simulink model "kinovaMicoSimscapeModel"  (R2021b)
(part 40 of 50)

Y4_5_3=(1369*ddqr5)/2000000 - (4107*ddqr4*cos(q5)^2)/4000000 + ddqr4*((23717*3^(1/2))/10000000 + 2327843/400000000) - (1369*dq2*dqr3*sin(2*q5))/4000000 + (1369*dq3*dqr3*sin(2*q5))/4000000 + (4107*dq4*dqr5*sin(2*q5))/8000000 + (4107*dq5*dqr4*sin(2*q5))/8000000 - (32449*ddqr2*sin(q4)*sin(q5))/4000000 + (32449*ddqr3*sin(q4)*sin(q5))/4000000 - ddqr4*cos(q5)*((23717*3^(1/2))/20000000 + 1369/1000000) - ddqr5*cos(q5)*((23717*3^(1/2))/20000000 + 1369/1000000) - ddqr2*cos(q4)*((562157*3^(1/2))/80000000 + 32449/4000000) + ddqr3*cos(q4)*((562157*3^(1/2))/80000000 + 32449/4000000) + (1369*3^(1/2)*ddqr2*cos(q4)*cos(q5)^2)/4000000 - (1369*3^(1/2)*ddqr3*cos(q4)*cos(q5)^2)/4000000 + dq2*dqr3*sin(q5)*((23717*3^(1/2))/20000000 + 1369/1000000) - dq3*dqr3*sin(q5)*((23717*3^(1/2))/20000000 + 1369/1000000) + dq5*dqr5*sin(q5)*((23717*3^(1/2))/20000000 + 1369/1000000) + dq4*dqr5*sin(q5)*((23717*3^(1/2))/40000000 + 1369/2000000) + dq5*dqr4*sin(q5)*((23717*3^(1/2))/40000000 + 1369/2000000) - (1073*ddqr2*cos(q3)*cos(q4)*cos(q5))/200000 - (1073*ddqr1*cos(q4)*sin(q2)*sin(q5))/100000 - (1073*ddqr1*cos(q5)*sin(q2)*sin(q4))/200000 + (1073*ddqr2*cos(q3)*sin(q4)*sin(q5))/100000 + (1369*3^(1/2)*dq2*dqr5*sin(q4))/2000000 - (1369*3^(1/2)*dq3*dqr5*sin(q4))/2000000 - (1369*3^(1/2)*dq5*dqr3*sin(q4))/2000000 + ddqr2*cos(q3)*cos(q4)*((18589*3^(1/2))/2000000 + 1073/100000) - ddqr2*cos(q4)*cos(q5)*((1369*3^(1/2))/2000000 - 45547/20000000) + ddqr3*cos(q4)*cos(q5)*((1369*3^(1/2))/2000000 - 45547/20000000) - (4107*ddqr1*cos(q2)*cos(q3)*cos(q5)^2)/4000000 + ddqr1*cos(q2)*cos(q3)*((23717*3^(1/2))/10000000 + 2327843/400000000) + ddqr1*sin(q2)*sin(q4)*((18589*3^(1/2))/2000000 + 1073/100000) + dq2*dqr3*sin(2*q4)*((23717*3^(1/2))/20000000 + 1232643/800000000) - dq3*dqr3*sin(2*q4)*((23717*3^(1/2))/20000000 + 1232643/800000000) - (4107*ddqr1*cos(q5)^2*sin(q2)*sin(q3))/4000000 + ddqr1*sin(q2)*sin(q3)*((23717*3^(1/2))/10000000 + 2327843/400000000) + dq2*dqr5*cos(q4)*sin(q5)*((1369*3^(1/2))/2000000 + 71151/40000000) - dq3*dqr5*cos(q4)*sin(q5)*((1369*3^(1/2))/2000000 + 71151/40000000) - dq5*dqr3*cos(q4)*sin(q5)*((1369*3^(1/2))/2000000 + 71151/40000000) + (1369*dq2*dqr3*cos(q4)*cos(q5)^2*sin(q4))/800000 + (1369*dq2*dqr3*cos(q4)^2*cos(q5)*sin(q5))/1000000 - (1369*dq3*dqr3*cos(q4)*cos(q5)^2*sin(q4))/800000 - (1369*dq3*dqr3*cos(q4)^2*cos(q5)*sin(q5))/1000000 + (259*ddqr1*cos(q2)*cos(q3)*cos(q4)*cos(q5))/2000000 - (259*ddqr1*cos(q2)*cos(q3)*sin(q4)*sin(q5))/1000000 - (32449*ddqr1*cos(q2)*cos(q4)*sin(q3)*sin(q5))/4000000 + (32449*ddqr1*cos(q3)*cos(q4)*sin(q2)*sin(q5))/4000000 + (259*ddqr1*cos(q4)*cos(q5)*sin(q2)*sin(q3))/2000000 - (259*ddqr1*sin(q2)*sin(q3)*sin(q4)*sin(q5))/1000000 - dq2*dqr3*cos(q4)^2*sin(q5)*((23717*3^(1/2))/10000000 + 1369/500000) + dq3*dqr3*cos(q4)^2*sin(q5)*((23717*3^(1/2))/10000000 + 1369/500000) - ddqr1*cos(q2)*cos(q3)*cos(q4)*((4487*3^(1/2))/20000000 + 259/1000000) - ddqr1*cos(q2)*cos(q3)*cos(q5)*((23717*3^(1/2))/20000000 + 1369/1000000) - ddqr1*cos(q4)*sin(q2)*sin(q3)*((4487*3^(1/2))/20000000 + 259/1000000) - ddqr1*cos(q5)*sin(q2)*sin(q3)*((23717*3^(1/2))/20000000 + 1369/1000000) + ddqr1*cos(q2)*sin(q3)*sin(q4)*((562157*3^(1/2))/80000000 + 32449/4000000) - ddqr1*cos(q3)*sin(q2)*sin(q4)*((562157*3^(1/2))/80000000 + 32449/4000000) - (1369*3^(1/2)*dq2*dqr5*cos(q5)^2*sin(q4))/2000000 + (1369*3^(1/2)*dq3*dqr5*cos(q5)^2*sin(q4))/2000000 + (1369*3^(1/2)*dq5*dqr3*cos(q5)^2*sin(q4))/2000000 - (1369*3^(1/2)*ddqr2*cos(q5)*sin(q4)*sin(q5))/2000000 + (1369*3^(1/2)*ddqr3*cos(q5)*sin(q4)*sin(q5))/2000000 + (1369*3^(1/2)*dq1*dqr5*cos(q2)*cos(q4)*sin(q3))/2000000 - (1369*3^(1/2)*dq1*dqr5*cos(q3)*cos(q4)*sin(q2))/2000000 - (1369*3^(1/2)*dq2*dqr5*cos(q4)*cos(q5)*sin(q5))/4000000 + (1369*3^(1/2)*dq3*dqr5*cos(q4)*cos(q5)*sin(q5))/4000000 + (1369*3^(1/2)*dq5*dqr3*cos(q4)*cos(q5)*sin(q5))/4000000 + ddqr1*cos(q2)*cos(q5)*sin(q3)*sin(q4)*((1369*3^(1/2))/2000000 - 45547/20000000) - ddqr1*cos(q3)*cos(q5)*sin(q2)*sin(q4)*((1369*3^(1/2))/2000000 - 45547/20000000) - (32449*dq1*dqr3*cos(q2)*cos(q3)*cos(q4)*sin(q5))/4000000 + (4107*dq1*dqr5*cos(q2)*cos(q3)*cos(q5)*sin(q5))/4000000 + (4107*dq1*dqr5*cos(q5)*sin(q2)*sin(q3)*sin(q5))/4000000 - dq2*dqr3*cos(q4)*cos(q5)*sin(q4)*((23717*3^(1/2))/20000000 + 1369/1000000) + dq3*dqr3*cos(q4)*cos(q5)*sin(q4)*((23717*3^(1/2))/20000000 + 1369/1000000) + dq1*dqr5*cos(q2)*cos(q3)*sin(q5)*((23717*3^(1/2))/40000000 + 1369/2000000) + dq1*dqr3*cos(q2)*cos(q3)*sin(q4)*((562157*3^(1/2))/80000000 + 32449/4000000) - (1369*3^(1/2)*ddqr1*cos(q2)*cos(q5)^2*sin(q3)*sin(q4))/4000000 + (1369*3^(1/2)*ddqr1*cos(q3)*cos(q5)^2*sin(q2)*sin(q4))/4000000 + dq1*dqr5*sin(q2)*sin(q3)*sin(q5)*((23717*3^(1/2))/40000000 + 1369/2000000) - (1369*3^(1/2)*dq1*dqr5*cos(q2)*cos(q4)*cos(q5)^2*sin(q3))/2000000 + (1369*3^(1/2)*dq1*dqr5*cos(q3)*cos(q4)*cos(q5)^2*sin(q2))/2000000 - (1369*3^(1/2)*ddqr1*cos(q2)*cos(q4)*cos(q5)*sin(q3)*sin(q5))/2000000 + (1369*3^(1/2)*ddqr1*cos(q3)*cos(q4)*cos(q5)*sin(q2)*sin(q5))/2000000 - dq1*dqr5*cos(q2)*sin(q3)*sin(q4)*sin(q5)*((1369*3^(1/2))/2000000 + 71151/40000000) + dq1*dqr5*cos(q3)*sin(q2)*sin(q4)*sin(q5)*((1369*3^(1/2))/2000000 + 71151/40000000) - (1369*3^(1/2)*dq1*dqr3*cos(q2)*cos(q3)*cos(q4)*cos(q5)*sin(q5))/2000000 + (1369*3^(1/2)*dq1*dqr5*cos(q2)*cos(q5)*sin(q3)*sin(q4)*sin(q5))/4000000 - (1369*3^(1/2)*dq1*dqr5*cos(q3)*cos(q5)*sin(q2)*sin(q4)*sin(q5))/4000000;
Y4_8_1=(1231*ddqr2*cos(q4))/10000 - (1231*ddqr3*cos(q4))/10000 + (7*dq1*dqr1*sin(q4))/1000 - (29*ddqr2*cos(q3)*cos(q4))/100 - (29*ddqr1*sin(q2)*sin(q4))/100 + (7*ddqr1*cos(q2)*cos(q3)*cos(q4))/1000 - (1231*ddqr1*cos(q2)*sin(q3)*sin(q4))/10000 + (1231*ddqr1*cos(q3)*sin(q2)*sin(q4))/10000 + (7*ddqr1*cos(q4)*sin(q2)*sin(q3))/1000 + (29*dq1*dqr1*cos(q4)*sin(q3))/100 - (29*dq1*dqr2*cos(q2)*sin(q4))/100 - (29*dq2*dqr1*cos(q2)*sin(q4))/100 + (29*dq2*dqr2*cos(q4)*sin(q3))/100 - (29*dq1*dqr1*cos(q2)^2*cos(q4)*sin(q3))/100 + (1231*dq1*dqr1*cos(q2)*cos(q4)*sin(q2))/10000 - (1231*dq1*dqr1*cos(q3)*cos(q4)*sin(q3))/10000 + (1231*dq1*dqr2*cos(q2)*cos(q3)*sin(q4))/10000 + (1231*dq2*dqr1*cos(q2)*cos(q3)*sin(q4))/10000 - (1231*dq1*dqr3*cos(q2)*cos(q3)*sin(q4))/10000 - (1231*dq3*dqr1*cos(q2)*cos(q3)*sin(q4))/10000 + (1231*dq1*dqr2*sin(q2)*sin(q3)*sin(q4))/10000 + (1231*dq2*dqr1*sin(q2)*sin(q3)*sin(q4))/10000 - (1231*dq1*dqr3*sin(q2)*sin(q3)*sin(q4))/10000 - (1231*dq3*dqr1*sin(q2)*sin(q3)*sin(q4))/10000 + (29*dq1*dqr1*cos(q2)*cos(q3)*cos(q4)*sin(q2))/100 - (1231*dq1*dqr1*cos(q2)*cos(q3)^2*cos(q4)*sin(q2))/5000 + (1231*dq1*dqr1*cos(q2)^2*cos(q3)*cos(q4)*sin(q3))/5000;
Y4_9_1=(37*dq2*dqr2*sin(q5))/1000 - (37*dq2*dqr3*sin(q5))/1000 - (37*dq3*dqr2*sin(q5))/1000 + (37*dq3*dqr3*sin(q5))/1000 - (37*dq4*dqr5*sin(q5))/2000 - (37*dq5*dqr4*sin(q5))/2000 - (37*dq1*dqr1*cos(q2)^2*sin(q5))/1000 - (37*dq1*dqr1*cos(q3)^2*sin(q5))/1000 - (37*dq2*dqr2*cos(q4)^2*sin(q5))/500 + (37*dq2*dqr3*cos(q4)^2*sin(q5))/500 + (37*dq3*dqr2*cos(q4)^2*sin(q5))/500 - (37*dq3*dqr3*cos(q4)^2*sin(q5))/500 - (7*dq1*dqr1*cos(q4)*sin(q5))/1000 - (7*dq1*dqr1*cos(q5)*sin(q4))/2000 - (37*3^(1/2)*dq2*dqr5*cos(q4)*sin(q5))/2000 - (37*3^(1/2)*dq5*dqr2*cos(q4)*sin(q5))/2000 + (37*3^(1/2)*dq3*dqr5*cos(q4)*sin(q5))/2000 + (37*3^(1/2)*dq5*dqr3*cos(q4)*sin(q5))/2000 + (37*dq1*dqr1*cos(q2)^2*cos(q3)^2*sin(q5))/500 + (37*dq1*dqr1*cos(q2)^2*cos(q4)^2*sin(q5))/500 + (37*dq1*dqr1*cos(q3)^2*cos(q4)^2*sin(q5))/500 + (37*dq1*dqr2*cos(q2)*cos(q5)*sin(q3))/1000 - (37*dq1*dqr2*cos(q3)*cos(q5)*sin(q2))/1000 + (37*dq2*dqr1*cos(q2)*cos(q5)*sin(q3))/1000 - (37*dq2*dqr1*cos(q3)*cos(q5)*sin(q2))/1000 - (29*dq1*dqr1*cos(q4)*cos(q5)*sin(q3))/200 + (29*dq1*dqr2*cos(q2)*cos(q4)*sin(q5))/100 + (29*dq1*dqr2*cos(q2)*cos(q5)*sin(q4))/200 - (37*dq1*dqr3*cos(q2)*cos(q5)*sin(q3))/1000 + (37*dq1*dqr3*cos(q3)*cos(q5)*sin(q2))/1000 + (29*dq2*dqr1*cos(q2)*cos(q4)*sin(q5))/100 + (29*dq2*dqr1*cos(q2)*cos(q5)*sin(q4))/200 - (37*dq3*dqr1*cos(q2)*cos(q5)*sin(q3))/1000 + (37*dq3*dqr1*cos(q3)*cos(q5)*sin(q2))/1000 - (37*dq1*dqr5*cos(q2)*cos(q3)*sin(q5))/2000 - (29*dq2*dqr2*cos(q4)*cos(q5)*sin(q3))/200 - (37*dq5*dqr1*cos(q2)*cos(q3)*sin(q5))/2000 - (37*dq2*dqr2*cos(q4)*cos(q5)*sin(q4))/1000 + (37*dq2*dqr3*cos(q4)*cos(q5)*sin(q4))/1000 + (37*dq3*dqr2*cos(q4)*cos(q5)*sin(q4))/1000 - (37*dq3*dqr3*cos(q4)*cos(q5)*sin(q4))/1000 + (29*dq1*dqr1*sin(q3)*sin(q4)*sin(q5))/100 - (37*dq1*dqr5*sin(q2)*sin(q3)*sin(q5))/2000 + (29*dq2*dqr2*sin(q3)*sin(q4)*sin(q5))/100 - (37*dq5*dqr1*sin(q2)*sin(q3)*sin(q5))/2000 - (29*dq1*dqr1*cos(q2)^2*sin(q3)*sin(q4)*sin(q5))/100 - (117*dq1*dqr2*cos(q2)*cos(q3)*cos(q4)*sin(q5))/625 - (117*dq2*dqr1*cos(q2)*cos(q3)*cos(q4)*sin(q5))/625 + (117*dq1*dqr3*cos(q2)*cos(q3)*cos(q4)*sin(q5))/625 + (117*dq3*dqr1*cos(q2)*cos(q3)*cos(q4)*sin(q5))/625 - (37*dq1*dqr1*cos(q2)^2*cos(q3)^2*cos(q4)^2*sin(q5))/250 + (117*dq1*dqr1*cos(q2)*sin(q2)*sin(q4)*sin(q5))/625 - (117*dq1*dqr1*cos(q3)*sin(q3)*sin(q4)*sin(q5))/625 - (117*dq1*dqr2*cos(q4)*sin(q2)*sin(q3)*sin(q5))/625 - (117*dq2*dqr1*cos(q4)*sin(q2)*sin(q3)*sin(q5))/625 + (117*dq1*dqr3*cos(q4)*sin(q2)*sin(q3)*sin(q5))/625 + (117*dq3*dqr1*cos(q4)*sin(q2)*sin(q3)*sin(q5))/625 + (29*dq1*dqr1*cos(q2)^2*cos(q4)*cos(q5)*sin(q3))/200 + (37*dq1*dqr1*cos(q2)^2*cos(q4)*cos(q5)*sin(q4))/1000 - (37*dq1*dqr2*cos(q2)*cos(q4)^2*cos(q5)*sin(q3))/1000 + (37*dq1*dqr2*cos(q3)*cos(q4)^2*cos(q5)*sin(q2))/1000 - (37*dq2*dqr1*cos(q2)*cos(q4)^2*cos(q5)*sin(q3))/1000 + (37*dq2*dqr1*cos(q3)*cos(q4)^2*cos(q5)*sin(q2))/1000 + (37*dq1*dqr1*cos(q3)^2*cos(q4)*cos(q5)*sin(q4))/1000 + (37*dq1*dqr3*cos(q2)*cos(q4)^2*cos(q5)*sin(q3))/1000 - (37*dq1*dqr3*cos(q3)*cos(q4)^2*cos(q5)*sin(q2))/1000 + (37*dq3*dqr1*cos(q2)*cos(q4)^2*cos(q5)*sin(q3))/1000 - (37*dq3*dqr1*cos(q3)*cos(q4)^2*cos(q5)*sin(q2))/1000 + (37*3^(1/2)*dq1*dqr5*cos(q2)*sin(q3)*sin(q4)*sin(q5))/2000 - (37*3^(1/2)*dq1*dqr5*cos(q3)*sin(q2)*sin(q4)*sin(q5))/2000 + (37*3^(1/2)*dq5*dqr1*cos(q2)*sin(q3)*sin(q4)*sin(q5))/2000 - (37*3^(1/2)*dq5*dqr1*cos(q3)*sin(q2)*sin(q4)*sin(q5))/2000 - (37*dq1*dqr1*cos(q2)^2*cos(q3)^2*cos(q4)*cos(q5)*sin(q4))/500 - (29*dq1*dqr1*cos(q2)*cos(q3)*cos(q4)*cos(q5)*sin(q2))/200 + (37*dq1*dqr1*cos(q2)*cos(q3)*sin(q2)*sin(q3)*sin(q5))/500 + (29*dq1*dqr1*cos(q2)*cos(q3)*sin(q2)*sin(q4)*sin(q5))/100 + (37*dq1*dqr2*cos(q2)*cos(q4)*sin(q3)*sin(q4)*sin(q5))/500 - (37*dq1*dqr2*cos(q3)*cos(q4)*sin(q2)*sin(q4)*sin(q5))/500 + (37*dq2*dqr1*cos(q2)*cos(q4)*sin(q3)*sin(q4)*sin(q5))/500 - (37*dq2*dqr1*cos(q3)*cos(q4)*sin(q2)*sin(q4)*sin(q5))/500 - (37*dq1*dqr3*cos(q2)*cos(q4)*sin(q3)*sin(q4)*sin(q5))/500 + (37*dq1*dqr3*cos(q3)*cos(q4)*sin(q2)*sin(q4)*sin(q5))/500 - (37*dq3*dqr1*cos(q2)*cos(q4)*sin(q3)*sin(q4)*sin(q5))/500 + (37*dq3*dqr1*cos(q3)*cos(q4)*sin(q2)*sin(q4)*sin(q5))/500 + dq1*dqr1*cos(q2)*cos(q4)*cos(q5)*sin(q2)*((37*3^(1/2))/2000 - 117/1250) - dq1*dqr1*cos(q3)*cos(q4)*cos(q5)*sin(q3)*((37*3^(1/2))/2000 - 117/1250) + dq1*dqr2*cos(q2)*cos(q3)*cos(q5)*sin(q4)*((37*3^(1/2))/2000 - 117/1250) + dq2*dqr1*cos(q2)*cos(q3)*cos(q5)*sin(q4)*((37*3^(1/2))/2000 - 117/1250) - dq1*dqr3*cos(q2)*cos(q3)*cos(q5)*sin(q4)*((37*3^(1/2))/2000 - 117/1250) - dq3*dqr1*cos(q2)*cos(q3)*cos(q5)*sin(q4)*((37*3^(1/2))/2000 - 117/1250) + dq1*dqr2*cos(q5)*sin(q2)*sin(q3)*sin(q4)*((37*3^(1/2))/2000 - 117/1250) + dq2*dqr1*cos(q5)*sin(q2)*sin(q3)*sin(q4)*((37*3^(1/2))/2000 - 117/1250) - dq1*dqr3*cos(q5)*sin(q2)*sin(q3)*sin(q4)*((37*3^(1/2))/2000 - 117/1250) - dq3*dqr1*cos(q5)*sin(q2)*sin(q3)*sin(q4)*((37*3^(1/2))/2000 - 117/1250) - (234*dq1*dqr1*cos(q2)*cos(q3)^2*sin(q2)*sin(q4)*sin(q5))/625 + (234*dq1*dqr1*cos(q2)^2*cos(q3)*sin(q3)*sin(q4)*sin(q5))/625 - (37*dq1*dqr1*cos(q2)*cos(q3)*cos(q4)^2*sin(q2)*sin(q3)*sin(q5))/250 - dq1*dqr1*cos(q2)*cos(q3)^2*cos(q4)*cos(q5)*sin(q2)*((37*3^(1/2))/1000 - 117/625) + dq1*dqr1*cos(q2)^2*cos(q3)*cos(q4)*cos(q5)*sin(q3)*((37*3^(1/2))/1000 - 117/625) - (37*dq1*dqr1*cos(q2)*cos(q3)*cos(q4)*cos(q5)*sin(q2)*sin(q3)*sin(q4))/500;
Y4_9_2=(37*ddqr4*cos(q5))/1000 + (37*ddqr5*cos(q5))/1000 - (37*dq5*dqr5*sin(q5))/1000 + (117*ddqr2*sin(q4)*sin(q5))/625 - (117*ddqr3*sin(q4)*sin(q5))/625 + (37*ddqr1*cos(q2)*cos(q3)*cos(q5))/1000 + (29*ddqr2*cos(q3)*cos(q4)*cos(q5))/200 + (37*ddqr1*cos(q5)*sin(q2)*sin(q3))/1000 + (29*ddqr1*cos(q4)*sin(q2)*sin(q5))/100 + (29*ddqr1*cos(q5)*sin(q2)*sin(q4))/200 - (29*ddqr2*cos(q3)*sin(q4)*sin(q5))/100 + ddqr2*cos(q4)*cos(q5)*((37*3^(1/2))/2000 - 117/1250) - ddqr3*cos(q4)*cos(q5)*((37*3^(1/2))/2000 - 117/1250) - (7*ddqr1*cos(q2)*cos(q3)*cos(q4)*cos(q5))/2000 + (7*ddqr1*cos(q2)*cos(q3)*sin(q4)*sin(q5))/1000 + (117*ddqr1*cos(q2)*cos(q4)*sin(q3)*sin(q5))/625 - (117*ddqr1*cos(q3)*cos(q4)*sin(q2)*sin(q5))/625 - (7*ddqr1*cos(q4)*cos(q5)*sin(q2)*sin(q3))/2000 + (7*ddqr1*sin(q2)*sin(q3)*sin(q4)*sin(q5))/1000 - ddqr1*cos(q2)*cos(q5)*sin(q3)*sin(q4)*((37*3^(1/2))/2000 - 117/1250) + ddqr1*cos(q3)*cos(q5)*sin(q2)*sin(q4)*((37*3^(1/2))/2000 - 117/1250);
Y4_10_1=(111*dq5*dqr1*cos(q5)^2*sin(q2)*sin(q3)*sin(q6))/2000 - (111*dq5*dqr1*sin(q2)*sin(q3)*sin(q6))/4000 + (111*dq6*dqr1*cos(q5)^2*sin(q2)*sin(q3)*sin(q6))/8000 + dq6*dqr1*sin(q2)*sin(q3)*sin(q6)*((1923*3^(1/2))/80000 + 37/4000) + (37*3^(1/2)*dq1*dqr1*cos(q2)*sin(q2)*sin(q4)*sin(q6))/2000 - (37*3^(1/2)*dq2*dqr1*cos(q4)*sin(q2)*sin(q3)*sin(q6))/2000 + (37*3^(1/2)*dq3*dqr1*cos(q4)*sin(q2)*sin(q3)*sin(q6))/2000 + (37*3^(1/2)*dq5*dqr1*cos(q3)*sin(q2)*sin(q4)*sin(q6))/4000 + (87*dq1*dqr1*cos(q2)*cos(q3)*cos(q4)*cos(q6)*sin(q2))/400 + (1231*dq1*dqr1*cos(q2)*cos(q4)*cos(q5)*cos(q6)*sin(q2))/40000 - (37*dq1*dqr1*cos(q2)*cos(q3)*sin(q2)*sin(q3)*sin(q6))/1000 - (877*dq1*dqr1*cos(q2)*cos(q5)*sin(q2)*sin(q4)*sin(q6))/4000 + (37*dq2*dqr1*cos(q3)*cos(q4)*sin(q2)*sin(q4)*sin(q6))/1000 + (877*dq2*dqr1*cos(q4)*cos(q5)*sin(q2)*sin(q3)*sin(q6))/4000 + (1231*dq2*dqr1*cos(q5)*cos(q6)*sin(q2)*sin(q3)*sin(q4))/40000 - (37*dq3*dqr1*cos(q3)*cos(q4)*sin(q2)*sin(q4)*sin(q6))/1000 + (37*dq2*dqr1*cos(q3)*cos(q5)*sin(q2)*sin(q5)*sin(q6))/2000 - (877*dq3*dqr1*cos(q4)*cos(q5)*sin(q2)*sin(q3)*sin(q6))/4000 - (1231*dq3*dqr1*cos(q5)*cos(q6)*sin(q2)*sin(q3)*sin(q4))/40000 - (37*dq3*dqr1*cos(q3)*cos(q5)*sin(q2)*sin(q5)*sin(q6))/2000 + (111*dq5*dqr1*cos(q5)*cos(q6)*sin(q2)*sin(q3)*sin(q5))/4000 + (111*dq6*dqr1*cos(q5)*cos(q6)*sin(q2)*sin(q3)*sin(q5))/4000 - dq2*dqr1*cos(q3)*sin(q2)*sin(q5)*sin(q6)*((641*3^(1/2))/20000 + 37/1000) + dq3*dqr1*cos(q3)*sin(q2)*sin(q5)*sin(q6)*((641*3^(1/2))/20000 + 37/1000) + dq5*dqr1*cos(q5)*sin(q2)*sin(q3)*sin(q6)*((641*3^(1/2))/40000 + 37/2000) + dq6*dqr1*cos(q6)*sin(q2)*sin(q3)*sin(q5)*((641*3^(1/2))/40000 + 37/2000) + dq2*dqr1*cos(q6)*sin(q2)*sin(q3)*sin(q4)*((37*3^(1/2))/4000 + 7539/40000) - dq3*dqr1*cos(q6)*sin(q2)*sin(q3)*sin(q4)*((37*3^(1/2))/4000 + 7539/40000) - dq6*dqr1*cos(q3)*sin(q2)*sin(q4)*sin(q6)*((37*3^(1/2))/4000 + 1923/80000) + dq5*dqr1*cos(q6)*sin(q2)*sin(q3)*sin(q5)*((641*3^(1/2))/80000 - 37/8000) + dq6*dqr1*cos(q5)*sin(q2)*sin(q3)*sin(q6)*((641*3^(1/2))/80000 - 37/8000) + (37*3^(1/2)*dq1*dqr1*cos(q2)*cos(q4)*cos(q5)^2*cos(q6)*sin(q2))/4000 + (29*dq1*dqr1*cos(q2)*cos(q3)*cos(q4)*cos(q5)*cos(q6)*sin(q2))/400 - (37*3^(1/2)*dq1*dqr1*cos(q2)*cos(q3)^2*sin(q2)*sin(q4)*sin(q6))/1000 - (37*3^(1/2)*dq1*dqr1*cos(q2)*cos(q5)^2*sin(q2)*sin(q4)*sin(q6))/1000 + (37*3^(1/2)*dq2*dqr1*cos(q4)*cos(q5)^2*sin(q2)*sin(q3)*sin(q6))/1000 + (37*3^(1/2)*dq2*dqr1*cos(q5)^2*cos(q6)*sin(q2)*sin(q3)*sin(q4))/4000 - (37*3^(1/2)*dq3*dqr1*cos(q4)*cos(q5)^2*sin(q2)*sin(q3)*sin(q6))/1000 - (37*3^(1/2)*dq3*dqr1*cos(q5)^2*cos(q6)*sin(q2)*sin(q3)*sin(q4))/4000 - (37*3^(1/2)*dq5*dqr1*cos(q3)*cos(q5)^2*sin(q2)*sin(q4)*sin(q6))/2000 - (37*3^(1/2)*dq6*dqr1*cos(q3)*cos(q5)^2*sin(q2)*sin(q4)*sin(q6))/8000 - (29*dq1*dqr1*cos(q2)*cos(q3)*cos(q4)*sin(q2)*sin(q5)*sin(q6))/200 - (29*dq1*dqr1*cos(q2)*cos(q3)*cos(q5)*sin(q2)*sin(q4)*sin(q6))/100 - (29*dq1*dqr1*cos(q2)*cos(q3)*cos(q6)*sin(q2)*sin(q4)*sin(q5))/200 - (1231*dq1*dqr1*cos(q2)*cos(q3)^2*cos(q4)*cos(q5)*cos(q6)*sin(q2))/20000 + dq1*dqr1*cos(q2)*cos(q6)*sin(q2)*sin(q4)*sin(q5)*((37*3^(1/2))/4000 - 877/8000) - dq2*dqr1*cos(q4)*cos(q6)*sin(q2)*sin(q3)*sin(q5)*((37*3^(1/2))/4000 - 877/8000) + dq3*dqr1*cos(q4)*cos(q6)*sin(q2)*sin(q3)*sin(q5)*((37*3^(1/2))/4000 - 877/8000) + dq1*dqr1*cos(q2)*cos(q4)*sin(q2)*sin(q5)*sin(q6)*((37*3^(1/2))/2000 - 1231/20000) + dq5*dqr1*cos(q3)*cos(q5)*sin(q2)*sin(q4)*sin(q6)*((37*3^(1/2))/2000 + 1923/40000) + dq6*dqr1*cos(q3)*cos(q6)*sin(q2)*sin(q4)*sin(q5)*((37*3^(1/2))/2000 + 1923/40000) - dq5*dqr1*cos(q3)*cos(q6)*sin(q2)*sin(q4)*sin(q5)*((37*3^(1/2))/8000 - 1923/80000) + dq6*dqr1*cos(q3)*cos(q5)*sin(q2)*sin(q4)*sin(q6)*((111*3^(1/2))/8000 + 1923/80000) + (37*dq1*dqr1*cos(q2)*cos(q3)*cos(q4)^2*sin(q2)*sin(q3)*sin(q6))/500 + (37*dq1*dqr1*cos(q2)*cos(q3)*cos(q5)^2*sin(q2)*sin(q3)*sin(q6))/500 + (877*dq1*dqr1*cos(q2)*cos(q3)^2*cos(q5)*sin(q2)*sin(q4)*sin(q6))/2000 - (37*dq2*dqr1*cos(q3)*cos(q4)*cos(q5)^2*sin(q2)*sin(q4)*sin(q6))/500 - (37*dq2*dqr1*cos(q3)*cos(q4)^2*cos(q5)*sin(q2)*sin(q5)*sin(q6))/400 + (37*dq3*dqr1*cos(q3)*cos(q4)*cos(q5)^2*sin(q2)*sin(q4)*sin(q6))/500 + (37*dq3*dqr1*cos(q3)*cos(q4)^2*cos(q5)*sin(q2)*sin(q5)*sin(q6))/400 + dq2*dqr1*sin(q2)*sin(q3)*sin(q4)*sin(q5)*sin(q6)*((37*3^(1/2))/2000 - 1231/20000) - dq3*dqr1*sin(q2)*sin(q3)*sin(q4)*sin(q5)*sin(q6)*((37*3^(1/2))/2000 - 1231/20000) - dq1*dqr1*cos(q2)*cos(q3)^2*cos(q4)*cos(q6)*sin(q2)*((37*3^(1/2))/2000 + 7539/20000) + (37*3^(1/2)*dq6*dqr1*cos(q3)*cos(q4)*sin(q2)*sin(q5)*sin(q6))/4000 + dq2*dqr1*cos(q3)*cos(q4)^2*sin(q2)*sin(q5)*sin(q6)*((641*3^(1/2))/20000 + 37/1000) - dq3*dqr1*cos(q3)*cos(q4)^2*sin(q2)*sin(q5)*sin(q6)*((641*3^(1/2))/20000 + 37/1000) + (37*dq1*dqr1*cos(q2)*cos(q3)*cos(q5)*cos(q6)*sin(q2)*sin(q3)*sin(q5))/1000 - (37*dq2*dqr1*cos(q3)*cos(q4)*cos(q5)*cos(q6)*sin(q2)*sin(q4)*sin(q5))/1000 + (37*dq3*dqr1*cos(q3)*cos(q4)*cos(q5)*cos(q6)*sin(q2)*sin(q4)*sin(q5))/1000 - (37*3^(1/2)*dq1*dqr1*cos(q2)*cos(q3)^2*cos(q4)*cos(q5)^2*cos(q6)*sin(q2))/2000 - dq1*dqr1*cos(q2)*cos(q3)*cos(q5)*sin(q2)*sin(q3)*sin(q6)*((641*3^(1/2))/10000 + 37/500) + dq2*dqr1*cos(q3)*cos(q4)*cos(q5)*sin(q2)*sin(q4)*sin(q6)*((641*3^(1/2))/10000 + 37/500) - dq3*dqr1*cos(q3)*cos(q4)*cos(q5)*sin(q2)*sin(q4)*sin(q6)*((641*3^(1/2))/10000 + 37/500) - dq1*dqr1*cos(q2)*cos(q3)*cos(q6)*sin(q2)*sin(q3)*sin(q5)*((641*3^(1/2))/20000 - 37/2000) + dq2*dqr1*cos(q3)*cos(q4)*cos(q6)*sin(q2)*sin(q4)*sin(q5)*((641*3^(1/2))/20000 - 37/2000) - dq3*dqr1*cos(q3)*cos(q4)*cos(q6)*sin(q2)*sin(q4)*sin(q5)*((641*3^(1/2))/20000 - 37/2000) + (37*3^(1/2)*dq1*dqr1*cos(q2)*cos(q3)^2*cos(q5)^2*sin(q2)*sin(q4)*sin(q6))/500 - (37*3^(1/2)*dq1*dqr1*cos(q2)*cos(q4)*cos(q5)*sin(q2)*sin(q5)*sin(q6))/2000 - (37*3^(1/2)*dq1*dqr1*cos(q2)*cos(q5)*cos(q6)*sin(q2)*sin(q4)*sin(q5))/2000 + (37*3^(1/2)*dq2*dqr1*cos(q4)*cos(q5)*cos(q6)*sin(q2)*sin(q3)*sin(q5))/2000 - (37*3^(1/2)*dq3*dqr1*cos(q4)*cos(q5)*cos(q6)*sin(q2)*sin(q3)*sin(q5))/2000 - (37*3^(1/2)*dq5*dqr1*cos(q3)*cos(q4)*cos(q5)*sin(q2)*sin(q5)*sin(q6))/1000 - (37*3^(1/2)*dq5*dqr1*cos(q3)*cos(q5)*cos(q6)*sin(q2)*sin(q4)*sin(q5))/4000 - (37*3^(1/2)*dq6*dqr1*cos(q3)*cos(q4)*cos(q5)*sin(q2)*sin(q5)*sin(q6))/4000 - (37*3^(1/2)*dq6*dqr1*cos(q3)*cos(q5)*cos(q6)*sin(q2)*sin(q4)*sin(q5))/4000 - dq1*dqr1*cos(q2)*cos(q3)^2*cos(q6)*sin(q2)*sin(q4)*sin(q5)*((37*3^(1/2))/2000 - 877/4000) - dq1*dqr1*cos(q2)*cos(q3)^2*cos(q4)*sin(q2)*sin(q5)*sin(q6)*((37*3^(1/2))/1000 - 1231/10000) - (37*3^(1/2)*dq2*dqr1*cos(q5)*sin(q2)*sin(q3)*sin(q4)*sin(q5)*sin(q6))/2000 + (37*3^(1/2)*dq3*dqr1*cos(q5)*sin(q2)*sin(q3)*sin(q4)*sin(q5)*sin(q6))/2000 - (37*dq1*dqr1*cos(q2)*cos(q3)*cos(q4)^2*cos(q5)^2*sin(q2)*sin(q3)*sin(q6))/250 + dq1*dqr1*cos(q2)*cos(q3)*cos(q4)*cos(q6)*sin(q2)*sin(q3)*sin(q4)*((1923*3^(1/2))/20000 + 37/200) - (37*dq1*dqr1*cos(q2)*cos(q3)*cos(q4)*cos(q5)^2*cos(q6)*sin(q2)*sin(q3)*sin(q4))/400 - (37*dq1*dqr1*cos(q2)*cos(q3)*cos(q4)^2*cos(q5)*cos(q6)*sin(q2)*sin(q3)*sin(q5))/500 + dq1*dqr1*cos(q2)*cos(q3)*cos(q4)^2*cos(q5)*sin(q2)*sin(q3)*sin(q6)*((641*3^(1/2))/5000 + 37/250) + dq1*dqr1*cos(q2)*cos(q3)*cos(q4)^2*cos(q6)*sin(q2)*sin(q3)*sin(q5)*((641*3^(1/2))/10000 - 37/1000) + (37*3^(1/2)*dq1*dqr1*cos(q2)*cos(q3)^2*cos(q4)*cos(q5)*sin(q2)*sin(q5)*sin(q6))/1000 + (37*3^(1/2)*dq1*dqr1*cos(q2)*cos(q3)^2*cos(q5)*cos(q6)*sin(q2)*sin(q4)*sin(q5))/1000 + dq1*dqr1*cos(q2)*cos(q3)*cos(q4)*cos(q5)*cos(q6)*sin(q2)*sin(q3)*sin(q4)*((641*3^(1/2))/20000 - 37/2000) - dq1*dqr1*cos(q2)*cos(q3)*cos(q4)*sin(q2)*sin(q3)*sin(q4)*sin(q5)*sin(q6)*((641*3^(1/2))/10000 + 37/500) + (37*dq1*dqr1*cos(q2)*cos(q3)*cos(q4)*cos(q5)*sin(q2)*sin(q3)*sin(q4)*sin(q5)*sin(q6))/200;
Y4_10_2=(87*dq1*dqr1*cos(q4)*cos(q6)*sin(q3))/400 + (29*dq1*dqr1*cos(q4)*cos(q5)*cos(q6)*sin(q3))/400 - (29*dq1*dqr1*cos(q4)*sin(q3)*sin(q5)*sin(q6))/200 - (29*dq1*dqr1*cos(q5)*sin(q3)*sin(q4)*sin(q6))/100 - (29*dq1*dqr1*cos(q6)*sin(q3)*sin(q4)*sin(q5))/200 - dq2*dqr1*cos(q2)*cos(q6)*sin(q3)*((1923*3^(1/2))/40000 + 111/2000) + dq2*dqr1*cos(q3)*cos(q6)*sin(q2)*((1923*3^(1/2))/40000 + 111/2000) + dq3*dqr1*cos(q2)*cos(q6)*sin(q3)*((1923*3^(1/2))/40000 + 111/2000) - dq3*dqr1*cos(q3)*cos(q6)*sin(q2)*((1923*3^(1/2))/40000 + 111/2000) - (87*dq1*dqr1*cos(q2)^2*cos(q4)*cos(q6)*sin(q3))/400 + (37*dq2*dqr1*cos(q2)*cos(q5)^2*cos(q6)*sin(q3))/4000 - (37*dq2*dqr1*cos(q3)*cos(q5)^2*cos(q6)*sin(q2))/4000 - (37*dq3*dqr1*cos(q2)*cos(q5)^2*cos(q6)*sin(q3))/4000 + (37*dq3*dqr1*cos(q3)*cos(q5)^2*cos(q6)*sin(q2))/4000 + dq2*dqr1*cos(q2)*cos(q4)^2*cos(q6)*sin(q3)*((1923*3^(1/2))/40000 + 37/400) - dq2*dqr1*cos(q3)*cos(q4)^2*cos(q6)*sin(q2)*((1923*3^(1/2))/40000 + 37/400) - dq3*dqr1*cos(q2)*cos(q4)^2*cos(q6)*sin(q3)*((1923*3^(1/2))/40000 + 37/400) + dq3*dqr1*cos(q3)*cos(q4)^2*cos(q6)*sin(q2)*((1923*3^(1/2))/40000 + 37/400) - (37*3^(1/2)*dq1*dqr1*cos(q3)*sin(q3)*sin(q4)*sin(q6))/2000 - (37*3^(1/2)*dq5*dqr1*cos(q2)*sin(q3)*sin(q4)*sin(q6))/4000 - (37*dq2*dqr1*cos(q2)*cos(q4)^2*cos(q5)^2*cos(q6)*sin(q3))/800 + (37*dq2*dqr1*cos(q3)*cos(q4)^2*cos(q5)^2*cos(q6)*sin(q2))/800 + (37*dq3*dqr1*cos(q2)*cos(q4)^2*cos(q5)^2*cos(q6)*sin(q3))/800 - (37*dq3*dqr1*cos(q3)*cos(q4)^2*cos(q5)^2*cos(q6)*sin(q2))/800 - (1231*dq1*dqr1*cos(q3)*cos(q4)*cos(q5)*cos(q6)*sin(q3))/40000 - (37*dq2*dqr1*cos(q2)*cos(q4)*sin(q3)*sin(q4)*sin(q6))/1000 + (877*dq1*dqr1*cos(q3)*cos(q5)*sin(q3)*sin(q4)*sin(q6))/4000 + (37*dq3*dqr1*cos(q2)*cos(q4)*sin(q3)*sin(q4)*sin(q6))/1000 - (37*dq2*dqr1*cos(q2)*cos(q5)*sin(q3)*sin(q5)*sin(q6))/2000 + (37*dq3*dqr1*cos(q2)*cos(q5)*sin(q3)*sin(q5)*sin(q6))/2000 - dq2*dqr1*cos(q2)*cos(q5)*cos(q6)*sin(q3)*((641*3^(1/2))/40000 - 37/4000) + dq2*dqr1*cos(q3)*cos(q5)*cos(q6)*sin(q2)*((641*3^(1/2))/40000 - 37/4000) + dq3*dqr1*cos(q2)*cos(q5)*cos(q6)*sin(q3)*((641*3^(1/2))/40000 - 37/4000) - dq3*dqr1*cos(q3)*cos(q5)*cos(q6)*sin(q2)*((641*3^(1/2))/40000 - 37/4000) + dq1*dqr1*cos(q2)*cos(q4)*cos(q6)*sin(q2)*((37*3^(1/2))/4000 + 7539/40000) - dq1*dqr1*cos(q3)*cos(q4)*cos(q6)*sin(q3)*((37*3^(1/2))/4000 + 7539/40000) - (29*dq1*dqr1*cos(q2)^2*cos(q4)*cos(q5)*cos(q6)*sin(q3))/400 + dq2*dqr1*cos(q2)*sin(q3)*sin(q5)*sin(q6)*((641*3^(1/2))/20000 + 37/1000) - dq3*dqr1*cos(q2)*sin(q3)*sin(q5)*sin(q6)*((641*3^(1/2))/20000 + 37/1000) + dq6*dqr1*cos(q2)*sin(q3)*sin(q4)*sin(q6)*((37*3^(1/2))/4000 + 1923/80000) + (29*dq1*dqr1*cos(q2)^2*cos(q4)*sin(q3)*sin(q5)*sin(q6))/200 + (29*dq1*dqr1*cos(q2)^2*cos(q5)*sin(q3)*sin(q4)*sin(q6))/100 + (29*dq1*dqr1*cos(q2)^2*cos(q6)*sin(q3)*sin(q4)*sin(q5))/200 + (37*3^(1/2)*dq5*dqr1*cos(q2)*cos(q4)*cos(q6)*sin(q3))/2000 - (37*3^(1/2)*dq5*dqr1*cos(q3)*cos(q4)*cos(q6)*sin(q2))/2000 + (37*3^(1/2)*dq6*dqr1*cos(q2)*cos(q4)*cos(q6)*sin(q3))/2000 - (37*3^(1/2)*dq6*dqr1*cos(q3)*cos(q4)*cos(q6)*sin(q2))/2000 - (37*3^(1/2)*dq1*dqr1*cos(q3)*cos(q4)*cos(q5)^2*cos(q6)*sin(q3))/4000 - (37*3^(1/2)*dq5*dqr1*cos(q2)*cos(q4)*cos(q5)^2*cos(q6)*sin(q3))/2000 + (37*3^(1/2)*dq5*dqr1*cos(q3)*cos(q4)*cos(q5)^2*cos(q6)*sin(q2))/2000 - (37*3^(1/2)*dq6*dqr1*cos(q2)*cos(q4)*cos(q5)^2*cos(q6)*sin(q3))/2000 + (37*3^(1/2)*dq6*dqr1*cos(q3)*cos(q4)*cos(q5)^2*cos(q6)*sin(q2))/2000 + (37*3^(1/2)*dq1*dqr1*cos(q2)^2*cos(q3)*sin(q3)*sin(q4)*sin(q6))/1000 + (37*3^(1/2)*dq1*dqr1*cos(q3)*cos(q5)^2*sin(q3)*sin(q4)*sin(q6))/1000 + (37*3^(1/2)*dq5*dqr1*cos(q2)*cos(q5)^2*sin(q3)*sin(q4)*sin(q6))/2000 + (37*3^(1/2)*dq6*dqr1*cos(q2)*cos(q5)^2*sin(q3)*sin(q4)*sin(q6))/8000 + (1231*dq1*dqr1*cos(q2)^2*cos(q3)*cos(q4)*cos(q5)*cos(q6)*sin(q3))/20000 - dq1*dqr1*cos(q3)*cos(q6)*sin(q3)*sin(q4)*sin(q5)*((37*3^(1/2))/4000 - 877/8000) - dq1*dqr1*cos(q3)*cos(q4)*sin(q3)*sin(q5)*sin(q6)*((37*3^(1/2))/2000 - 1231/20000) - dq5*dqr1*cos(q2)*cos(q5)*sin(q3)*sin(q4)*sin(q6)*((37*3^(1/2))/2000 + 1923/40000) - dq6*dqr1*cos(q2)*cos(q6)*sin(q3)*sin(q4)*sin(q5)*((37*3^(1/2))/2000 + 1923/40000) + dq5*dqr1*cos(q2)*cos(q6)*sin(q3)*sin(q4)*sin(q5)*((37*3^(1/2))/8000 - 1923/80000) - dq6*dqr1*cos(q2)*cos(q5)*sin(q3)*sin(q4)*sin(q6)*((111*3^(1/2))/8000 + 1923/80000) - (877*dq1*dqr1*cos(q2)^2*cos(q3)*cos(q5)*sin(q3)*sin(q4)*sin(q6))/2000 + (37*dq2*dqr1*cos(q2)*cos(q4)*cos(q5)^2*sin(q3)*sin(q4)*sin(q6))/500 - (37*dq1*dqr1*cos(q2)^2*cos(q4)*cos(q5)*sin(q4)*sin(q5)*sin(q6))/400 + (37*dq2*dqr1*cos(q2)*cos(q4)^2*cos(q5)*sin(q3)*sin(q5)*sin(q6))/400 - (37*dq3*dqr1*cos(q2)*cos(q4)*cos(q5)^2*sin(q3)*sin(q4)*sin(q6))/500 - (37*dq3*dqr1*cos(q2)*cos(q4)^2*cos(q5)*sin(q3)*sin(q5)*sin(q6))/400 + dq1*dqr1*cos(q2)^2*cos(q3)*cos(q4)*cos(q6)*sin(q3)*((37*3^(1/2))/2000 + 7539/20000) + dq2*dqr1*cos(q2)*cos(q4)^2*cos(q5)*cos(q6)*sin(q3)*((641*3^(1/2))/40000 - 37/4000) - dq2*dqr1*cos(q3)*cos(q4)^2*cos(q5)*cos(q6)*sin(q2)*((641*3^(1/2))/40000 - 37/4000) - dq3*dqr1*cos(q2)*cos(q4)^2*cos(q5)*cos(q6)*sin(q3)*((641*3^(1/2))/40000 - 37/4000) + dq3*dqr1*cos(q3)*cos(q4)^2*cos(q5)*cos(q6)*sin(q2)*((641*3^(1/2))/40000 - 37/4000) - (37*3^(1/2)*dq6*dqr1*cos(q2)*cos(q4)*sin(q3)*sin(q5)*sin(q6))/4000 + dq1*dqr1*cos(q2)^2*cos(q4)*sin(q4)*sin(q5)*sin(q6)*((641*3^(1/2))/20000 + 37/1000) - dq2*dqr1*cos(q2)*cos(q4)^2*sin(q3)*sin(q5)*sin(q6)*((641*3^(1/2))/20000 + 37/1000) + dq3*dqr1*cos(q2)*cos(q4)^2*sin(q3)*sin(q5)*sin(q6)*((641*3^(1/2))/20000 + 37/1000) + (37*dq2*dqr1*cos(q2)*cos(q4)*cos(q5)*cos(q6)*sin(q3)*sin(q4)*sin(q5))/1000 - (37*dq3*dqr1*cos(q2)*cos(q4)*cos(q5)*cos(q6)*sin(q3)*sin(q4)*sin(q5))/1000 - dq1*dqr1*cos(q2)^2*cos(q3)^2*cos(q4)*sin(q4)*sin(q5)*sin(q6)*((641*3^(1/2))/10000 + 37/500) + (37*3^(1/2)*dq1*dqr1*cos(q2)^2*cos(q3)*cos(q4)*cos(q5)^2*cos(q6)*sin(q3))/2000 - dq2*dqr1*cos(q2)*cos(q4)*cos(q5)*sin(q3)*sin(q4)*sin(q6)*((641*3^(1/2))/10000 + 37/500) + dq3*dqr1*cos(q2)*cos(q4)*cos(q5)*sin(q3)*sin(q4)*sin(q6)*((641*3^(1/2))/10000 + 37/500) - dq2*dqr1*cos(q2)*cos(q4)*cos(q6)*sin(q3)*sin(q4)*sin(q5)*((641*3^(1/2))/20000 - 37/2000) + dq3*dqr1*cos(q2)*cos(q4)*cos(q6)*sin(q3)*sin(q4)*sin(q5)*((641*3^(1/2))/20000 - 37/2000) - (37*3^(1/2)*dq1*dqr1*cos(q2)^2*cos(q3)*cos(q5)^2*sin(q3)*sin(q4)*sin(q6))/500 + (37*3^(1/2)*dq1*dqr1*cos(q3)*cos(q4)*cos(q5)*sin(q3)*sin(q5)*sin(q6))/2000 + (37*3^(1/2)*dq1*dqr1*cos(q3)*cos(q5)*cos(q6)*sin(q3)*sin(q4)*sin(q5))/2000 - (37*3^(1/2)*dq2*dqr1*cos(q2)*cos(q3)*cos(q5)*sin(q4)*sin(q5)*sin(q6))/2000 + (37*3^(1/2)*dq3*dqr1*cos(q2)*cos(q3)*cos(q5)*sin(q4)*sin(q5)*sin(q6))/2000 + (37*3^(1/2)*dq5*dqr1*cos(q2)*cos(q4)*cos(q5)*sin(q3)*sin(q5)*sin(q6))/1000 + (37*3^(1/2)*dq5*dqr1*cos(q2)*cos(q5)*cos(q6)*sin(q3)*sin(q4)*sin(q5))/4000 + (37*3^(1/2)*dq6*dqr1*cos(q2)*cos(q4)*cos(q5)*sin(q3)*sin(q5)*sin(q6))/4000 + (37*3^(1/2)*dq6*dqr1*cos(q2)*cos(q5)*cos(q6)*sin(q3)*sin(q4)*sin(q5))/4000 + dq1*dqr1*cos(q2)^2*cos(q3)*cos(q6)*sin(q3)*sin(q4)*sin(q5)*((37*3^(1/2))/2000 - 877/4000) + dq1*dqr1*cos(q2)^2*cos(q3)*cos(q4)*sin(q3)*sin(q5)*sin(q6)*((37*3^(1/2))/1000 - 1231/10000) + (37*dq1*dqr1*cos(q2)^2*cos(q3)^2*cos(q4)*cos(q5)*sin(q4)*sin(q5)*sin(q6))/200 - (37*3^(1/2)*dq1*dqr1*cos(q2)^2*cos(q3)*cos(q4)*cos(q5)*sin(q3)*sin(q5)*sin(q6))/1000 - (37*3^(1/2)*dq1*dqr1*cos(q2)^2*cos(q3)*cos(q5)*cos(q6)*sin(q3)*sin(q4)*sin(q5))/1000;
Y4_10_3=(37*dq1*dqr1*cos(q2)^2*sin(q6))/2000 + (37*dq1*dqr1*cos(q3)^2*sin(q6))/2000 + (21*dq1*dqr1*cos(q6)*sin(q4))/4000 - (37*dq1*dqr1*cos(q2)^2*cos(q3)^2*sin(q6))/1000 - (37*dq1*dqr1*cos(q2)^2*cos(q4)^2*sin(q6))/1000 - (37*dq1*dqr1*cos(q2)^2*cos(q5)^2*sin(q6))/1000 - (37*dq1*dqr1*cos(q3)^2*cos(q4)^2*sin(q6))/1000 - (37*dq1*dqr1*cos(q3)^2*cos(q5)^2*sin(q6))/1000 - (87*dq2*dqr1*cos(q2)*cos(q6)*sin(q4))/400 + (7*dq1*dqr1*cos(q4)*cos(q5)*sin(q6))/1000 + (7*dq1*dqr1*cos(q4)*cos(q6)*sin(q5))/2000 + (7*dq1*dqr1*cos(q5)*cos(q6)*sin(q4))/4000 - (111*dq5*dqr1*cos(q2)*cos(q3)*sin(q6))/4000 - (7*dq1*dqr1*sin(q4)*sin(q5)*sin(q6))/2000 + dq1*dqr1*cos(q2)^2*cos(q5)*sin(q6)*((641*3^(1/2))/20000 + 37/1000) + dq1*dqr1*cos(q3)^2*cos(q5)*sin(q6)*((641*3^(1/2))/20000 + 37/1000) + dq1*dqr1*cos(q2)^2*cos(q6)*sin(q5)*((641*3^(1/2))/40000 - 37/4000) + dq1*dqr1*cos(q3)^2*cos(q6)*sin(q5)*((641*3^(1/2))/40000 - 37/4000) - (29*dq2*dqr1*cos(q2)*cos(q4)*cos(q5)*sin(q6))/100 - (29*dq2*dqr1*cos(q2)*cos(q4)*cos(q6)*sin(q5))/200 - (29*dq2*dqr1*cos(q2)*cos(q5)*cos(q6)*sin(q4))/400 + (37*dq1*dqr1*cos(q2)^2*cos(q3)^2*cos(q4)^2*sin(q6))/500 + (37*dq1*dqr1*cos(q2)^2*cos(q3)^2*cos(q5)^2*sin(q6))/500 + (37*dq1*dqr1*cos(q2)^2*cos(q4)^2*cos(q5)^2*sin(q6))/500 + (37*dq1*dqr1*cos(q3)^2*cos(q4)^2*cos(q5)^2*sin(q6))/500 + (29*dq2*dqr1*cos(q2)*sin(q4)*sin(q5)*sin(q6))/200 + dq6*dqr1*cos(q2)*cos(q3)*sin(q6)*((1923*3^(1/2))/80000 + 37/4000) - (37*dq1*dqr1*cos(q2)^2*cos(q5)*cos(q6)*sin(q5))/2000 - (37*dq1*dqr1*cos(q3)^2*cos(q5)*cos(q6)*sin(q5))/2000 + (111*dq5*dqr1*cos(q2)*cos(q3)*cos(q5)^2*sin(q6))/2000 + (111*dq6*dqr1*cos(q2)*cos(q3)*cos(q5)^2*sin(q6))/8000 - dq1*dqr1*cos(q2)^2*cos(q4)*cos(q6)*sin(q4)*((1923*3^(1/2))/40000 + 37/400) - dq1*dqr1*cos(q3)^2*cos(q4)*cos(q6)*sin(q4)*((1923*3^(1/2))/40000 + 37/400) - (37*3^(1/2)*dq1*dqr2*cos(q4)*sin(q2)*sin(q3)*sin(q6))/2000 + (37*dq1*dqr1*cos(q2)^2*cos(q4)*cos(q5)^2*cos(q6)*sin(q4))/800 + (37*dq1*dqr1*cos(q2)^2*cos(q3)^2*cos(q5)*cos(q6)*sin(q5))/1000 + (37*dq1*dqr2*cos(q3)*cos(q4)^2*cos(q5)^2*cos(q6)*sin(q2))/800 + (37*dq1*dqr1*cos(q2)^2*cos(q4)^2*cos(q5)*cos(q6)*sin(q5))/1000 + (37*dq1*dqr1*cos(q3)^2*cos(q4)*cos(q5)^2*cos(q6)*sin(q4))/800 + (37*dq1*dqr1*cos(q3)^2*cos(q4)^2*cos(q5)*cos(q6)*sin(q5))/1000 + (877*dq2*dqr1*cos(q2)*cos(q3)*cos(q4)*cos(q5)*sin(q6))/4000 + (1231*dq2*dqr1*cos(q2)*cos(q3)*cos(q5)*cos(q6)*sin(q4))/40000 - (877*dq3*dqr1*cos(q2)*cos(q3)*cos(q4)*cos(q5)*sin(q6))/4000 - (1231*dq3*dqr1*cos(q2)*cos(q3)*cos(q5)*cos(q6)*sin(q4))/40000 + (111*dq5*dqr1*cos(q2)*cos(q3)*cos(q5)*cos(q6)*sin(q5))/4000 + (111*dq6*dqr1*cos(q2)*cos(q3)*cos(q5)*cos(q6)*sin(q5))/4000 - dq1*dqr1*cos(q2)^2*cos(q3)^2*cos(q5)*sin(q6)*((641*3^(1/2))/10000 + 37/500) - dq1*dqr1*cos(q2)^2*cos(q4)^2*cos(q5)*sin(q6)*((641*3^(1/2))/10000 + 37/500) - dq1*dqr1*cos(q3)^2*cos(q4)^2*cos(q5)*sin(q6)*((641*3^(1/2))/10000 + 37/500) - dq1*dqr1*cos(q2)^2*cos(q3)^2*cos(q6)*sin(q5)*((641*3^(1/2))/20000 - 37/2000) - dq1*dqr1*cos(q2)^2*cos(q4)^2*cos(q6)*sin(q5)*((641*3^(1/2))/20000 - 37/2000) - dq1*dqr1*cos(q3)^2*cos(q4)^2*cos(q6)*sin(q5)*((641*3^(1/2))/20000 - 37/2000) + (37*dq1*dqr2*cos(q3)*cos(q4)*sin(q2)*sin(q4)*sin(q6))/1000 + (877*dq1*dqr2*cos(q4)*cos(q5)*sin(q2)*sin(q3)*sin(q6))/4000 + (1231*dq1*dqr2*cos(q5)*cos(q6)*sin(q2)*sin(q3)*sin(q4))/40000 + (37*dq1*dqr2*cos(q3)*cos(q5)*sin(q2)*sin(q5)*sin(q6))/2000 + dq5*dqr1*cos(q2)*cos(q3)*cos(q5)*sin(q6)*((641*3^(1/2))/40000 + 37/2000) + dq6*dqr1*cos(q2)*cos(q3)*cos(q6)*sin(q5)*((641*3^(1/2))/40000 + 37/2000) + dq2*dqr1*cos(q2)*cos(q3)*cos(q6)*sin(q4)*((37*3^(1/2))/4000 + 7539/40000) - dq3*dqr1*cos(q2)*cos(q3)*cos(q6)*sin(q4)*((37*3^(1/2))/4000 + 7539/40000) + dq5*dqr1*cos(q2)*cos(q3)*cos(q6)*sin(q5)*((641*3^(1/2))/80000 - 37/8000) + dq6*dqr1*cos(q2)*cos(q3)*cos(q5)*sin(q6)*((641*3^(1/2))/80000 - 37/8000) - dq1*dqr2*cos(q3)*sin(q2)*sin(q5)*sin(q6)*((641*3^(1/2))/20000 + 37/1000) + dq1*dqr2*cos(q6)*sin(q2)*sin(q3)*sin(q4)*((37*3^(1/2))/4000 + 7539/40000) - (37*dq1*dqr1*cos(q2)^2*cos(q3)^2*cos(q4)^2*cos(q5)^2*sin(q6))/250 - (37*3^(1/2)*dq2*dqr1*cos(q2)*cos(q3)*cos(q4)*sin(q6))/2000 + (37*3^(1/2)*dq3*dqr1*cos(q2)*cos(q3)*cos(q4)*sin(q6))/2000 + (37*3^(1/2)*dq2*dqr1*cos(q2)*cos(q3)*cos(q4)*cos(q5)^2*sin(q6))/1000 + (37*3^(1/2)*dq2*dqr1*cos(q2)*cos(q3)*cos(q5)^2*cos(q6)*sin(q4))/4000 - (37*3^(1/2)*dq3*dqr1*cos(q2)*cos(q3)*cos(q4)*cos(q5)^2*sin(q6))/1000 - (37*3^(1/2)*dq3*dqr1*cos(q2)*cos(q3)*cos(q5)^2*cos(q6)*sin(q4))/4000 + dq1*dqr1*cos(q2)^2*cos(q3)^2*cos(q4)*cos(q6)*sin(q4)*((1923*3^(1/2))/20000 + 37/200) + (37*3^(1/2)*dq1*dqr2*cos(q4)*cos(q5)^2*sin(q2)*sin(q3)*sin(q6))/1000 + (37*3^(1/2)*dq1*dqr2*cos(q5)^2*cos(q6)*sin(q2)*sin(q3)*sin(q4))/4000 - (37*dq1*dqr1*cos(q2)^2*cos(q3)^2*cos(q4)*cos(q5)^2*cos(q6)*sin(q4))/400 - (37*dq1*dqr1*cos(q2)^2*cos(q3)^2*cos(q4)^2*cos(q5)*cos(q6)*sin(q5))/500 - dq2*dqr1*cos(q2)*cos(q3)*cos(q4)*cos(q6)*sin(q5)*((37*3^(1/2))/4000 - 877/8000) + dq3*dqr1*cos(q2)*cos(q3)*cos(q4)*cos(q6)*sin(q5)*((37*3^(1/2))/4000 - 877/8000) + dq1*dqr1*cos(q2)^2*cos(q3)^2*cos(q4)^2*cos(q5)*sin(q6)*((641*3^(1/2))/5000 + 37/250) + dq1*dqr1*cos(q2)^2*cos(q3)^2*cos(q4)^2*cos(q6)*sin(q5)*((641*3^(1/2))/10000 - 37/1000) - dq1*dqr2*cos(q4)*cos(q6)*sin(q2)*sin(q3)*sin(q5)*((37*3^(1/2))/4000 - 877/8000) + dq2*dqr1*cos(q2)*cos(q3)*sin(q4)*sin(q5)*sin(q6)*((37*3^(1/2))/2000 - 1231/20000) - dq3*dqr1*cos(q2)*cos(q3)*sin(q4)*sin(q5)*sin(q6)*((37*3^(1/2))/2000 - 1231/20000) - (37*dq1*dqr2*cos(q3)*cos(q4)*cos(q5)^2*sin(q2)*sin(q4)*sin(q6))/500 - (37*dq1*dqr2*cos(q3)*cos(q4)^2*cos(q5)*sin(q2)*sin(q5)*sin(q6))/400 - (37*dq1*dqr1*cos(q3)^2*cos(q4)*cos(q5)*sin(q4)*sin(q5)*sin(q6))/400 + dq1*dqr2*sin(q2)*sin(q3)*sin(q4)*sin(q5)*sin(q6)*((37*3^(1/2))/2000 - 1231/20000) - dq1*dqr1*cos(q2)^2*cos(q4)*cos(q5)*cos(q6)*sin(q4)*((641*3^(1/2))/40000 - 37/4000) - dq1*dqr2*cos(q3)*cos(q4)^2*cos(q5)*cos(q6)*sin(q2)*((641*3^(1/2))/40000 - 37/4000) - dq1*dqr1*cos(q3)^2*cos(q4)*cos(q5)*cos(q6)*sin(q4)*((641*3^(1/2))/40000 - 37/4000) + dq1*dqr2*cos(q3)*cos(q4)^2*sin(q2)*sin(q5)*sin(q6)*((641*3^(1/2))/20000 + 37/1000) + dq1*dqr1*cos(q3)^2*cos(q4)*sin(q4)*sin(q5)*sin(q6)*((641*3^(1/2))/20000 + 37/1000) + dq1*dqr1*cos(q2)^2*cos(q3)^2*cos(q4)*cos(q5)*cos(q6)*sin(q4)*((641*3^(1/2))/20000 - 37/2000) - (37*dq1*dqr2*cos(q3)*cos(q4)*cos(q5)*cos(q6)*sin(q2)*sin(q4)*sin(q5))/1000 + dq1*dqr2*cos(q3)*cos(q4)*cos(q5)*sin(q2)*sin(q4)*sin(q6)*((641*3^(1/2))/10000 + 37/500) + dq1*dqr2*cos(q3)*cos(q4)*cos(q6)*sin(q2)*sin(q4)*sin(q5)*((641*3^(1/2))/20000 - 37/2000) + (37*3^(1/2)*dq2*dqr1*cos(q2)*cos(q3)*cos(q4)*cos(q5)*cos(q6)*sin(q5))/2000 - (37*3^(1/2)*dq3*dqr1*cos(q2)*cos(q3)*cos(q4)*cos(q5)*cos(q6)*sin(q5))/2000 + (37*3^(1/2)*dq1*dqr2*cos(q4)*cos(q5)*cos(q6)*sin(q2)*sin(q3)*sin(q5))/2000 - (37*3^(1/2)*dq1*dqr2*cos(q5)*sin(q2)*sin(q3)*sin(q4)*sin(q5)*sin(q6))/2000;
Y4_10_4=(37*dq3*dqr2*sin(q6))/2000 - (37*dq2*dqr2*sin(q6))/2000 + (37*dq2*dqr2*cos(q4)^2*sin(q6))/1000 + (37*dq2*dqr2*cos(q5)^2*sin(q6))/1000 - (37*dq3*dqr2*cos(q4)^2*sin(q6))/1000 - (37*dq3*dqr2*cos(q5)^2*sin(q6))/1000 + (37*3^(1/2)*dq5*dqr2*cos(q4)*sin(q6))/4000 + (37*3^(1/2)*dq5*dqr2*cos(q6)*sin(q4))/2000 + (37*3^(1/2)*dq6*dqr2*cos(q6)*sin(q4))/2000 - (37*dq2*dqr2*cos(q4)^2*cos(q5)^2*sin(q6))/500 + (37*dq3*dqr2*cos(q4)^2*cos(q5)^2*sin(q6))/500 - (87*dq1*dqr2*cos(q2)*cos(q6)*sin(q4))/400 + (87*dq2*dqr2*cos(q4)*cos(q6)*sin(q3))/400 + (37*dq2*dqr2*cos(q5)*cos(q6)*sin(q5))/2000 - (37*dq3*dqr2*cos(q5)*cos(q6)*sin(q5))/2000 - dq2*dqr2*cos(q5)*sin(q6)*((641*3^(1/2))/20000 + 37/1000) + dq3*dqr2*cos(q5)*sin(q6)*((641*3^(1/2))/20000 + 37/1000) - dq2*dqr2*cos(q6)*sin(q5)*((641*3^(1/2))/40000 - 37/4000) + dq3*dqr2*cos(q6)*sin(q5)*((641*3^(1/2))/40000 - 37/4000) - dq6*dqr2*cos(q4)*sin(q6)*((37*3^(1/2))/4000 + 1923/80000) + dq2*dqr2*cos(q4)^2*cos(q5)*sin(q6)*((641*3^(1/2))/10000 + 37/500) - dq3*dqr2*cos(q4)^2*cos(q5)*sin(q6)*((641*3^(1/2))/10000 + 37/500) + dq2*dqr2*cos(q4)^2*cos(q6)*sin(q5)*((641*3^(1/2))/20000 - 37/2000) - dq3*dqr2*cos(q4)^2*cos(q6)*sin(q5)*((641*3^(1/2))/20000 - 37/2000) - (37*3^(1/2)*dq6*dqr2*sin(q4)*sin(q5)*sin(q6))/4000 - (37*3^(1/2)*dq5*dqr2*cos(q4)*cos(q5)^2*sin(q6))/2000 - (37*3^(1/2)*dq5*dqr2*cos(q5)^2*cos(q6)*sin(q4))/2000 - (37*3^(1/2)*dq6*dqr2*cos(q4)*cos(q5)^2*sin(q6))/8000 - (37*3^(1/2)*dq6*dqr2*cos(q5)^2*cos(q6)*sin(q4))/2000 - (29*dq1*dqr2*cos(q2)*cos(q4)*cos(q5)*sin(q6))/100 - (29*dq1*dqr2*cos(q2)*cos(q4)*cos(q6)*sin(q5))/200 - (29*dq1*dqr2*cos(q2)*cos(q5)*cos(q6)*sin(q4))/400 + (29*dq2*dqr2*cos(q4)*cos(q5)*cos(q6)*sin(q3))/400 + (29*dq1*dqr2*cos(q2)*sin(q4)*sin(q5)*sin(q6))/200 - (29*dq2*dqr2*cos(q4)*sin(q3)*sin(q5)*sin(q6))/200 - (29*dq2*dqr2*cos(q5)*sin(q3)*sin(q4)*sin(q6))/100 - (29*dq2*dqr2*cos(q6)*sin(q3)*sin(q4)*sin(q5))/200 + dq2*dqr2*cos(q4)*cos(q6)*sin(q4)*((1923*3^(1/2))/40000 + 37/400) - dq3*dqr2*cos(q4)*cos(q6)*sin(q4)*((1923*3^(1/2))/40000 + 37/400) + dq5*dqr2*cos(q4)*cos(q5)*sin(q6)*((37*3^(1/2))/2000 + 1923/40000) + dq6*dqr2*cos(q4)*cos(q6)*sin(q5)*((37*3^(1/2))/2000 + 1923/40000) - dq1*dqr2*cos(q2)*cos(q6)*sin(q3)*((1923*3^(1/2))/40000 + 111/2000) + dq1*dqr2*cos(q3)*cos(q6)*sin(q2)*((1923*3^(1/2))/40000 + 111/2000) - dq5*dqr2*cos(q4)*cos(q6)*sin(q5)*((37*3^(1/2))/8000 - 1923/80000) + dq6*dqr2*cos(q4)*cos(q5)*sin(q6)*((111*3^(1/2))/8000 + 1923/80000) + (37*dq1*dqr2*cos(q2)*cos(q5)^2*cos(q6)*sin(q3))/4000 - (37*dq1*dqr2*cos(q3)*cos(q5)^2*cos(q6)*sin(q2))/4000 - (37*dq2*dqr2*cos(q4)*cos(q5)^2*cos(q6)*sin(q4))/800 - (37*dq2*dqr2*cos(q4)^2*cos(q5)*cos(q6)*sin(q5))/1000 + (37*dq3*dqr2*cos(q4)*cos(q5)^2*cos(q6)*sin(q4))/800 + (37*dq3*dqr2*cos(q4)^2*cos(q5)*cos(q6)*sin(q5))/1000 + dq1*dqr2*cos(q2)*cos(q4)^2*cos(q6)*sin(q3)*((1923*3^(1/2))/40000 + 37/400) - dq1*dqr2*cos(q3)*cos(q4)^2*cos(q6)*sin(q2)*((1923*3^(1/2))/40000 + 37/400) + (37*3^(1/2)*dq1*dqr3*cos(q4)*sin(q2)*sin(q3)*sin(q6))/2000 + (37*3^(1/2)*dq5*dqr2*cos(q5)*sin(q4)*sin(q5)*sin(q6))/1000 + (37*3^(1/2)*dq6*dqr2*cos(q5)*sin(q4)*sin(q5)*sin(q6))/4000 - (37*dq1*dqr2*cos(q2)*cos(q4)^2*cos(q5)^2*cos(q6)*sin(q3))/800 + (877*dq1*dqr2*cos(q2)*cos(q3)*cos(q4)*cos(q5)*sin(q6))/4000 + (1231*dq1*dqr2*cos(q2)*cos(q3)*cos(q5)*cos(q6)*sin(q4))/40000 - (37*dq1*dqr2*cos(q2)*cos(q4)*sin(q3)*sin(q4)*sin(q6))/1000 - (37*dq1*dqr2*cos(q2)*cos(q5)*sin(q3)*sin(q5)*sin(q6))/2000 - (877*dq1*dqr3*cos(q4)*cos(q5)*sin(q2)*sin(q3)*sin(q6))/4000 - (1231*dq1*dqr3*cos(q5)*cos(q6)*sin(q2)*sin(q3)*sin(q4))/40000 + (37*dq2*dqr2*cos(q4)*cos(q5)*sin(q4)*sin(q5)*sin(q6))/400 - (37*dq3*dqr2*cos(q4)*cos(q5)*sin(q4)*sin(q5)*sin(q6))/400 - dq1*dqr2*cos(q2)*cos(q5)*cos(q6)*sin(q3)*((641*3^(1/2))/40000 - 37/4000) + dq1*dqr2*cos(q3)*cos(q5)*cos(q6)*sin(q2)*((641*3^(1/2))/40000 - 37/4000) + dq2*dqr2*cos(q4)*cos(q5)*cos(q6)*sin(q4)*((641*3^(1/2))/40000 - 37/4000) - dq3*dqr2*cos(q4)*cos(q5)*cos(q6)*sin(q4)*((641*3^(1/2))/40000 - 37/4000) + dq1*dqr2*cos(q2)*cos(q3)*cos(q6)*sin(q4)*((37*3^(1/2))/4000 + 7539/40000) + dq1*dqr2*cos(q2)*sin(q3)*sin(q5)*sin(q6)*((641*3^(1/2))/20000 + 37/1000) - dq2*dqr2*cos(q4)*sin(q4)*sin(q5)*sin(q6)*((641*3^(1/2))/20000 + 37/1000) + dq3*dqr2*cos(q4)*sin(q4)*sin(q5)*sin(q6)*((641*3^(1/2))/20000 + 37/1000) - dq1*dqr3*cos(q6)*sin(q2)*sin(q3)*sin(q4)*((37*3^(1/2))/4000 + 7539/40000) - (37*3^(1/2)*dq1*dqr2*cos(q2)*cos(q3)*cos(q4)*sin(q6))/2000 - (37*3^(1/2)*dq5*dqr2*cos(q4)*cos(q5)*cos(q6)*sin(q5))/4000 - (37*3^(1/2)*dq6*dqr2*cos(q4)*cos(q5)*cos(q6)*sin(q5))/4000 + (37*3^(1/2)*dq1*dqr2*cos(q2)*cos(q3)*cos(q4)*cos(q5)^2*sin(q6))/1000 + (37*3^(1/2)*dq1*dqr2*cos(q2)*cos(q3)*cos(q5)^2*cos(q6)*sin(q4))/4000 - (37*3^(1/2)*dq1*dqr3*cos(q4)*cos(q5)^2*sin(q2)*sin(q3)*sin(q6))/1000 - (37*3^(1/2)*dq1*dqr3*cos(q5)^2*cos(q6)*sin(q2)*sin(q3)*sin(q4))/4000 - dq1*dqr2*cos(q2)*cos(q3)*cos(q4)*cos(q6)*sin(q5)*((37*3^(1/2))/4000 - 877/8000) + dq1*dqr3*cos(q4)*cos(q6)*sin(q2)*sin(q3)*sin(q5)*((37*3^(1/2))/4000 - 877/8000) + dq1*dqr2*cos(q2)*cos(q3)*sin(q4)*sin(q5)*sin(q6)*((37*3^(1/2))/2000 - 1231/20000) + (37*dq1*dqr2*cos(q2)*cos(q4)*cos(q5)^2*sin(q3)*sin(q4)*sin(q6))/500 + (37*dq1*dqr2*cos(q2)*cos(q4)^2*cos(q5)*sin(q3)*sin(q5)*sin(q6))/400 + (37*dq1*dqr3*cos(q3)*cos(q4)*cos(q5)^2*sin(q2)*sin(q4)*sin(q6))/500 - dq1*dqr3*sin(q2)*sin(q3)*sin(q4)*sin(q5)*sin(q6)*((37*3^(1/2))/2000 - 1231/20000) + dq1*dqr2*cos(q2)*cos(q4)^2*cos(q5)*cos(q6)*sin(q3)*((641*3^(1/2))/40000 - 37/4000) - dq1*dqr2*cos(q2)*cos(q4)^2*sin(q3)*sin(q5)*sin(q6)*((641*3^(1/2))/20000 + 37/1000) + (37*dq1*dqr2*cos(q2)*cos(q4)*cos(q5)*cos(q6)*sin(q3)*sin(q4)*sin(q5))/1000 + (37*dq1*dqr3*cos(q3)*cos(q4)*cos(q5)*cos(q6)*sin(q2)*sin(q4)*sin(q5))/1000 - dq1*dqr2*cos(q2)*cos(q4)*cos(q5)*sin(q3)*sin(q4)*sin(q6)*((641*3^(1/2))/10000 + 37/500) - dq1*dqr3*cos(q3)*cos(q4)*cos(q5)*sin(q2)*sin(q4)*sin(q6)*((641*3^(1/2))/10000 + 37/500) - dq1*dqr2*cos(q2)*cos(q4)*cos(q6)*sin(q3)*sin(q4)*sin(q5)*((641*3^(1/2))/20000 - 37/2000) - dq1*dqr3*cos(q3)*cos(q4)*cos(q6)*sin(q2)*sin(q4)*sin(q5)*((641*3^(1/2))/20000 - 37/2000) + (37*3^(1/2)*dq1*dqr2*cos(q2)*cos(q3)*cos(q4)*cos(q5)*cos(q6)*sin(q5))/2000 - (37*3^(1/2)*dq1*dqr2*cos(q2)*cos(q3)*cos(q5)*sin(q4)*sin(q5)*sin(q6))/2000 - (37*3^(1/2)*dq1*dqr3*cos(q4)*cos(q5)*cos(q6)*sin(q2)*sin(q3)*sin(q5))/2000 + (37*3^(1/2)*dq1*dqr3*cos(q5)*sin(q2)*sin(q3)*sin(q4)*sin(q5)*sin(q6))/2000;
Y4_10_5=(37*dq2*dqr3*sin(q6))/2000 - (37*dq3*dqr3*sin(q6))/2000 - (111*dq5*dqr4*sin(q6))/4000 + dq6*dqr4*sin(q6)*((1923*3^(1/2))/80000 + 37/4000) - (37*dq2*dqr3*cos(q4)^2*sin(q6))/1000 - (37*dq2*dqr3*cos(q5)^2*sin(q6))/1000 + (37*dq3*dqr3*cos(q4)^2*sin(q6))/1000 + (37*dq3*dqr3*cos(q5)^2*sin(q6))/1000 + (111*dq5*dqr4*cos(q5)^2*sin(q6))/2000 + (111*dq6*dqr4*cos(q5)^2*sin(q6))/8000 - (37*3^(1/2)*dq5*dqr3*cos(q4)*sin(q6))/4000 - (37*3^(1/2)*dq5*dqr3*cos(q6)*sin(q4))/2000 - (37*3^(1/2)*dq6*dqr3*cos(q6)*sin(q4))/2000 + (37*dq2*dqr3*cos(q4)^2*cos(q5)^2*sin(q6))/500 - (37*dq3*dqr3*cos(q4)^2*cos(q5)^2*sin(q6))/500 - (37*dq2*dqr3*cos(q5)*cos(q6)*sin(q5))/2000 + (37*dq3*dqr3*cos(q5)*cos(q6)*sin(q5))/2000 + (111*dq5*dqr4*cos(q5)*cos(q6)*sin(q5))/4000 + (111*dq6*dqr4*cos(q5)*cos(q6)*sin(q5))/4000 - (111*dq1*dqr5*sin(q2)*sin(q3)*sin(q6))/4000 + dq2*dqr3*cos(q5)*sin(q6)*((641*3^(1/2))/20000 + 37/1000) - dq3*dqr3*cos(q5)*sin(q6)*((641*3^(1/2))/20000 + 37/1000) + dq5*dqr4*cos(q5)*sin(q6)*((641*3^(1/2))/40000 + 37/2000) + dq6*dqr4*cos(q6)*sin(q5)*((641*3^(1/2))/40000 + 37/2000) + dq2*dqr3*cos(q6)*sin(q5)*((641*3^(1/2))/40000 - 37/4000) - dq3*dqr3*cos(q6)*sin(q5)*((641*3^(1/2))/40000 - 37/4000) + dq6*dqr3*cos(q4)*sin(q6)*((37*3^(1/2))/4000 + 1923/80000) + dq5*dqr4*cos(q6)*sin(q5)*((641*3^(1/2))/80000 - 37/8000) + dq6*dqr4*cos(q5)*sin(q6)*((641*3^(1/2))/80000 - 37/8000) + (111*dq1*dqr5*cos(q5)^2*sin(q2)*sin(q3)*sin(q6))/2000 - dq2*dqr3*cos(q4)^2*cos(q5)*sin(q6)*((641*3^(1/2))/10000 + 37/500) + dq3*dqr3*cos(q4)^2*cos(q5)*sin(q6)*((641*3^(1/2))/10000 + 37/500) - dq2*dqr3*cos(q4)^2*cos(q6)*sin(q5)*((641*3^(1/2))/20000 - 37/2000) + dq3*dqr3*cos(q4)^2*cos(q6)*sin(q5)*((641*3^(1/2))/20000 - 37/2000) + (37*3^(1/2)*dq6*dqr3*sin(q4)*sin(q5)*sin(q6))/4000 + (37*3^(1/2)*dq5*dqr3*cos(q4)*cos(q5)^2*sin(q6))/2000 + (37*3^(1/2)*dq5*dqr3*cos(q5)^2*cos(q6)*sin(q4))/2000 + (37*3^(1/2)*dq6*dqr3*cos(q4)*cos(q5)^2*sin(q6))/8000 + (37*3^(1/2)*dq6*dqr3*cos(q5)^2*cos(q6)*sin(q4))/2000 - dq2*dqr3*cos(q4)*cos(q6)*sin(q4)*((1923*3^(1/2))/40000 + 37/400) + dq3*dqr3*cos(q4)*cos(q6)*sin(q4)*((1923*3^(1/2))/40000 + 37/400) - dq5*dqr3*cos(q4)*cos(q5)*sin(q6)*((37*3^(1/2))/2000 + 1923/40000) - dq6*dqr3*cos(q4)*cos(q6)*sin(q5)*((37*3^(1/2))/2000 + 1923/40000) + dq1*dqr3*cos(q2)*cos(q6)*sin(q3)*((1923*3^(1/2))/40000 + 111/2000) - dq1*dqr3*cos(q3)*cos(q6)*sin(q2)*((1923*3^(1/2))/40000 + 111/2000) + dq5*dqr3*cos(q4)*cos(q6)*sin(q5)*((37*3^(1/2))/8000 - 1923/80000) - dq6*dqr3*cos(q4)*cos(q5)*sin(q6)*((111*3^(1/2))/8000 + 1923/80000) - (37*dq1*dqr3*cos(q2)*cos(q5)^2*cos(q6)*sin(q3))/4000 + (37*dq1*dqr3*cos(q3)*cos(q5)^2*cos(q6)*sin(q2))/4000 + (37*dq2*dqr3*cos(q4)*cos(q5)^2*cos(q6)*sin(q4))/800 + (37*dq2*dqr3*cos(q4)^2*cos(q5)*cos(q6)*sin(q5))/1000 - (37*dq3*dqr3*cos(q4)*cos(q5)^2*cos(q6)*sin(q4))/800 - (37*dq3*dqr3*cos(q4)^2*cos(q5)*cos(q6)*sin(q5))/1000 - dq1*dqr3*cos(q2)*cos(q4)^2*cos(q6)*sin(q3)*((1923*3^(1/2))/40000 + 37/400) + dq1*dqr3*cos(q3)*cos(q4)^2*cos(q6)*sin(q2)*((1923*3^(1/2))/40000 + 37/400) - (37*3^(1/2)*dq5*dqr3*cos(q5)*sin(q4)*sin(q5)*sin(q6))/1000 - (37*3^(1/2)*dq6*dqr3*cos(q5)*sin(q4)*sin(q5)*sin(q6))/4000 + (37*dq1*dqr3*cos(q2)*cos(q4)^2*cos(q5)^2*cos(q6)*sin(q3))/800 - (37*dq1*dqr3*cos(q3)*cos(q4)^2*cos(q5)^2*cos(q6)*sin(q2))/800 - (877*dq1*dqr3*cos(q2)*cos(q3)*cos(q4)*cos(q5)*sin(q6))/4000 - (1231*dq1*dqr3*cos(q2)*cos(q3)*cos(q5)*cos(q6)*sin(q4))/40000 + (37*dq1*dqr3*cos(q2)*cos(q4)*sin(q3)*sin(q4)*sin(q6))/1000 - (37*dq1*dqr3*cos(q3)*cos(q4)*sin(q2)*sin(q4)*sin(q6))/1000 + (37*dq1*dqr3*cos(q2)*cos(q5)*sin(q3)*sin(q5)*sin(q6))/2000 - (37*dq1*dqr3*cos(q3)*cos(q5)*sin(q2)*sin(q5)*sin(q6))/2000 + (111*dq1*dqr5*cos(q5)*cos(q6)*sin(q2)*sin(q3)*sin(q5))/4000 - (37*dq2*dqr3*cos(q4)*cos(q5)*sin(q4)*sin(q5)*sin(q6))/400 + (37*dq3*dqr3*cos(q4)*cos(q5)*sin(q4)*sin(q5)*sin(q6))/400 + dq1*dqr3*cos(q2)*cos(q5)*cos(q6)*sin(q3)*((641*3^(1/2))/40000 - 37/4000) - dq1*dqr3*cos(q3)*cos(q5)*cos(q6)*sin(q2)*((641*3^(1/2))/40000 - 37/4000) - dq2*dqr3*cos(q4)*cos(q5)*cos(q6)*sin(q4)*((641*3^(1/2))/40000 - 37/4000) + dq3*dqr3*cos(q4)*cos(q5)*cos(q6)*sin(q4)*((641*3^(1/2))/40000 - 37/4000) - dq1*dqr3*cos(q2)*cos(q3)*cos(q6)*sin(q4)*((37*3^(1/2))/4000 + 7539/40000) - dq1*dqr3*cos(q2)*sin(q3)*sin(q5)*sin(q6)*((641*3^(1/2))/20000 + 37/1000) + dq1*dqr3*cos(q3)*sin(q2)*sin(q5)*sin(q6)*((641*3^(1/2))/20000 + 37/1000) + dq2*dqr3*cos(q4)*sin(q4)*sin(q5)*sin(q6)*((641*3^(1/2))/20000 + 37/1000) - dq3*dqr3*cos(q4)*sin(q4)*sin(q5)*sin(q6)*((641*3^(1/2))/20000 + 37/1000) + dq1*dqr5*cos(q5)*sin(q2)*sin(q3)*sin(q6)*((641*3^(1/2))/40000 + 37/2000) + dq1*dqr5*cos(q6)*sin(q2)*sin(q3)*sin(q5)*((641*3^(1/2))/80000 - 37/8000) + (37*3^(1/2)*dq1*dqr3*cos(q2)*cos(q3)*cos(q4)*sin(q6))/2000 + (37*3^(1/2)*dq5*dqr3*cos(q4)*cos(q5)*cos(q6)*sin(q5))/4000 + (37*3^(1/2)*dq6*dqr3*cos(q4)*cos(q5)*cos(q6)*sin(q5))/4000 - (37*3^(1/2)*dq1*dqr3*cos(q2)*cos(q3)*cos(q4)*cos(q5)^2*sin(q6))/1000 - (37*3^(1/2)*dq1*dqr3*cos(q2)*cos(q3)*cos(q5)^2*cos(q6)*sin(q4))/4000 + dq1*dqr3*cos(q2)*cos(q3)*cos(q4)*cos(q6)*sin(q5)*((37*3^(1/2))/4000 - 877/8000) - dq1*dqr3*cos(q2)*cos(q3)*sin(q4)*sin(q5)*sin(q6)*((37*3^(1/2))/2000 - 1231/20000) - dq1*dqr5*cos(q3)*cos(q6)*sin(q2)*sin(q4)*sin(q5)*((37*3^(1/2))/8000 - 1923/80000) - (37*dq1*dqr3*cos(q2)*cos(q4)*cos(q5)^2*sin(q3)*sin(q4)*sin(q6))/500 - (37*dq1*dqr3*cos(q2)*cos(q4)^2*cos(q5)*sin(q3)*sin(q5)*sin(q6))/400 + (37*dq1*dqr3*cos(q3)*cos(q4)^2*cos(q5)*sin(q2)*sin(q5)*sin(q6))/400 - dq1*dqr3*cos(q2)*cos(q4)^2*cos(q5)*cos(q6)*sin(q3)*((641*3^(1/2))/40000 - 37/4000) + dq1*dqr3*cos(q3)*cos(q4)^2*cos(q5)*cos(q6)*sin(q2)*((641*3^(1/2))/40000 - 37/4000) + dq1*dqr3*cos(q2)*cos(q4)^2*sin(q3)*sin(q5)*sin(q6)*((641*3^(1/2))/20000 + 37/1000) - dq1*dqr3*cos(q3)*cos(q4)^2*sin(q2)*sin(q5)*sin(q6)*((641*3^(1/2))/20000 + 37/1000) - (37*dq1*dqr3*cos(q2)*cos(q4)*cos(q5)*cos(q6)*sin(q3)*sin(q4)*sin(q5))/1000 + dq1*dqr3*cos(q2)*cos(q4)*cos(q5)*sin(q3)*sin(q4)*sin(q6)*((641*3^(1/2))/10000 + 37/500) + dq1*dqr3*cos(q2)*cos(q4)*cos(q6)*sin(q3)*sin(q4)*sin(q5)*((641*3^(1/2))/20000 - 37/2000) - (37*3^(1/2)*dq1*dqr3*cos(q2)*cos(q3)*cos(q4)*cos(q5)*cos(q6)*sin(q5))/2000 + (37*3^(1/2)*dq1*dqr3*cos(q2)*cos(q3)*cos(q5)*sin(q4)*sin(q5)*sin(q6))/2000 - (37*3^(1/2)*dq1*dqr5*cos(q3)*cos(q5)*cos(q6)*sin(q2)*sin(q4)*sin(q5))/4000;
Y4_10_6=dq4*dqr6*sin(q6)*((1923*3^(1/2))/80000 + 37/4000) - (37*dq6*dqr5*sin(q6))/4000 - (111*dq4*dqr5*sin(q6))/4000 + (111*dq4*dqr5*cos(q5)^2*sin(q6))/2000 + (111*dq4*dqr6*cos(q5)^2*sin(q6))/8000 + (37*3^(1/2)*dq2*dqr5*cos(q4)*sin(q6))/4000 + (37*3^(1/2)*dq2*dqr5*cos(q6)*sin(q4))/2000 + (37*3^(1/2)*dq2*dqr6*cos(q6)*sin(q4))/2000 - (37*3^(1/2)*dq3*dqr5*cos(q4)*sin(q6))/4000 - (37*3^(1/2)*dq3*dqr5*cos(q6)*sin(q4))/2000 - (37*3^(1/2)*dq3*dqr6*cos(q6)*sin(q4))/2000 - (111*dq1*dqr5*cos(q2)*cos(q3)*sin(q6))/4000 + (111*dq4*dqr5*cos(q5)*cos(q6)*sin(q5))/4000 + (111*dq4*dqr6*cos(q5)*cos(q6)*sin(q5))/4000 + dq5*dqr5*cos(q5)*sin(q6)*((641*3^(1/2))/20000 + 37/1000) + dq5*dqr6*cos(q6)*sin(q5)*((641*3^(1/2))/20000 + 37/1000) + dq6*dqr5*cos(q6)*sin(q5)*((641*3^(1/2))/20000 + 37/1000) + dq6*dqr6*cos(q5)*sin(q6)*((641*3^(1/2))/20000 + 37/1000) + dq6*dqr6*cos(q6)*sin(q5)*((641*3^(1/2))/40000 + 37/800) + dq4*dqr5*cos(q5)*sin(q6)*((641*3^(1/2))/40000 + 37/2000) + dq4*dqr6*cos(q6)*sin(q5)*((641*3^(1/2))/40000 + 37/2000) + dq5*dqr6*cos(q5)*sin(q6)*((641*3^(1/2))/40000 + 37/2000) + dq6*dqr5*cos(q5)*sin(q6)*((641*3^(1/2))/40000 + 37/2000) + dq5*dqr5*cos(q6)*sin(q5)*((641*3^(1/2))/40000 - 37/4000) - dq2*dqr6*cos(q4)*sin(q6)*((37*3^(1/2))/4000 + 1923/80000) + dq3*dqr6*cos(q4)*sin(q6)*((37*3^(1/2))/4000 + 1923/80000) + dq4*dqr5*cos(q6)*sin(q5)*((641*3^(1/2))/80000 - 37/8000) + dq4*dqr6*cos(q5)*sin(q6)*((641*3^(1/2))/80000 - 37/8000) + (111*dq1*dqr6*cos(q5)^2*sin(q2)*sin(q3)*sin(q6))/8000 - (37*3^(1/2)*dq2*dqr6*sin(q4)*sin(q5)*sin(q6))/4000 + (37*3^(1/2)*dq3*dqr6*sin(q4)*sin(q5)*sin(q6))/4000 - (37*3^(1/2)*dq2*dqr5*cos(q4)*cos(q5)^2*sin(q6))/2000 - (37*3^(1/2)*dq2*dqr5*cos(q5)^2*cos(q6)*sin(q4))/2000 - (37*3^(1/2)*dq2*dqr6*cos(q4)*cos(q5)^2*sin(q6))/8000 - (37*3^(1/2)*dq2*dqr6*cos(q5)^2*cos(q6)*sin(q4))/2000 + (37*3^(1/2)*dq3*dqr5*cos(q4)*cos(q5)^2*sin(q6))/2000 + (37*3^(1/2)*dq3*dqr5*cos(q5)^2*cos(q6)*sin(q4))/2000 + (37*3^(1/2)*dq3*dqr6*cos(q4)*cos(q5)^2*sin(q6))/8000 + (37*3^(1/2)*dq3*dqr6*cos(q5)^2*cos(q6)*sin(q4))/2000 + dq2*dqr5*cos(q4)*cos(q5)*sin(q6)*((37*3^(1/2))/2000 + 1923/40000) + dq2*dqr6*cos(q4)*cos(q6)*sin(q5)*((37*3^(1/2))/2000 + 1923/40000) - dq3*dqr5*cos(q4)*cos(q5)*sin(q6)*((37*3^(1/2))/2000 + 1923/40000) - dq3*dqr6*cos(q4)*cos(q6)*sin(q5)*((37*3^(1/2))/2000 + 1923/40000) + dq1*dqr6*cos(q2)*cos(q3)*sin(q6)*((1923*3^(1/2))/80000 + 37/4000) - dq2*dqr5*cos(q4)*cos(q6)*sin(q5)*((37*3^(1/2))/8000 - 1923/80000) + dq3*dqr5*cos(q4)*cos(q6)*sin(q5)*((37*3^(1/2))/8000 - 1923/80000) + dq2*dqr6*cos(q4)*cos(q5)*sin(q6)*((111*3^(1/2))/8000 + 1923/80000) - dq3*dqr6*cos(q4)*cos(q5)*sin(q6)*((111*3^(1/2))/8000 + 1923/80000) + (111*dq1*dqr5*cos(q2)*cos(q3)*cos(q5)^2*sin(q6))/2000 + (111*dq1*dqr6*cos(q2)*cos(q3)*cos(q5)^2*sin(q6))/8000 + dq1*dqr6*sin(q2)*sin(q3)*sin(q6)*((1923*3^(1/2))/80000 + 37/4000) - (37*3^(1/2)*dq1*dqr5*cos(q2)*sin(q3)*sin(q4)*sin(q6))/4000 + (37*3^(1/2)*dq1*dqr5*cos(q3)*sin(q2)*sin(q4)*sin(q6))/4000 + (37*3^(1/2)*dq2*dqr5*cos(q5)*sin(q4)*sin(q5)*sin(q6))/1000 + (37*3^(1/2)*dq2*dqr6*cos(q5)*sin(q4)*sin(q5)*sin(q6))/4000 - (37*3^(1/2)*dq3*dqr5*cos(q5)*sin(q4)*sin(q5)*sin(q6))/1000 - (37*3^(1/2)*dq3*dqr6*cos(q5)*sin(q4)*sin(q5)*sin(q6))/4000 + (111*dq1*dqr5*cos(q2)*cos(q3)*cos(q5)*cos(q6)*sin(q5))/4000 + (111*dq1*dqr6*cos(q2)*cos(q3)*cos(q5)*cos(q6)*sin(q5))/4000 + (111*dq1*dqr6*cos(q5)*cos(q6)*sin(q2)*sin(q3)*sin(q5))/4000 + dq1*dqr5*cos(q2)*cos(q3)*cos(q5)*sin(q6)*((641*3^(1/2))/40000 + 37/2000) + dq1*dqr6*cos(q2)*cos(q3)*cos(q6)*sin(q5)*((641*3^(1/2))/40000 + 37/2000) + dq1*dqr5*cos(q2)*cos(q3)*cos(q6)*sin(q5)*((641*3^(1/2))/80000 - 37/8000) + dq1*dqr6*cos(q2)*cos(q3)*cos(q5)*sin(q6)*((641*3^(1/2))/80000 - 37/8000) + dq1*dqr6*cos(q6)*sin(q2)*sin(q3)*sin(q5)*((641*3^(1/2))/40000 + 37/2000) + dq1*dqr6*cos(q2)*sin(q3)*sin(q4)*sin(q6)*((37*3^(1/2))/4000 + 1923/80000) - dq1*dqr6*cos(q3)*sin(q2)*sin(q4)*sin(q6)*((37*3^(1/2))/4000 + 1923/80000) + dq1*dqr6*cos(q5)*sin(q2)*sin(q3)*sin(q6)*((641*3^(1/2))/80000 - 37/8000) + (37*3^(1/2)*dq1*dqr5*cos(q2)*cos(q4)*cos(q6)*sin(q3))/2000 - (37*3^(1/2)*dq1*dqr5*cos(q3)*cos(q4)*cos(q6)*sin(q2))/2000 + (37*3^(1/2)*dq1*dqr6*cos(q2)*cos(q4)*cos(q6)*sin(q3))/2000 - (37*3^(1/2)*dq1*dqr6*cos(q3)*cos(q4)*cos(q6)*sin(q2))/2000 - (37*3^(1/2)*dq2*dqr5*cos(q4)*cos(q5)*cos(q6)*sin(q5))/4000 - (37*3^(1/2)*dq2*dqr6*cos(q4)*cos(q5)*cos(q6)*sin(q5))/4000 + (37*3^(1/2)*dq3*dqr5*cos(q4)*cos(q5)*cos(q6)*sin(q5))/4000 + (37*3^(1/2)*dq3*dqr6*cos(q4)*cos(q5)*cos(q6)*sin(q5))/4000 - (37*3^(1/2)*dq1*dqr5*cos(q2)*cos(q4)*cos(q5)^2*cos(q6)*sin(q3))/2000 + (37*3^(1/2)*dq1*dqr5*cos(q3)*cos(q4)*cos(q5)^2*cos(q6)*sin(q2))/2000 - (37*3^(1/2)*dq1*dqr6*cos(q2)*cos(q4)*cos(q5)^2*cos(q6)*sin(q3))/2000 + (37*3^(1/2)*dq1*dqr6*cos(q3)*cos(q4)*cos(q5)^2*cos(q6)*sin(q2))/2000 + (37*3^(1/2)*dq1*dqr5*cos(q2)*cos(q5)^2*sin(q3)*sin(q4)*sin(q6))/2000 - (37*3^(1/2)*dq1*dqr5*cos(q3)*cos(q5)^2*sin(q2)*sin(q4)*sin(q6))/2000 + (37*3^(1/2)*dq1*dqr6*cos(q2)*cos(q5)^2*sin(q3)*sin(q4)*sin(q6))/8000 - (37*3^(1/2)*dq1*dqr6*cos(q3)*cos(q5)^2*sin(q2)*sin(q4)*sin(q6))/8000 - dq1*dqr5*cos(q2)*cos(q5)*sin(q3)*sin(q4)*sin(q6)*((37*3^(1/2))/2000 + 1923/40000) + dq1*dqr5*cos(q3)*cos(q5)*sin(q2)*sin(q4)*sin(q6)*((37*3^(1/2))/2000 + 1923/40000) - dq1*dqr6*cos(q2)*cos(q6)*sin(q3)*sin(q4)*sin(q5)*((37*3^(1/2))/2000 + 1923/40000) + dq1*dqr6*cos(q3)*cos(q6)*sin(q2)*sin(q4)*sin(q5)*((37*3^(1/2))/2000 + 1923/40000) + dq1*dqr5*cos(q2)*cos(q6)*sin(q3)*sin(q4)*sin(q5)*((37*3^(1/2))/8000 - 1923/80000) - dq1*dqr6*cos(q2)*cos(q5)*sin(q3)*sin(q4)*sin(q6)*((111*3^(1/2))/8000 + 1923/80000) + dq1*dqr6*cos(q3)*cos(q5)*sin(q2)*sin(q4)*sin(q6)*((111*3^(1/2))/8000 + 1923/80000) - (37*3^(1/2)*dq1*dqr6*cos(q2)*cos(q4)*sin(q3)*sin(q5)*sin(q6))/4000 + (37*3^(1/2)*dq1*dqr6*cos(q3)*cos(q4)*sin(q2)*sin(q5)*sin(q6))/4000 + (37*3^(1/2)*dq1*dqr5*cos(q2)*cos(q4)*cos(q5)*sin(q3)*sin(q5)*sin(q6))/1000 + (37*3^(1/2)*dq1*dqr5*cos(q2)*cos(q5)*cos(q6)*sin(q3)*sin(q4)*sin(q5))/4000 - (37*3^(1/2)*dq1*dqr5*cos(q3)*cos(q4)*cos(q5)*sin(q2)*sin(q5)*sin(q6))/1000 + (37*3^(1/2)*dq1*dqr6*cos(q2)*cos(q4)*cos(q5)*sin(q3)*sin(q5)*sin(q6))/4000 + (37*3^(1/2)*dq1*dqr6*cos(q2)*cos(q5)*cos(q6)*sin(q3)*sin(q4)*sin(q5))/4000 - (37*3^(1/2)*dq1*dqr6*cos(q3)*cos(q4)*cos(q5)*sin(q2)*sin(q5)*sin(q6))/4000 - (37*3^(1/2)*dq1*dqr6*cos(q3)*cos(q5)*cos(q6)*sin(q2)*sin(q4)*sin(q5))/4000;
Y4_10_7=(37*ddqr5*cos(q6))/2000 + (37*ddqr6*cos(q6))/2000 - (37*dq5*dqr6*sin(q6))/4000 - (37*dq6*dqr6*sin(q6))/2000 - ddqr4*cos(q6)*((1923*3^(1/2))/40000 + 37/2000) - (111*ddqr4*cos(q5)^2*cos(q6))/4000 - (87*ddqr2*cos(q3)*cos(q4)*cos(q6))/400 + (1231*ddqr2*cos(q4)*cos(q5)*cos(q6))/40000 - (1231*ddqr3*cos(q4)*cos(q5)*cos(q6))/40000 - (87*ddqr1*cos(q6)*sin(q2)*sin(q4))/400 - (877*ddqr2*cos(q5)*sin(q4)*sin(q6))/4000 + (877*ddqr3*cos(q5)*sin(q4)*sin(q6))/4000 + (111*ddqr4*cos(q5)*sin(q5)*sin(q6))/2000 - ddqr6*cos(q5)*cos(q6)*((641*3^(1/2))/20000 + 37/1000) - ddqr4*cos(q5)*cos(q6)*((641*3^(1/2))/40000 - 37/4000) - ddqr5*cos(q5)*cos(q6)*((641*3^(1/2))/40000 - 37/4000) + ddqr2*cos(q4)*cos(q6)*((37*3^(1/2))/4000 + 7539/40000) - ddqr3*cos(q4)*cos(q6)*((37*3^(1/2))/4000 + 7539/40000) + ddqr4*sin(q5)*sin(q6)*((641*3^(1/2))/20000 + 37/1000) + ddqr5*sin(q5)*sin(q6)*((641*3^(1/2))/20000 + 37/1000) + ddqr6*sin(q5)*sin(q6)*((641*3^(1/2))/40000 + 37/800) + (37*3^(1/2)*ddqr2*sin(q4)*sin(q6))/2000 - (37*3^(1/2)*ddqr3*sin(q4)*sin(q6))/2000 + (37*3^(1/2)*ddqr2*cos(q4)*cos(q5)^2*cos(q6))/4000 - (37*3^(1/2)*ddqr3*cos(q4)*cos(q5)^2*cos(q6))/4000 + (21*ddqr1*cos(q2)*cos(q3)*cos(q4)*cos(q6))/4000 - (29*ddqr2*cos(q3)*cos(q4)*cos(q5)*cos(q6))/400 - (37*3^(1/2)*ddqr2*cos(q5)^2*sin(q4)*sin(q6))/1000 + (37*3^(1/2)*ddqr3*cos(q5)^2*sin(q4)*sin(q6))/1000 + (21*ddqr1*cos(q4)*cos(q6)*sin(q2)*sin(q3))/4000 - (29*ddqr1*cos(q4)*cos(q5)*sin(q2)*sin(q6))/100 - (29*ddqr1*cos(q4)*cos(q6)*sin(q2)*sin(q5))/200 - (29*ddqr1*cos(q5)*cos(q6)*sin(q2)*sin(q4))/400 + (29*ddqr2*cos(q3)*cos(q4)*sin(q5)*sin(q6))/200 + (29*ddqr2*cos(q3)*cos(q5)*sin(q4)*sin(q6))/100 + (29*ddqr2*cos(q3)*cos(q6)*sin(q4)*sin(q5))/200 + (29*ddqr1*sin(q2)*sin(q4)*sin(q5)*sin(q6))/200 - ddqr1*cos(q2)*cos(q3)*cos(q6)*((1923*3^(1/2))/40000 + 37/2000) - (111*ddqr1*cos(q2)*cos(q3)*cos(q5)^2*cos(q6))/4000 + ddqr2*cos(q6)*sin(q4)*sin(q5)*((37*3^(1/2))/4000 - 877/8000) - ddqr3*cos(q6)*sin(q4)*sin(q5)*((37*3^(1/2))/4000 - 877/8000) + ddqr2*cos(q4)*sin(q5)*sin(q6)*((37*3^(1/2))/2000 - 1231/20000) - ddqr3*cos(q4)*sin(q5)*sin(q6)*((37*3^(1/2))/2000 - 1231/20000) - ddqr1*cos(q6)*sin(q2)*sin(q3)*((1923*3^(1/2))/40000 + 37/2000) - (111*ddqr1*cos(q5)^2*cos(q6)*sin(q2)*sin(q3))/4000 - (7*ddqr1*cos(q2)*cos(q3)*cos(q4)*sin(q5)*sin(q6))/2000 - (7*ddqr1*cos(q2)*cos(q3)*cos(q5)*sin(q4)*sin(q6))/1000 - (7*ddqr1*cos(q2)*cos(q3)*cos(q6)*sin(q4)*sin(q5))/2000 - (877*ddqr1*cos(q2)*cos(q4)*cos(q5)*sin(q3)*sin(q6))/4000 - (1231*ddqr1*cos(q2)*cos(q5)*cos(q6)*sin(q3)*sin(q4))/40000 + (877*ddqr1*cos(q3)*cos(q4)*cos(q5)*sin(q2)*sin(q6))/4000 + (1231*ddqr1*cos(q3)*cos(q5)*cos(q6)*sin(q2)*sin(q4))/40000 + (7*ddqr1*cos(q4)*cos(q5)*cos(q6)*sin(q2)*sin(q3))/4000 + (111*ddqr1*cos(q2)*cos(q3)*cos(q5)*sin(q5)*sin(q6))/2000 - (7*ddqr1*cos(q4)*sin(q2)*sin(q3)*sin(q5)*sin(q6))/2000 - (7*ddqr1*cos(q5)*sin(q2)*sin(q3)*sin(q4)*sin(q6))/1000 - (7*ddqr1*cos(q6)*sin(q2)*sin(q3)*sin(q4)*sin(q5))/2000 + (111*ddqr1*cos(q5)*sin(q2)*sin(q3)*sin(q5)*sin(q6))/2000 - ddqr1*cos(q2)*cos(q3)*cos(q5)*cos(q6)*((641*3^(1/2))/40000 - 37/4000) + ddqr1*cos(q2)*cos(q3)*sin(q5)*sin(q6)*((641*3^(1/2))/20000 + 37/1000) - ddqr1*cos(q5)*cos(q6)*sin(q2)*sin(q3)*((641*3^(1/2))/40000 - 37/4000) - ddqr1*cos(q2)*cos(q6)*sin(q3)*sin(q4)*((37*3^(1/2))/4000 + 7539/40000) + ddqr1*cos(q3)*cos(q6)*sin(q2)*sin(q4)*((37*3^(1/2))/4000 + 7539/40000) + ddqr1*sin(q2)*sin(q3)*sin(q5)*sin(q6)*((641*3^(1/2))/20000 + 37/1000) + (37*3^(1/2)*ddqr1*cos(q2)*cos(q4)*sin(q3)*sin(q6))/2000 - (37*3^(1/2)*ddqr1*cos(q3)*cos(q4)*sin(q2)*sin(q6))/2000 - (37*3^(1/2)*ddqr2*cos(q4)*cos(q5)*sin(q5)*sin(q6))/2000 - (37*3^(1/2)*ddqr2*cos(q5)*cos(q6)*sin(q4)*sin(q5))/2000 + (37*3^(1/2)*ddqr3*cos(q4)*cos(q5)*sin(q5)*sin(q6))/2000 + (37*3^(1/2)*ddqr3*cos(q5)*cos(q6)*sin(q4)*sin(q5))/2000 + (7*ddqr1*cos(q2)*cos(q3)*cos(q4)*cos(q5)*cos(q6))/4000 + ddqr1*cos(q2)*cos(q4)*cos(q6)*sin(q3)*sin(q5)*((37*3^(1/2))/4000 - 877/8000) - ddqr1*cos(q3)*cos(q4)*cos(q6)*sin(q2)*sin(q5)*((37*3^(1/2))/4000 - 877/8000) - ddqr1*cos(q2)*sin(q3)*sin(q4)*sin(q5)*sin(q6)*((37*3^(1/2))/2000 - 1231/20000) + ddqr1*cos(q3)*sin(q2)*sin(q4)*sin(q5)*sin(q6)*((37*3^(1/2))/2000 - 1231/20000) - (37*3^(1/2)*ddqr1*cos(q2)*cos(q4)*cos(q5)^2*sin(q3)*sin(q6))/1000 - (37*3^(1/2)*ddqr1*cos(q2)*cos(q5)^2*cos(q6)*sin(q3)*sin(q4))/4000 + (37*3^(1/2)*ddqr1*cos(q3)*cos(q4)*cos(q5)^2*sin(q2)*sin(q6))/1000 + (37*3^(1/2)*ddqr1*cos(q3)*cos(q5)^2*cos(q6)*sin(q2)*sin(q4))/4000 - (37*3^(1/2)*ddqr1*cos(q2)*cos(q4)*cos(q5)*cos(q6)*sin(q3)*sin(q5))/2000 + (37*3^(1/2)*ddqr1*cos(q3)*cos(q4)*cos(q5)*cos(q6)*sin(q2)*sin(q5))/2000 + (37*3^(1/2)*ddqr1*cos(q2)*cos(q5)*sin(q3)*sin(q4)*sin(q5)*sin(q6))/2000 - (37*3^(1/2)*ddqr1*cos(q3)*cos(q5)*sin(q2)*sin(q4)*sin(q5)*sin(q6))/2000;
Y4_13_1=(37*sin(q2 - q3)*cos(q4))/1000;
Y4_14_1=(37*sin(q2 - q3)*sin(q4)*sin(q5))/1000 - (37*sin(q2 - q3)*cos(q4)*cos(q5))/2000 + sin(q2 - q3)*cos(q4)*((641*3^(1/2))/20000 + 37/1000);
Y4_18_1=ddqr4 - (dq2*dqr2*sin(2*q4))/2 + (dq2*dqr3*sin(2*q4))/2 + (dq3*dqr2*sin(2*q4))/2 - (dq3*dqr3*sin(2*q4))/2 + ddqr1*cos(q2)*cos(q3) + ddqr1*sin(q2)*sin(q3) + dq1*dqr2*cos(q2)*sin(q3) - dq1*dqr2*cos(q3)*sin(q2) + dq2*dqr1*cos(q2)*sin(q3) - dq2*dqr1*cos(q3)*sin(q2) - dq1*dqr3*cos(q2)*sin(q3) + dq1*dqr3*cos(q3)*sin(q2) - dq3*dqr1*cos(q2)*sin(q3) + dq3*dqr1*cos(q3)*sin(q2) + dq1*dqr1*cos(q2)^2*cos(q4)*sin(q4) - dq1*dqr2*cos(q2)*cos(q4)^2*sin(q3) + dq1*dqr2*cos(q3)*cos(q4)^2*sin(q2) - dq2*dqr1*cos(q2)*cos(q4)^2*sin(q3) + dq2*dqr1*cos(q3)*cos(q4)^2*sin(q2) + dq1*dqr1*cos(q3)^2*cos(q4)*sin(q4) + dq1*dqr3*cos(q2)*cos(q4)^2*sin(q3) - dq1*dqr3*cos(q3)*cos(q4)^2*sin(q2) + dq3*dqr1*cos(q2)*cos(q4)^2*sin(q3) - dq3*dqr1*cos(q3)*cos(q4)^2*sin(q2) - 2*dq1*dqr1*cos(q2)^2*cos(q3)^2*cos(q4)*sin(q4) - 2*dq1*dqr1*cos(q2)*cos(q3)*cos(q4)*sin(q2)*sin(q3)*sin(q4);
Y4_19_1=(dq2*dqr2*sin(2*q4))/2 + (dq2*dqr2*sin(2*q5))/4 - (dq2*dqr3*sin(2*q4))/2 - (dq3*dqr2*sin(2*q4))/2 - (dq2*dqr3*sin(2*q5))/4 - (dq3*dqr2*sin(2*q5))/4 + (3^(1/2)*dq5*dqr2*sin(q4))/2 - (3^(1/2)*dq5*dqr3*sin(q4))/2 - dq1*dqr1*cos(q2)^2*cos(q4)*sin(q4) + dq1*dqr2*cos(q2)*cos(q4)^2*sin(q3) - dq1*dqr2*cos(q3)*cos(q4)^2*sin(q2) + dq2*dqr1*cos(q2)*cos(q4)^2*sin(q3) - dq2*dqr1*cos(q3)*cos(q4)^2*sin(q2) - dq1*dqr1*cos(q3)^2*cos(q4)*sin(q4) + (dq1*dqr2*cos(q2)*cos(q5)^2*sin(q3))/4 - (dq1*dqr2*cos(q3)*cos(q5)^2*sin(q2))/4 - dq1*dqr3*cos(q2)*cos(q4)^2*sin(q3) + dq1*dqr3*cos(q3)*cos(q4)^2*sin(q2) + (dq2*dqr1*cos(q2)*cos(q5)^2*sin(q3))/4 - (dq2*dqr1*cos(q3)*cos(q5)^2*sin(q2))/4 - dq3*dqr1*cos(q2)*cos(q4)^2*sin(q3) + dq3*dqr1*cos(q3)*cos(q4)^2*sin(q2) - (dq1*dqr1*cos(q2)^2*cos(q5)*sin(q5))/2 - (dq1*dqr3*cos(q2)*cos(q5)^2*sin(q3))/4 + (dq1*dqr3*cos(q3)*cos(q5)^2*sin(q2))/4 - (dq3*dqr1*cos(q2)*cos(q5)^2*sin(q3))/4 + (dq3*dqr1*cos(q3)*cos(q5)^2*sin(q2))/4 - (dq1*dqr1*cos(q3)^2*cos(q5)*sin(q5))/2 - (5*dq2*dqr2*cos(q4)*cos(q5)^2*sin(q4))/4 - dq2*dqr2*cos(q4)^2*cos(q5)*sin(q5) + (5*dq2*dqr3*cos(q4)*cos(q5)^2*sin(q4))/4 + (5*dq3*dqr2*cos(q4)*cos(q5)^2*sin(q4))/4 + dq2*dqr3*cos(q4)^2*cos(q5)*sin(q5) + dq3*dqr2*cos(q4)^2*cos(q5)*sin(q5) - (5*dq3*dqr3*cos(q4)*cos(q5)^2*sin(q4))/4 - dq3*dqr3*cos(q4)^2*cos(q5)*sin(q5) - (3^(1/2)*dq5*dqr2*cos(q5)^2*sin(q4))/2 + (3^(1/2)*dq5*dqr3*cos(q5)^2*sin(q4))/2 + (3^(1/2)*dq5*dqr1*cos(q2)*cos(q4)*sin(q3))/2 - (3^(1/2)*dq5*dqr1*cos(q3)*cos(q4)*sin(q2))/2 - (3^(1/2)*dq5*dqr2*cos(q4)*cos(q5)*sin(q5))/4 + (3^(1/2)*dq5*dqr3*cos(q4)*cos(q5)*sin(q5))/4 + 2*dq1*dqr1*cos(q2)^2*cos(q3)^2*cos(q4)*sin(q4) + (5*dq1*dqr1*cos(q2)^2*cos(q4)*cos(q5)^2*sin(q4))/4 + dq1*dqr1*cos(q2)^2*cos(q3)^2*cos(q5)*sin(q5) - (5*dq1*dqr2*cos(q2)*cos(q4)^2*cos(q5)^2*sin(q3))/4 + (5*dq1*dqr2*cos(q3)*cos(q4)^2*cos(q5)^2*sin(q2))/4 - (5*dq2*dqr1*cos(q2)*cos(q4)^2*cos(q5)^2*sin(q3))/4 + (5*dq2*dqr1*cos(q3)*cos(q4)^2*cos(q5)^2*sin(q2))/4 + dq1*dqr1*cos(q2)^2*cos(q4)^2*cos(q5)*sin(q5) + (5*dq1*dqr1*cos(q3)^2*cos(q4)*cos(q5)^2*sin(q4))/4 + (5*dq1*dqr3*cos(q2)*cos(q4)^2*cos(q5)^2*sin(q3))/4 - (5*dq1*dqr3*cos(q3)*cos(q4)^2*cos(q5)^2*sin(q2))/4 + (5*dq3*dqr1*cos(q2)*cos(q4)^2*cos(q5)^2*sin(q3))/4 - (5*dq3*dqr1*cos(q3)*cos(q4)^2*cos(q5)^2*sin(q2))/4 + dq1*dqr1*cos(q3)^2*cos(q4)^2*cos(q5)*sin(q5) + (3*dq5*dqr1*cos(q2)*cos(q3)*cos(q5)*sin(q5))/4 + (3*dq5*dqr1*cos(q5)*sin(q2)*sin(q3)*sin(q5))/4 + (3^(1/2)*dq1*dqr1*cos(q2)*cos(q4)*cos(q5)^2*sin(q2))/4 - (3^(1/2)*dq1*dqr1*cos(q3)*cos(q4)*cos(q5)^2*sin(q3))/4 + (3^(1/2)*dq1*dqr2*cos(q2)*cos(q3)*cos(q5)^2*sin(q4))/4 + (3^(1/2)*dq2*dqr1*cos(q2)*cos(q3)*cos(q5)^2*sin(q4))/4 - (3^(1/2)*dq1*dqr3*cos(q2)*cos(q3)*cos(q5)^2*sin(q4))/4 - (3^(1/2)*dq3*dqr1*cos(q2)*cos(q3)*cos(q5)^2*sin(q4))/4 - (3^(1/2)*dq5*dqr1*cos(q2)*cos(q4)*cos(q5)^2*sin(q3))/2 + (3^(1/2)*dq5*dqr1*cos(q3)*cos(q4)*cos(q5)^2*sin(q2))/2 + (3^(1/2)*dq1*dqr2*cos(q5)^2*sin(q2)*sin(q3)*sin(q4))/4 + (3^(1/2)*dq2*dqr1*cos(q5)^2*sin(q2)*sin(q3)*sin(q4))/4 - (3^(1/2)*dq1*dqr3*cos(q5)^2*sin(q2)*sin(q3)*sin(q4))/4 - (3^(1/2)*dq3*dqr1*cos(q5)^2*sin(q2)*sin(q3)*sin(q4))/4 - (5*dq1*dqr1*cos(q2)^2*cos(q3)^2*cos(q4)*cos(q5)^2*sin(q4))/2 - 2*dq1*dqr1*cos(q2)^2*cos(q3)^2*cos(q4)^2*cos(q5)*sin(q5) + 2*dq1*dqr1*cos(q2)*cos(q3)*cos(q4)*sin(q2)*sin(q3)*sin(q4) + dq1*dqr1*cos(q2)*cos(q3)*cos(q5)*sin(q2)*sin(q3)*sin(q5) + dq1*dqr2*cos(q2)*cos(q4)*cos(q5)*sin(q3)*sin(q4)*sin(q5) - dq1*dqr2*cos(q3)*cos(q4)*cos(q5)*sin(q2)*sin(q4)*sin(q5) + dq2*dqr1*cos(q2)*cos(q4)*cos(q5)*sin(q3)*sin(q4)*sin(q5) - dq2*dqr1*cos(q3)*cos(q4)*cos(q5)*sin(q2)*sin(q4)*sin(q5) - dq1*dqr3*cos(q2)*cos(q4)*cos(q5)*sin(q3)*sin(q4)*sin(q5) + dq1*dqr3*cos(q3)*cos(q4)*cos(q5)*sin(q2)*sin(q4)*sin(q5) - dq3*dqr1*cos(q2)*cos(q4)*cos(q5)*sin(q3)*sin(q4)*sin(q5) + dq3*dqr1*cos(q3)*cos(q4)*cos(q5)*sin(q2)*sin(q4)*sin(q5) - (3^(1/2)*dq1*dqr1*cos(q2)*cos(q3)^2*cos(q4)*cos(q5)^2*sin(q2))/2 + (3^(1/2)*dq1*dqr1*cos(q2)^2*cos(q3)*cos(q4)*cos(q5)^2*sin(q3))/2 + (3^(1/2)*dq1*dqr2*cos(q2)*cos(q3)*cos(q4)*cos(q5)*sin(q5))/2 + (3^(1/2)*dq2*dqr1*cos(q2)*cos(q3)*cos(q4)*cos(q5)*sin(q5))/2 - (3^(1/2)*dq1*dqr3*cos(q2)*cos(q3)*cos(q4)*cos(q5)*sin(q5))/2 - (3^(1/2)*dq3*dqr1*cos(q2)*cos(q3)*cos(q4)*cos(q5)*sin(q5))/2 - (3^(1/2)*dq1*dqr1*cos(q2)*cos(q5)*sin(q2)*sin(q4)*sin(q5))/2 + (3^(1/2)*dq1*dqr1*cos(q3)*cos(q5)*sin(q3)*sin(q4)*sin(q5))/2 + (3^(1/2)*dq1*dqr2*cos(q4)*cos(q5)*sin(q2)*sin(q3)*sin(q5))/2 + (3^(1/2)*dq2*dqr1*cos(q4)*cos(q5)*sin(q2)*sin(q3)*sin(q5))/2 - (3^(1/2)*dq1*dqr3*cos(q4)*cos(q5)*sin(q2)*sin(q3)*sin(q5))/2 - (3^(1/2)*dq3*dqr1*cos(q4)*cos(q5)*sin(q2)*sin(q3)*sin(q5))/2 + (3^(1/2)*dq5*dqr1*cos(q2)*cos(q5)*sin(q3)*sin(q4)*sin(q5))/4 - (3^(1/2)*dq5*dqr1*cos(q3)*cos(q5)*sin(q2)*sin(q4)*sin(q5))/4 + 3^(1/2)*dq1*dqr1*cos(q2)*cos(q3)^2*cos(q5)*sin(q2)*sin(q4)*sin(q5) - 3^(1/2)*dq1*dqr1*cos(q2)^2*cos(q3)*cos(q5)*sin(q3)*sin(q4)*sin(q5) - (5*dq1*dqr1*cos(q2)*cos(q3)*cos(q4)*cos(q5)^2*sin(q2)*sin(q3)*sin(q4))/2 - 2*dq1*dqr1*cos(q2)*cos(q3)*cos(q4)^2*cos(q5)*sin(q2)*sin(q3)*sin(q5);
Y4_19_2=ddqr4 + ddqr5/2 - (3*ddqr4*cos(q5)^2)/4 + (dq3*dqr3*sin(2*q4))/2 + (dq3*dqr3*sin(2*q5))/4 + (3*dq4*dqr5*sin(2*q5))/8 + (3*dq5*dqr4*sin(2*q5))/8 + ddqr1*cos(q2)*cos(q3) + ddqr1*sin(q2)*sin(q3) + (3^(1/2)*ddqr2*cos(q4)*cos(q5)^2)/4 - (3^(1/2)*ddqr3*cos(q4)*cos(q5)^2)/4 + (3^(1/2)*dq2*dqr5*sin(q4))/2 - (3^(1/2)*dq3*dqr5*sin(q4))/2 - (3*ddqr1*cos(q2)*cos(q3)*cos(q5)^2)/4 - (3*ddqr1*cos(q5)^2*sin(q2)*sin(q3))/4 - (3^(1/2)*dq2*dqr5*cos(q5)^2*sin(q4))/2 + (3^(1/2)*dq3*dqr5*cos(q5)^2*sin(q4))/2 - (3^(1/2)*ddqr2*cos(q5)*sin(q4)*sin(q5))/2 + (3^(1/2)*ddqr3*cos(q5)*sin(q4)*sin(q5))/2 + (3^(1/2)*dq1*dqr5*cos(q2)*cos(q4)*sin(q3))/2 - (3^(1/2)*dq1*dqr5*cos(q3)*cos(q4)*sin(q2))/2 - (3^(1/2)*dq2*dqr5*cos(q4)*cos(q5)*sin(q5))/4 + (3^(1/2)*dq3*dqr5*cos(q4)*cos(q5)*sin(q5))/4 + (3*dq1*dqr5*cos(q2)*cos(q3)*cos(q5)*sin(q5))/4 + (3*dq1*dqr5*cos(q5)*sin(q2)*sin(q3)*sin(q5))/4 - (3^(1/2)*ddqr1*cos(q2)*cos(q5)^2*sin(q3)*sin(q4))/4 + (3^(1/2)*ddqr1*cos(q3)*cos(q5)^2*sin(q2)*sin(q4))/4 - (3^(1/2)*dq1*dqr5*cos(q2)*cos(q4)*cos(q5)^2*sin(q3))/2 + (3^(1/2)*dq1*dqr5*cos(q3)*cos(q4)*cos(q5)^2*sin(q2))/2 - (3^(1/2)*ddqr1*cos(q2)*cos(q4)*cos(q5)*sin(q3)*sin(q5))/2 + (3^(1/2)*ddqr1*cos(q3)*cos(q4)*cos(q5)*sin(q2)*sin(q5))/2 + (3^(1/2)*dq1*dqr5*cos(q2)*cos(q5)*sin(q3)*sin(q4)*sin(q5))/4 - (3^(1/2)*dq1*dqr5*cos(q3)*cos(q5)*sin(q2)*sin(q4)*sin(q5))/4;
Y4_20_1=(3*dq6*dqr1*sin(q2)*sin(q3)*sin(q5))/8 - (3*dq5*dqr1*cos(q6)^2*sin(q2)*sin(q3)*sin(q5))/16 - (3*dq6*dqr1*cos(q6)^2*sin(q2)*sin(q3)*sin(q5))/4 + (3^(1/2)*dq2*dqr1*sin(q2)*sin(q3)*sin(q4))/4 - (3^(1/2)*dq3*dqr1*sin(q2)*sin(q3)*sin(q4))/4 - (3*dq5*dqr1*cos(q5)*sin(q2)*sin(q3)*sin(q5))/4 - (3*dq6*dqr1*cos(q5)*sin(q2)*sin(q3)*sin(q5))/8 - (3*dq5*dqr1*cos(q6)*sin(q2)*sin(q3)*sin(q6))/8 - (9*dq6*dqr1*cos(q6)*sin(q2)*sin(q3)*sin(q6))/16 - (3^(1/2)*dq6*dqr1*cos(q3)*sin(q2)*sin(q4)*sin(q5))/8 - (3^(1/2)*dq2*dqr1*cos(q5)^2*sin(q2)*sin(q3)*sin(q4))/4 - (7*3^(1/2)*dq2*dqr1*cos(q6)^2*sin(q2)*sin(q3)*sin(q4))/16 + (3^(1/2)*dq3*dqr1*cos(q5)^2*sin(q2)*sin(q3)*sin(q4))/4 + (7*3^(1/2)*dq3*dqr1*cos(q6)^2*sin(q2)*sin(q3)*sin(q4))/16 - (3*dq5*dqr1*cos(q5)*cos(q6)*sin(q2)*sin(q3)*sin(q6))/8 - (3*dq6*dqr1*cos(q5)*cos(q6)*sin(q2)*sin(q3)*sin(q6))/8 + (15*dq5*dqr1*cos(q5)*cos(q6)^2*sin(q2)*sin(q3)*sin(q5))/16 + (3*dq5*dqr1*cos(q5)^2*cos(q6)*sin(q2)*sin(q3)*sin(q6))/4 + (3*dq6*dqr1*cos(q5)*cos(q6)^2*sin(q2)*sin(q3)*sin(q5))/4 + (15*dq6*dqr1*cos(q5)^2*cos(q6)*sin(q2)*sin(q3)*sin(q6))/16 + (3^(1/2)*dq1*dqr1*cos(q2)*cos(q6)^2*sin(q2)*sin(q4)*sin(q5))/8 - (3^(1/2)*dq2*dqr1*cos(q4)*cos(q6)^2*sin(q2)*sin(q3)*sin(q5))/8 + (3^(1/2)*dq2*dqr1*cos(q5)*cos(q6)^2*sin(q2)*sin(q3)*sin(q4))/8 + (3^(1/2)*dq3*dqr1*cos(q4)*cos(q6)^2*sin(q2)*sin(q3)*sin(q5))/8 - (3^(1/2)*dq3*dqr1*cos(q5)*cos(q6)^2*sin(q2)*sin(q3)*sin(q4))/8 - (3*3^(1/2)*dq5*dqr1*cos(q3)*cos(q6)^2*sin(q2)*sin(q4)*sin(q5))/16 - (3^(1/2)*dq6*dqr1*cos(q3)*cos(q6)^2*sin(q2)*sin(q4)*sin(q5))/4 - (dq1*dqr1*cos(q2)*cos(q3)*cos(q4)*sin(q2)*sin(q3)*sin(q4))/2 - dq1*dqr1*cos(q2)*cos(q3)*cos(q5)*sin(q2)*sin(q3)*sin(q5) - (dq1*dqr1*cos(q2)*cos(q3)*cos(q6)*sin(q2)*sin(q3)*sin(q6))/2 + dq2*dqr1*cos(q3)*cos(q4)*cos(q5)*sin(q2)*sin(q4)*sin(q5) - dq3*dqr1*cos(q3)*cos(q4)*cos(q5)*sin(q2)*sin(q4)*sin(q5) + (dq2*dqr1*cos(q3)*cos(q4)*cos(q6)*sin(q2)*sin(q4)*sin(q6))/2 - (dq3*dqr1*cos(q3)*cos(q4)*cos(q6)*sin(q2)*sin(q4)*sin(q6))/2 + (5*3^(1/2)*dq2*dqr1*cos(q5)^2*cos(q6)^2*sin(q2)*sin(q3)*sin(q4))/16 - (5*3^(1/2)*dq3*dqr1*cos(q5)^2*cos(q6)^2*sin(q2)*sin(q3)*sin(q4))/16 + (3*dq1*dqr1*cos(q2)*cos(q3)*cos(q6)^2*sin(q2)*sin(q3)*sin(q5))/4 - (3*dq2*dqr1*cos(q3)*cos(q4)*cos(q6)^2*sin(q2)*sin(q4)*sin(q5))/4 + (3*dq3*dqr1*cos(q3)*cos(q4)*cos(q6)^2*sin(q2)*sin(q4)*sin(q5))/4 + (3^(1/2)*dq1*dqr1*cos(q2)*cos(q5)*sin(q2)*sin(q4)*sin(q5))/2 + (3^(1/2)*dq1*dqr1*cos(q2)*cos(q6)*sin(q2)*sin(q4)*sin(q6))/4 - (3^(1/2)*dq2*dqr1*cos(q4)*cos(q5)*sin(q2)*sin(q3)*sin(q5))/2 + (3^(1/2)*dq3*dqr1*cos(q4)*cos(q5)*sin(q2)*sin(q3)*sin(q5))/2 - (3^(1/2)*dq2*dqr1*cos(q4)*cos(q6)*sin(q2)*sin(q3)*sin(q6))/4 + (3^(1/2)*dq3*dqr1*cos(q4)*cos(q6)*sin(q2)*sin(q3)*sin(q6))/4 + (3^(1/2)*dq5*dqr1*cos(q3)*cos(q5)*sin(q2)*sin(q4)*sin(q5))/4 + (3^(1/2)*dq6*dqr1*cos(q3)*cos(q5)*sin(q2)*sin(q4)*sin(q5))/8 + (3^(1/2)*dq5*dqr1*cos(q3)*cos(q6)*sin(q2)*sin(q4)*sin(q6))/8 + (7*3^(1/2)*dq6*dqr1*cos(q3)*cos(q6)*sin(q2)*sin(q4)*sin(q6))/16 - 3^(1/2)*dq1*dqr1*cos(q2)*cos(q3)^2*cos(q5)*sin(q2)*sin(q4)*sin(q5) - (3^(1/2)*dq1*dqr1*cos(q2)*cos(q3)^2*cos(q6)*sin(q2)*sin(q4)*sin(q6))/2 - (5*3^(1/2)*dq1*dqr1*cos(q2)*cos(q5)*cos(q6)^2*sin(q2)*sin(q4)*sin(q5))/8 - (3^(1/2)*dq1*dqr1*cos(q2)*cos(q5)^2*cos(q6)*sin(q2)*sin(q4)*sin(q6))/2 + (5*3^(1/2)*dq2*dqr1*cos(q4)*cos(q5)*cos(q6)^2*sin(q2)*sin(q3)*sin(q5))/8 + (3^(1/2)*dq2*dqr1*cos(q4)*cos(q5)^2*cos(q6)*sin(q2)*sin(q3)*sin(q6))/2 - (5*3^(1/2)*dq3*dqr1*cos(q4)*cos(q5)*cos(q6)^2*sin(q2)*sin(q3)*sin(q5))/8 - (3^(1/2)*dq3*dqr1*cos(q4)*cos(q5)^2*cos(q6)*sin(q2)*sin(q3)*sin(q6))/2 - (5*3^(1/2)*dq5*dqr1*cos(q3)*cos(q5)*cos(q6)^2*sin(q2)*sin(q4)*sin(q5))/16 - (3^(1/2)*dq5*dqr1*cos(q3)*cos(q5)^2*cos(q6)*sin(q2)*sin(q4)*sin(q6))/4 - (3^(1/2)*dq6*dqr1*cos(q3)*cos(q5)*cos(q6)^2*sin(q2)*sin(q4)*sin(q5))/4 - (5*3^(1/2)*dq6*dqr1*cos(q3)*cos(q5)^2*cos(q6)*sin(q2)*sin(q4)*sin(q6))/16 + (3*dq1*dqr1*cos(q2)*cos(q3)*cos(q5)*cos(q6)*sin(q2)*sin(q3)*sin(q6))/2 - (3*dq2*dqr1*cos(q3)*cos(q4)*cos(q5)*cos(q6)*sin(q2)*sin(q4)*sin(q6))/2 + (3*dq3*dqr1*cos(q3)*cos(q4)*cos(q5)*cos(q6)*sin(q2)*sin(q4)*sin(q6))/2 - (3^(1/2)*dq1*dqr1*cos(q2)*cos(q3)^2*cos(q6)^2*sin(q2)*sin(q4)*sin(q5))/4 + (5*dq1*dqr1*cos(q2)*cos(q3)*cos(q4)*cos(q5)^2*sin(q2)*sin(q3)*sin(q4))/2 - (dq1*dqr1*cos(q2)*cos(q3)*cos(q4)*cos(q6)^2*sin(q2)*sin(q3)*sin(q4))/8 + 2*dq1*dqr1*cos(q2)*cos(q3)*cos(q4)^2*cos(q5)*sin(q2)*sin(q3)*sin(q5) + (5*dq1*dqr1*cos(q2)*cos(q3)*cos(q5)*cos(q6)^2*sin(q2)*sin(q3)*sin(q5))/4 + dq1*dqr1*cos(q2)*cos(q3)*cos(q4)^2*cos(q6)*sin(q2)*sin(q3)*sin(q6) + dq1*dqr1*cos(q2)*cos(q3)*cos(q5)^2*cos(q6)*sin(q2)*sin(q3)*sin(q6) - (5*dq2*dqr1*cos(q3)*cos(q4)*cos(q5)*cos(q6)^2*sin(q2)*sin(q4)*sin(q5))/4 - dq2*dqr1*cos(q3)*cos(q4)*cos(q5)^2*cos(q6)*sin(q2)*sin(q4)*sin(q6) + (5*dq3*dqr1*cos(q3)*cos(q4)*cos(q5)*cos(q6)^2*sin(q2)*sin(q4)*sin(q5))/4 - (5*dq2*dqr1*cos(q3)*cos(q4)^2*cos(q5)*cos(q6)*sin(q2)*sin(q5)*sin(q6))/4 + dq3*dqr1*cos(q3)*cos(q4)*cos(q5)^2*cos(q6)*sin(q2)*sin(q4)*sin(q6) - (3^(1/2)*dq1*dqr1*cos(q2)*cos(q4)*cos(q6)*sin(q2)*sin(q5)*sin(q6))/4 + (3^(1/2)*dq1*dqr1*cos(q2)*cos(q5)*cos(q6)*sin(q2)*sin(q4)*sin(q6))/4 - (3^(1/2)*dq2*dqr1*cos(q4)*cos(q5)*cos(q6)*sin(q2)*sin(q3)*sin(q6))/4 + (3^(1/2)*dq3*dqr1*cos(q4)*cos(q5)*cos(q6)*sin(q2)*sin(q3)*sin(q6))/4 - (3*3^(1/2)*dq5*dqr1*cos(q3)*cos(q5)*cos(q6)*sin(q2)*sin(q4)*sin(q6))/8 - (3^(1/2)*dq6*dqr1*cos(q3)*cos(q5)*cos(q6)*sin(q2)*sin(q4)*sin(q6))/8 - (3^(1/2)*dq2*dqr1*cos(q6)*sin(q2)*sin(q3)*sin(q4)*sin(q5)*sin(q6))/4 + (3^(1/2)*dq3*dqr1*cos(q6)*sin(q2)*sin(q3)*sin(q4)*sin(q5)*sin(q6))/4 - (3*dq1*dqr1*cos(q2)*cos(q3)*cos(q4)^2*cos(q6)^2*sin(q2)*sin(q3)*sin(q5))/2 + (5*3^(1/2)*dq1*dqr1*cos(q2)*cos(q3)^2*cos(q5)*cos(q6)^2*sin(q2)*sin(q4)*sin(q5))/4 + 3^(1/2)*dq1*dqr1*cos(q2)*cos(q3)^2*cos(q5)^2*cos(q6)*sin(q2)*sin(q4)*sin(q6) - (3*dq1*dqr1*cos(q2)*cos(q3)*cos(q4)*cos(q5)*cos(q6)^2*sin(q2)*sin(q3)*sin(q4))/4 - 3*dq1*dqr1*cos(q2)*cos(q3)*cos(q4)^2*cos(q5)*cos(q6)*sin(q2)*sin(q3)*sin(q6) - (3^(1/2)*dq1*dqr1*cos(q2)*cos(q4)*cos(q5)*cos(q6)*sin(q2)*sin(q5)*sin(q6))/4 - (3^(1/2)*dq2*dqr1*cos(q5)*cos(q6)*sin(q2)*sin(q3)*sin(q4)*sin(q5)*sin(q6))/4 + (3^(1/2)*dq3*dqr1*cos(q5)*cos(q6)*sin(q2)*sin(q3)*sin(q4)*sin(q5)*sin(q6))/4 - (25*dq1*dqr1*cos(q2)*cos(q3)*cos(q4)*cos(q5)^2*cos(q6)^2*sin(q2)*sin(q3)*sin(q4))/8 - (5*dq1*dqr1*cos(q2)*cos(q3)*cos(q4)^2*cos(q5)*cos(q6)^2*sin(q2)*sin(q3)*sin(q5))/2 - 2*dq1*dqr1*cos(q2)*cos(q3)*cos(q4)^2*cos(q5)^2*cos(q6)*sin(q2)*sin(q3)*sin(q6) + (3^(1/2)*dq1*dqr1*cos(q2)*cos(q3)^2*cos(q4)*cos(q6)*sin(q2)*sin(q5)*sin(q6))/2 - (3^(1/2)*dq1*dqr1*cos(q2)*cos(q3)^2*cos(q5)*cos(q6)*sin(q2)*sin(q4)*sin(q6))/2 + (3^(1/2)*dq1*dqr1*cos(q2)*cos(q3)^2*cos(q4)*cos(q5)*cos(q6)*sin(q2)*sin(q5)*sin(q6))/2 + (3*dq1*dqr1*cos(q2)*cos(q3)*cos(q4)*cos(q6)*sin(q2)*sin(q3)*sin(q4)*sin(q5)*sin(q6))/2 + (5*dq1*dqr1*cos(q2)*cos(q3)*cos(q4)*cos(q5)*cos(q6)*sin(q2)*sin(q3)*sin(q4)*sin(q5)*sin(q6))/2;
Y4_20_2=(dq3*dqr1*cos(q3)*sin(q2))/4 - (dq2*dqr1*cos(q3)*sin(q2))/4 + (dq2*dqr1*cos(q3)*cos(q4)^2*sin(q2))/4 + (dq2*dqr1*cos(q3)*cos(q5)^2*sin(q2))/4 - (dq3*dqr1*cos(q3)*cos(q4)^2*sin(q2))/4 - (5*dq2*dqr1*cos(q3)*cos(q6)^2*sin(q2))/16 - (dq3*dqr1*cos(q3)*cos(q5)^2*sin(q2))/4 + (5*dq3*dqr1*cos(q3)*cos(q6)^2*sin(q2))/16 + (3^(1/2)*dq1*dqr1*cos(q2)*cos(q4)*sin(q2))/4 - (5*dq2*dqr1*cos(q3)*cos(q4)^2*cos(q5)^2*sin(q2))/4 + (dq2*dqr1*cos(q3)*cos(q4)^2*cos(q6)^2*sin(q2))/16 + (5*dq3*dqr1*cos(q3)*cos(q4)^2*cos(q5)^2*sin(q2))/4 - (5*dq2*dqr1*cos(q3)*cos(q5)^2*cos(q6)^2*sin(q2))/16 - (dq3*dqr1*cos(q3)*cos(q4)^2*cos(q6)^2*sin(q2))/16 + (5*dq3*dqr1*cos(q3)*cos(q5)^2*cos(q6)^2*sin(q2))/16 - (3*dq2*dqr1*cos(q3)*cos(q5)*cos(q6)^2*sin(q2))/8 + (3*dq3*dqr1*cos(q3)*cos(q5)*cos(q6)^2*sin(q2))/8 + (3^(1/2)*dq6*dqr1*cos(q2)*sin(q3)*sin(q4)*sin(q5))/8 + (3*dq2*dqr1*cos(q3)*cos(q4)^2*cos(q5)*cos(q6)^2*sin(q2))/8 - (3*dq3*dqr1*cos(q3)*cos(q4)^2*cos(q5)*cos(q6)^2*sin(q2))/8 - (3^(1/2)*dq1*dqr1*cos(q2)*cos(q3)^2*cos(q4)*sin(q2))/2 - (3^(1/2)*dq1*dqr1*cos(q2)*cos(q4)*cos(q5)^2*sin(q2))/4 - (7*3^(1/2)*dq1*dqr1*cos(q2)*cos(q4)*cos(q6)^2*sin(q2))/16 - (3^(1/2)*dq5*dqr1*cos(q3)*cos(q4)*cos(q5)^2*sin(q2))/2 - (3^(1/2)*dq5*dqr1*cos(q3)*cos(q4)*cos(q6)^2*sin(q2))/8 - (3^(1/2)*dq6*dqr1*cos(q3)*cos(q4)*cos(q5)^2*sin(q2))/4 - (3^(1/2)*dq6*dqr1*cos(q3)*cos(q4)*cos(q6)^2*sin(q2))/4 + (25*dq2*dqr1*cos(q3)*cos(q4)^2*cos(q5)^2*cos(q6)^2*sin(q2))/16 - (25*dq3*dqr1*cos(q3)*cos(q4)^2*cos(q5)^2*cos(q6)^2*sin(q2))/16 - (3*dq2*dqr1*cos(q2)*cos(q6)*sin(q3)*sin(q5)*sin(q6))/4 + (3*dq2*dqr1*cos(q3)*cos(q6)*sin(q2)*sin(q5)*sin(q6))/4 + (3*dq3*dqr1*cos(q2)*cos(q6)*sin(q3)*sin(q5)*sin(q6))/4 - (3*dq3*dqr1*cos(q3)*cos(q6)*sin(q2)*sin(q5)*sin(q6))/4 + (3^(1/2)*dq6*dqr1*cos(q3)*cos(q4)*cos(q5)*sin(q2))/4 + (3^(1/2)*dq1*dqr1*cos(q2)*cos(q4)*cos(q5)*cos(q6)^2*sin(q2))/8 - (3^(1/2)*dq6*dqr1*cos(q3)*cos(q4)*cos(q5)*cos(q6)^2*sin(q2))/4 - (3^(1/2)*dq1*dqr1*cos(q3)*cos(q6)^2*sin(q3)*sin(q4)*sin(q5))/8 + (3*3^(1/2)*dq5*dqr1*cos(q2)*cos(q6)^2*sin(q3)*sin(q4)*sin(q5))/16 + (3^(1/2)*dq6*dqr1*cos(q2)*cos(q6)^2*sin(q3)*sin(q4)*sin(q5))/4 - dq2*dqr1*cos(q2)*cos(q4)*cos(q5)*sin(q3)*sin(q4)*sin(q5) + dq3*dqr1*cos(q2)*cos(q4)*cos(q5)*sin(q3)*sin(q4)*sin(q5) - (dq2*dqr1*cos(q2)*cos(q4)*cos(q6)*sin(q3)*sin(q4)*sin(q6))/2 + (dq3*dqr1*cos(q2)*cos(q4)*cos(q6)*sin(q3)*sin(q4)*sin(q6))/2 - (dq2*dqr1*cos(q2)*cos(q5)*cos(q6)*sin(q3)*sin(q5)*sin(q6))/4 + (dq2*dqr1*cos(q3)*cos(q5)*cos(q6)*sin(q2)*sin(q5)*sin(q6))/4 + (dq3*dqr1*cos(q2)*cos(q5)*cos(q6)*sin(q3)*sin(q5)*sin(q6))/4 - (dq3*dqr1*cos(q3)*cos(q5)*cos(q6)*sin(q2)*sin(q5)*sin(q6))/4 + (3^(1/2)*dq1*dqr1*cos(q2)*cos(q3)^2*cos(q4)*cos(q5)^2*sin(q2))/2 + (7*3^(1/2)*dq1*dqr1*cos(q2)*cos(q3)^2*cos(q4)*cos(q6)^2*sin(q2))/8 + (5*3^(1/2)*dq1*dqr1*cos(q2)*cos(q4)*cos(q5)^2*cos(q6)^2*sin(q2))/16 + (5*3^(1/2)*dq5*dqr1*cos(q3)*cos(q4)*cos(q5)^2*cos(q6)^2*sin(q2))/8 + (3^(1/2)*dq6*dqr1*cos(q3)*cos(q4)*cos(q5)^2*cos(q6)^2*sin(q2))/2 + (3*dq2*dqr1*cos(q2)*cos(q4)*cos(q6)^2*sin(q3)*sin(q4)*sin(q5))/4 - (3*dq3*dqr1*cos(q2)*cos(q4)*cos(q6)^2*sin(q3)*sin(q4)*sin(q5))/4 + (3*dq2*dqr1*cos(q2)*cos(q4)^2*cos(q6)*sin(q3)*sin(q5)*sin(q6))/4 - (3*dq2*dqr1*cos(q3)*cos(q4)^2*cos(q6)*sin(q2)*sin(q5)*sin(q6))/4 - (3*dq3*dqr1*cos(q2)*cos(q4)^2*cos(q6)*sin(q3)*sin(q5)*sin(q6))/4 + (3*dq3*dqr1*cos(q3)*cos(q4)^2*cos(q6)*sin(q2)*sin(q5)*sin(q6))/4 - (3^(1/2)*dq1*dqr1*cos(q3)*cos(q5)*sin(q3)*sin(q4)*sin(q5))/2 - (3^(1/2)*dq1*dqr1*cos(q3)*cos(q6)*sin(q3)*sin(q4)*sin(q6))/4 - (3^(1/2)*dq5*dqr1*cos(q2)*cos(q5)*sin(q3)*sin(q4)*sin(q5))/4 - (3^(1/2)*dq6*dqr1*cos(q2)*cos(q5)*sin(q3)*sin(q4)*sin(q5))/8 - (3^(1/2)*dq5*dqr1*cos(q2)*cos(q6)*sin(q3)*sin(q4)*sin(q6))/8 - (7*3^(1/2)*dq6*dqr1*cos(q2)*cos(q6)*sin(q3)*sin(q4)*sin(q6))/16 + 3^(1/2)*dq1*dqr1*cos(q2)^2*cos(q3)*cos(q5)*sin(q3)*sin(q4)*sin(q5) + (3^(1/2)*dq1*dqr1*cos(q2)^2*cos(q3)*cos(q6)*sin(q3)*sin(q4)*sin(q6))/2 + (5*3^(1/2)*dq1*dqr1*cos(q3)*cos(q5)*cos(q6)^2*sin(q3)*sin(q4)*sin(q5))/8 + (3^(1/2)*dq1*dqr1*cos(q3)*cos(q5)^2*cos(q6)*sin(q3)*sin(q4)*sin(q6))/2 + (5*3^(1/2)*dq5*dqr1*cos(q2)*cos(q5)*cos(q6)^2*sin(q3)*sin(q4)*sin(q5))/16 + (3^(1/2)*dq5*dqr1*cos(q2)*cos(q5)^2*cos(q6)*sin(q3)*sin(q4)*sin(q6))/4 + (3^(1/2)*dq6*dqr1*cos(q2)*cos(q5)*cos(q6)^2*sin(q3)*sin(q4)*sin(q5))/4 + (5*3^(1/2)*dq6*dqr1*cos(q2)*cos(q5)^2*cos(q6)*sin(q3)*sin(q4)*sin(q6))/16 + (3*dq2*dqr1*cos(q2)*cos(q4)*cos(q5)*cos(q6)*sin(q3)*sin(q4)*sin(q6))/2 - (3*dq3*dqr1*cos(q2)*cos(q4)*cos(q5)*cos(q6)*sin(q3)*sin(q4)*sin(q6))/2 - (3^(1/2)*dq1*dqr1*cos(q2)*cos(q3)^2*cos(q4)*cos(q5)*cos(q6)^2*sin(q2))/4 + (3^(1/2)*dq1*dqr1*cos(q2)^2*cos(q3)*cos(q6)^2*sin(q3)*sin(q4)*sin(q5))/4 + (5*dq2*dqr1*cos(q2)*cos(q4)*cos(q5)*cos(q6)^2*sin(q3)*sin(q4)*sin(q5))/4 + dq2*dqr1*cos(q2)*cos(q4)*cos(q5)^2*cos(q6)*sin(q3)*sin(q4)*sin(q6) - (5*dq3*dqr1*cos(q2)*cos(q4)*cos(q5)*cos(q6)^2*sin(q3)*sin(q4)*sin(q5))/4 + (5*dq2*dqr1*cos(q2)*cos(q4)^2*cos(q5)*cos(q6)*sin(q3)*sin(q5)*sin(q6))/4 - dq3*dqr1*cos(q2)*cos(q4)*cos(q5)^2*cos(q6)*sin(q3)*sin(q4)*sin(q6) - (5*dq3*dqr1*cos(q2)*cos(q4)^2*cos(q5)*cos(q6)*sin(q3)*sin(q5)*sin(q6))/4 + (5*dq3*dqr1*cos(q3)*cos(q4)^2*cos(q5)*cos(q6)*sin(q2)*sin(q5)*sin(q6))/4 - (5*3^(1/2)*dq1*dqr1*cos(q2)*cos(q3)^2*cos(q4)*cos(q5)^2*cos(q6)^2*sin(q2))/8 + (3^(1/2)*dq1*dqr1*cos(q3)*cos(q4)*cos(q6)*sin(q3)*sin(q5)*sin(q6))/4 - (3^(1/2)*dq1*dqr1*cos(q3)*cos(q5)*cos(q6)*sin(q3)*sin(q4)*sin(q6))/4 + (3*3^(1/2)*dq5*dqr1*cos(q2)*cos(q5)*cos(q6)*sin(q3)*sin(q4)*sin(q6))/8 - (3^(1/2)*dq6*dqr1*cos(q2)*cos(q4)*cos(q6)*sin(q3)*sin(q5)*sin(q6))/8 + (3^(1/2)*dq6*dqr1*cos(q2)*cos(q5)*cos(q6)*sin(q3)*sin(q4)*sin(q6))/8 + (3^(1/2)*dq6*dqr1*cos(q3)*cos(q4)*cos(q6)*sin(q2)*sin(q5)*sin(q6))/8 - (5*3^(1/2)*dq1*dqr1*cos(q2)^2*cos(q3)*cos(q5)*cos(q6)^2*sin(q3)*sin(q4)*sin(q5))/4 - 3^(1/2)*dq1*dqr1*cos(q2)^2*cos(q3)*cos(q5)^2*cos(q6)*sin(q3)*sin(q4)*sin(q6) + (3^(1/2)*dq1*dqr1*cos(q3)*cos(q4)*cos(q5)*cos(q6)*sin(q3)*sin(q5)*sin(q6))/4 + (3^(1/2)*dq5*dqr1*cos(q2)*cos(q4)*cos(q5)*cos(q6)*sin(q3)*sin(q5)*sin(q6))/2 - (3^(1/2)*dq5*dqr1*cos(q3)*cos(q4)*cos(q5)*cos(q6)*sin(q2)*sin(q5)*sin(q6))/2 + (5*3^(1/2)*dq6*dqr1*cos(q2)*cos(q4)*cos(q5)*cos(q6)*sin(q3)*sin(q5)*sin(q6))/8 - (5*3^(1/2)*dq6*dqr1*cos(q3)*cos(q4)*cos(q5)*cos(q6)*sin(q2)*sin(q5)*sin(q6))/8 - (3^(1/2)*dq1*dqr1*cos(q2)^2*cos(q3)*cos(q4)*cos(q6)*sin(q3)*sin(q5)*sin(q6))/2 + (3^(1/2)*dq1*dqr1*cos(q2)^2*cos(q3)*cos(q5)*cos(q6)*sin(q3)*sin(q4)*sin(q6))/2 - (3^(1/2)*dq1*dqr1*cos(q2)^2*cos(q3)*cos(q4)*cos(q5)*cos(q6)*sin(q3)*sin(q5)*sin(q6))/2;
Y4_20_3=(dq2*dqr1*cos(q2)*sin(q3))/4 - (dq3*dqr1*cos(q2)*sin(q3))/4 + (dq1*dqr1*cos(q2)^2*cos(q4)*sin(q4))/4 - (dq2*dqr1*cos(q2)*cos(q4)^2*sin(q3))/4 + (dq1*dqr1*cos(q3)^2*cos(q4)*sin(q4))/4 - (dq2*dqr1*cos(q2)*cos(q5)^2*sin(q3))/4 + (dq3*dqr1*cos(q2)*cos(q4)^2*sin(q3))/4 + (dq1*dqr1*cos(q2)^2*cos(q5)*sin(q5))/2 + (5*dq2*dqr1*cos(q2)*cos(q6)^2*sin(q3))/16 + (dq3*dqr1*cos(q2)*cos(q5)^2*sin(q3))/4 - (5*dq3*dqr1*cos(q2)*cos(q6)^2*sin(q3))/16 - (3*dq1*dqr1*cos(q2)^2*cos(q6)^2*sin(q5))/8 + (3*dq6*dqr1*cos(q2)*cos(q3)*sin(q5))/8 - (3^(1/2)*dq1*dqr1*cos(q3)*cos(q4)*sin(q3))/4 + (3^(1/2)*dq2*dqr1*cos(q2)*cos(q3)*sin(q4))/4 - (3^(1/2)*dq3*dqr1*cos(q2)*cos(q3)*sin(q4))/4 - (dq1*dqr1*cos(q2)^2*cos(q3)^2*cos(q4)*sin(q4))/2 - (5*dq1*dqr1*cos(q2)^2*cos(q4)*cos(q5)^2*sin(q4))/4 - dq1*dqr1*cos(q2)^2*cos(q3)^2*cos(q5)*sin(q5) + (5*dq2*dqr1*cos(q2)*cos(q4)^2*cos(q5)^2*sin(q3))/4 + (dq1*dqr1*cos(q2)^2*cos(q4)*cos(q6)^2*sin(q4))/16 - dq1*dqr1*cos(q2)^2*cos(q4)^2*cos(q5)*sin(q5) - (5*dq1*dqr1*cos(q3)^2*cos(q4)*cos(q5)^2*sin(q4))/4 - (dq2*dqr1*cos(q2)*cos(q4)^2*cos(q6)^2*sin(q3))/16 - (5*dq3*dqr1*cos(q2)*cos(q4)^2*cos(q5)^2*sin(q3))/4 + (dq1*dqr1*cos(q3)^2*cos(q4)*cos(q6)^2*sin(q4))/16 - dq1*dqr1*cos(q3)^2*cos(q4)^2*cos(q5)*sin(q5) + (5*dq2*dqr1*cos(q2)*cos(q5)^2*cos(q6)^2*sin(q3))/16 + (dq3*dqr1*cos(q2)*cos(q4)^2*cos(q6)^2*sin(q3))/16 - (5*dq1*dqr1*cos(q2)^2*cos(q5)*cos(q6)^2*sin(q5))/8 - (5*dq3*dqr1*cos(q2)*cos(q5)^2*cos(q6)^2*sin(q3))/16 - (3*dq5*dqr1*cos(q2)*cos(q3)*cos(q5)*sin(q5))/4 - (3*dq6*dqr1*cos(q2)*cos(q3)*cos(q5)*sin(q5))/8 + (3*dq1*dqr1*cos(q2)^2*cos(q3)^2*cos(q6)^2*sin(q5))/4 + (3*dq1*dqr1*cos(q2)^2*cos(q4)^2*cos(q6)^2*sin(q5))/4 + (3*dq2*dqr1*cos(q2)*cos(q5)*cos(q6)^2*sin(q3))/8 - (3*dq3*dqr1*cos(q2)*cos(q5)*cos(q6)^2*sin(q3))/8 - (3*dq5*dqr1*cos(q2)*cos(q3)*cos(q6)^2*sin(q5))/16 - (3*dq6*dqr1*cos(q2)*cos(q3)*cos(q6)^2*sin(q5))/4 + (3*dq1*dqr1*cos(q2)^2*cos(q4)*cos(q5)*cos(q6)^2*sin(q4))/8 - (3*dq2*dqr1*cos(q2)*cos(q4)^2*cos(q5)*cos(q6)^2*sin(q3))/8 + (3*dq1*dqr1*cos(q3)^2*cos(q4)*cos(q5)*cos(q6)^2*sin(q4))/8 + (3*dq3*dqr1*cos(q2)*cos(q4)^2*cos(q5)*cos(q6)^2*sin(q3))/8 + (3^(1/2)*dq1*dqr1*cos(q2)^2*cos(q3)*cos(q4)*sin(q3))/2 + (3^(1/2)*dq1*dqr1*cos(q3)*cos(q4)*cos(q5)^2*sin(q3))/4 - (3^(1/2)*dq2*dqr1*cos(q2)*cos(q3)*cos(q5)^2*sin(q4))/4 + (7*3^(1/2)*dq1*dqr1*cos(q3)*cos(q4)*cos(q6)^2*sin(q3))/16 - (7*3^(1/2)*dq2*dqr1*cos(q2)*cos(q3)*cos(q6)^2*sin(q4))/16 + (3^(1/2)*dq3*dqr1*cos(q2)*cos(q3)*cos(q5)^2*sin(q4))/4 + (7*3^(1/2)*dq3*dqr1*cos(q2)*cos(q3)*cos(q6)^2*sin(q4))/16 + (3^(1/2)*dq5*dqr1*cos(q2)*cos(q4)*cos(q5)^2*sin(q3))/2 + (3^(1/2)*dq5*dqr1*cos(q2)*cos(q4)*cos(q6)^2*sin(q3))/8 + (3^(1/2)*dq6*dqr1*cos(q2)*cos(q4)*cos(q5)^2*sin(q3))/4 + (3^(1/2)*dq6*dqr1*cos(q2)*cos(q4)*cos(q6)^2*sin(q3))/4 + (5*dq1*dqr1*cos(q2)^2*cos(q3)^2*cos(q4)*cos(q5)^2*sin(q4))/2 - (dq1*dqr1*cos(q2)^2*cos(q3)^2*cos(q4)*cos(q6)^2*sin(q4))/8 + 2*dq1*dqr1*cos(q2)^2*cos(q3)^2*cos(q4)^2*cos(q5)*sin(q5) + (25*dq1*dqr1*cos(q2)^2*cos(q4)*cos(q5)^2*cos(q6)^2*sin(q4))/16 + (5*dq1*dqr1*cos(q2)^2*cos(q3)^2*cos(q5)*cos(q6)^2*sin(q5))/4 - (25*dq2*dqr1*cos(q2)*cos(q4)^2*cos(q5)^2*cos(q6)^2*sin(q3))/16 + (5*dq1*dqr1*cos(q2)^2*cos(q4)^2*cos(q5)*cos(q6)^2*sin(q5))/4 + (25*dq1*dqr1*cos(q3)^2*cos(q4)*cos(q5)^2*cos(q6)^2*sin(q4))/16 + (25*dq3*dqr1*cos(q2)*cos(q4)^2*cos(q5)^2*cos(q6)^2*sin(q3))/16 + (5*dq1*dqr1*cos(q3)^2*cos(q4)^2*cos(q5)*cos(q6)^2*sin(q5))/4 + (15*dq5*dqr1*cos(q2)*cos(q3)*cos(q5)*cos(q6)^2*sin(q5))/16 + (3*dq6*dqr1*cos(q2)*cos(q3)*cos(q5)*cos(q6)^2*sin(q5))/4 - (3*dq1*dqr1*cos(q2)^2*cos(q3)^2*cos(q4)^2*cos(q6)^2*sin(q5))/2 - (3^(1/2)*dq6*dqr1*cos(q2)*cos(q4)*cos(q5)*sin(q3))/4 - (3^(1/2)*dq1*dqr1*cos(q3)*cos(q4)*cos(q5)*cos(q6)^2*sin(q3))/8 - (3^(1/2)*dq2*dqr1*cos(q2)*cos(q3)*cos(q4)*cos(q6)^2*sin(q5))/8 + (3^(1/2)*dq2*dqr1*cos(q2)*cos(q3)*cos(q5)*cos(q6)^2*sin(q4))/8 + (3^(1/2)*dq3*dqr1*cos(q2)*cos(q3)*cos(q4)*cos(q6)^2*sin(q5))/8 - (3^(1/2)*dq3*dqr1*cos(q2)*cos(q3)*cos(q5)*cos(q6)^2*sin(q4))/8 + (3^(1/2)*dq6*dqr1*cos(q2)*cos(q4)*cos(q5)*cos(q6)^2*sin(q3))/4 - (3*dq1*dqr1*cos(q2)^2*cos(q3)^2*cos(q4)*cos(q5)*cos(q6)^2*sin(q4))/4 - (3^(1/2)*dq1*dqr1*cos(q2)^2*cos(q3)*cos(q4)*cos(q5)^2*sin(q3))/2 - (7*3^(1/2)*dq1*dqr1*cos(q2)^2*cos(q3)*cos(q4)*cos(q6)^2*sin(q3))/8 - (5*3^(1/2)*dq1*dqr1*cos(q3)*cos(q4)*cos(q5)^2*cos(q6)^2*sin(q3))/16 + (5*3^(1/2)*dq2*dqr1*cos(q2)*cos(q3)*cos(q5)^2*cos(q6)^2*sin(q4))/16 - (5*3^(1/2)*dq3*dqr1*cos(q2)*cos(q3)*cos(q5)^2*cos(q6)^2*sin(q4))/16 - (5*3^(1/2)*dq5*dqr1*cos(q2)*cos(q4)*cos(q5)^2*cos(q6)^2*sin(q3))/8 - (3^(1/2)*dq6*dqr1*cos(q2)*cos(q4)*cos(q5)^2*cos(q6)^2*sin(q3))/2 - (25*dq1*dqr1*cos(q2)^2*cos(q3)^2*cos(q4)*cos(q5)^2*cos(q6)^2*sin(q4))/8 - (5*dq1*dqr1*cos(q2)^2*cos(q3)^2*cos(q4)^2*cos(q5)*cos(q6)^2*sin(q5))/2 - (3*dq1*dqr1*cos(q2)^2*cos(q4)*cos(q6)*sin(q4)*sin(q5)*sin(q6))/4 - (3*dq1*dqr1*cos(q3)^2*cos(q4)*cos(q6)*sin(q4)*sin(q5)*sin(q6))/4 - (3^(1/2)*dq2*dqr1*cos(q2)*cos(q3)*cos(q4)*cos(q5)*sin(q5))/2 + (3^(1/2)*dq3*dqr1*cos(q2)*cos(q3)*cos(q4)*cos(q5)*sin(q5))/2 + (3^(1/2)*dq1*dqr1*cos(q2)^2*cos(q3)*cos(q4)*cos(q5)*cos(q6)^2*sin(q3))/4 - (5*dq1*dqr1*cos(q2)^2*cos(q4)*cos(q5)*cos(q6)*sin(q4)*sin(q5)*sin(q6))/4 - (5*dq1*dqr1*cos(q3)^2*cos(q4)*cos(q5)*cos(q6)*sin(q4)*sin(q5)*sin(q6))/4 + (5*3^(1/2)*dq1*dqr1*cos(q2)^2*cos(q3)*cos(q4)*cos(q5)^2*cos(q6)^2*sin(q3))/8 - (3^(1/2)*dq2*dqr1*cos(q2)*cos(q3)*cos(q6)*sin(q4)*sin(q5)*sin(q6))/4 + (3^(1/2)*dq3*dqr1*cos(q2)*cos(q3)*cos(q6)*sin(q4)*sin(q5)*sin(q6))/4 + (3*dq1*dqr1*cos(q2)^2*cos(q3)^2*cos(q4)*cos(q6)*sin(q4)*sin(q5)*sin(q6))/2 + (5*3^(1/2)*dq2*dqr1*cos(q2)*cos(q3)*cos(q4)*cos(q5)*cos(q6)^2*sin(q5))/8 - (5*3^(1/2)*dq3*dqr1*cos(q2)*cos(q3)*cos(q4)*cos(q5)*cos(q6)^2*sin(q5))/8 - (3^(1/2)*dq2*dqr1*cos(q2)*cos(q3)*cos(q5)*cos(q6)*sin(q4)*sin(q5)*sin(q6))/4 + (3^(1/2)*dq3*dqr1*cos(q2)*cos(q3)*cos(q5)*cos(q6)*sin(q4)*sin(q5)*sin(q6))/4 + (5*dq1*dqr1*cos(q2)^2*cos(q3)^2*cos(q4)*cos(q5)*cos(q6)*sin(q4)*sin(q5)*sin(q6))/2;
Y4_20_4=(dq1*dqr2*cos(q2)*sin(q3))/4 - (dq1*dqr2*cos(q3)*sin(q2))/4 - (dq1*dqr2*cos(q2)*cos(q4)^2*sin(q3))/4 + (dq1*dqr2*cos(q3)*cos(q4)^2*sin(q2))/4 - (dq1*dqr2*cos(q2)*cos(q5)^2*sin(q3))/4 + (dq1*dqr2*cos(q3)*cos(q5)^2*sin(q2))/4 + (5*dq1*dqr2*cos(q2)*cos(q6)^2*sin(q3))/16 - (5*dq1*dqr2*cos(q3)*cos(q6)^2*sin(q2))/16 + (dq1*dqr1*cos(q3)^2*cos(q5)*sin(q5))/2 + (dq1*dqr1*cos(q2)^2*cos(q6)*sin(q6))/4 + (dq1*dqr1*cos(q3)^2*cos(q6)*sin(q6))/4 - (3*dq1*dqr1*cos(q3)^2*cos(q6)^2*sin(q5))/8 + (3^(1/2)*dq1*dqr2*sin(q2)*sin(q3)*sin(q4))/4 + (5*dq1*dqr2*cos(q2)*cos(q4)^2*cos(q5)^2*sin(q3))/4 - (5*dq1*dqr2*cos(q3)*cos(q4)^2*cos(q5)^2*sin(q2))/4 - (dq1*dqr2*cos(q2)*cos(q4)^2*cos(q6)^2*sin(q3))/16 + (dq1*dqr2*cos(q3)*cos(q4)^2*cos(q6)^2*sin(q2))/16 - (dq1*dqr1*cos(q2)^2*cos(q3)^2*cos(q6)*sin(q6))/2 + (5*dq1*dqr2*cos(q2)*cos(q5)^2*cos(q6)^2*sin(q3))/16 - (5*dq1*dqr2*cos(q3)*cos(q5)^2*cos(q6)^2*sin(q2))/16 - (dq1*dqr1*cos(q2)^2*cos(q4)^2*cos(q6)*sin(q6))/2 - (dq1*dqr1*cos(q2)^2*cos(q5)^2*cos(q6)*sin(q6))/2 - (5*dq1*dqr1*cos(q3)^2*cos(q5)*cos(q6)^2*sin(q5))/8 - (dq1*dqr1*cos(q3)^2*cos(q4)^2*cos(q6)*sin(q6))/2 - (dq1*dqr1*cos(q3)^2*cos(q5)^2*cos(q6)*sin(q6))/2 - (3*dq5*dqr1*cos(q2)*cos(q3)*cos(q6)*sin(q6))/8 - (9*dq6*dqr1*cos(q2)*cos(q3)*cos(q6)*sin(q6))/16 + (3*dq1*dqr1*cos(q3)^2*cos(q4)^2*cos(q6)^2*sin(q5))/4 + (3*dq1*dqr2*cos(q2)*cos(q5)*cos(q6)^2*sin(q3))/8 - (3*dq1*dqr2*cos(q3)*cos(q5)*cos(q6)^2*sin(q2))/8 - (3*dq1*dqr1*cos(q2)^2*cos(q5)*cos(q6)*sin(q6))/4 - (3*dq1*dqr1*cos(q3)^2*cos(q5)*cos(q6)*sin(q6))/4 - (3^(1/2)*dq6*dqr2*cos(q6)*sin(q4)*sin(q5)*sin(q6))/8 - (3*dq1*dqr2*cos(q2)*cos(q4)^2*cos(q5)*cos(q6)^2*sin(q3))/8 + (3*dq1*dqr2*cos(q3)*cos(q4)^2*cos(q5)*cos(q6)^2*sin(q2))/8 + (3*dq1*dqr1*cos(q2)^2*cos(q3)^2*cos(q5)*cos(q6)*sin(q6))/2 + (3*dq1*dqr1*cos(q2)^2*cos(q4)^2*cos(q5)*cos(q6)*sin(q6))/2 + (3*dq1*dqr1*cos(q3)^2*cos(q4)^2*cos(q5)*cos(q6)*sin(q6))/2 - (3^(1/2)*dq1*dqr2*cos(q2)*cos(q3)*cos(q5)^2*sin(q4))/4 - (7*3^(1/2)*dq1*dqr2*cos(q2)*cos(q3)*cos(q6)^2*sin(q4))/16 - (3*dq5*dqr1*cos(q2)*cos(q3)*cos(q5)*cos(q6)*sin(q6))/8 - (3*dq6*dqr1*cos(q2)*cos(q3)*cos(q5)*cos(q6)*sin(q6))/8 - (3^(1/2)*dq1*dqr2*cos(q5)^2*sin(q2)*sin(q3)*sin(q4))/4 - (7*3^(1/2)*dq1*dqr2*cos(q6)^2*sin(q2)*sin(q3)*sin(q4))/16 + dq1*dqr1*cos(q2)^2*cos(q3)^2*cos(q4)^2*cos(q6)*sin(q6) - (25*dq1*dqr2*cos(q2)*cos(q4)^2*cos(q5)^2*cos(q6)^2*sin(q3))/16 + (25*dq1*dqr2*cos(q3)*cos(q4)^2*cos(q5)^2*cos(q6)^2*sin(q2))/16 + dq1*dqr1*cos(q2)^2*cos(q3)^2*cos(q5)^2*cos(q6)*sin(q6) + dq1*dqr1*cos(q2)^2*cos(q4)^2*cos(q5)^2*cos(q6)*sin(q6) + dq1*dqr1*cos(q3)^2*cos(q4)^2*cos(q5)^2*cos(q6)*sin(q6) - (3*dq1*dqr2*cos(q2)*cos(q6)*sin(q3)*sin(q5)*sin(q6))/4 + (3*dq1*dqr2*cos(q3)*cos(q6)*sin(q2)*sin(q5)*sin(q6))/4 + (3*dq2*dqr2*cos(q4)*cos(q6)*sin(q4)*sin(q5)*sin(q6))/4 - (3*dq3*dqr2*cos(q4)*cos(q6)*sin(q4)*sin(q5)*sin(q6))/4 + (3*dq5*dqr1*cos(q2)*cos(q3)*cos(q5)^2*cos(q6)*sin(q6))/4 + (15*dq6*dqr1*cos(q2)*cos(q3)*cos(q5)^2*cos(q6)*sin(q6))/16 + (3^(1/2)*dq1*dqr2*cos(q2)*cos(q3)*cos(q5)*cos(q6)^2*sin(q4))/8 - (3^(1/2)*dq1*dqr2*cos(q4)*cos(q6)^2*sin(q2)*sin(q3)*sin(q5))/8 + (3^(1/2)*dq1*dqr2*cos(q5)*cos(q6)^2*sin(q2)*sin(q3)*sin(q4))/8 - 3*dq1*dqr1*cos(q2)^2*cos(q3)^2*cos(q4)^2*cos(q5)*cos(q6)*sin(q6) - dq1*dqr2*cos(q2)*cos(q4)*cos(q5)*sin(q3)*sin(q4)*sin(q5) + dq1*dqr2*cos(q3)*cos(q4)*cos(q5)*sin(q2)*sin(q4)*sin(q5) - (dq1*dqr2*cos(q2)*cos(q4)*cos(q6)*sin(q3)*sin(q4)*sin(q6))/2 + (dq1*dqr2*cos(q3)*cos(q4)*cos(q6)*sin(q2)*sin(q4)*sin(q6))/2 - (dq1*dqr2*cos(q2)*cos(q5)*cos(q6)*sin(q3)*sin(q5)*sin(q6))/4 + (dq1*dqr2*cos(q3)*cos(q5)*cos(q6)*sin(q2)*sin(q5)*sin(q6))/4 + (5*dq2*dqr2*cos(q4)*cos(q5)*cos(q6)*sin(q4)*sin(q5)*sin(q6))/4 - (5*dq3*dqr2*cos(q4)*cos(q5)*cos(q6)*sin(q4)*sin(q5)*sin(q6))/4 + (5*3^(1/2)*dq1*dqr2*cos(q2)*cos(q3)*cos(q5)^2*cos(q6)^2*sin(q4))/16 + (5*3^(1/2)*dq1*dqr2*cos(q5)^2*cos(q6)^2*sin(q2)*sin(q3)*sin(q4))/16 - 2*dq1*dqr1*cos(q2)^2*cos(q3)^2*cos(q4)^2*cos(q5)^2*cos(q6)*sin(q6) + (3*dq1*dqr2*cos(q2)*cos(q4)*cos(q6)^2*sin(q3)*sin(q4)*sin(q5))/4 - (3*dq1*dqr2*cos(q3)*cos(q4)*cos(q6)^2*sin(q2)*sin(q4)*sin(q5))/4 + (3*dq1*dqr2*cos(q2)*cos(q4)^2*cos(q6)*sin(q3)*sin(q5)*sin(q6))/4 - (3*dq1*dqr2*cos(q3)*cos(q4)^2*cos(q6)*sin(q2)*sin(q5)*sin(q6))/4 - (3^(1/2)*dq2*dqr1*cos(q2)*cos(q3)*cos(q4)*cos(q6)*sin(q6))/4 + (3^(1/2)*dq3*dqr1*cos(q2)*cos(q3)*cos(q4)*cos(q6)*sin(q6))/4 - (3^(1/2)*dq1*dqr2*cos(q4)*cos(q5)*sin(q2)*sin(q3)*sin(q5))/2 - (3^(1/2)*dq1*dqr2*cos(q4)*cos(q6)*sin(q2)*sin(q3)*sin(q6))/4 + (3^(1/2)*dq5*dqr2*cos(q5)*cos(q6)*sin(q4)*sin(q5)*sin(q6))/2 + (5*3^(1/2)*dq6*dqr2*cos(q5)*cos(q6)*sin(q4)*sin(q5)*sin(q6))/8 + (5*3^(1/2)*dq1*dqr2*cos(q4)*cos(q5)*cos(q6)^2*sin(q2)*sin(q3)*sin(q5))/8 + (3^(1/2)*dq1*dqr2*cos(q4)*cos(q5)^2*cos(q6)*sin(q2)*sin(q3)*sin(q6))/2 + (3*dq1*dqr2*cos(q2)*cos(q4)*cos(q5)*cos(q6)*sin(q3)*sin(q4)*sin(q6))/2 - (3*dq1*dqr2*cos(q3)*cos(q4)*cos(q5)*cos(q6)*sin(q2)*sin(q4)*sin(q6))/2 + (5*dq1*dqr2*cos(q2)*cos(q4)*cos(q5)*cos(q6)^2*sin(q3)*sin(q4)*sin(q5))/4 - (5*dq1*dqr2*cos(q3)*cos(q4)*cos(q5)*cos(q6)^2*sin(q2)*sin(q4)*sin(q5))/4 + dq1*dqr2*cos(q2)*cos(q4)*cos(q5)^2*cos(q6)*sin(q3)*sin(q4)*sin(q6) - dq1*dqr2*cos(q3)*cos(q4)*cos(q5)^2*cos(q6)*sin(q2)*sin(q4)*sin(q6) + (5*dq1*dqr2*cos(q2)*cos(q4)^2*cos(q5)*cos(q6)*sin(q3)*sin(q5)*sin(q6))/4 - (5*dq1*dqr2*cos(q3)*cos(q4)^2*cos(q5)*cos(q6)*sin(q2)*sin(q5)*sin(q6))/4 - (3^(1/2)*dq2*dqr1*cos(q2)*cos(q3)*cos(q4)*cos(q5)*cos(q6)*sin(q6))/4 + (3^(1/2)*dq3*dqr1*cos(q2)*cos(q3)*cos(q4)*cos(q5)*cos(q6)*sin(q6))/4 - (3^(1/2)*dq1*dqr2*cos(q2)*cos(q3)*cos(q6)*sin(q4)*sin(q5)*sin(q6))/4 - (3^(1/2)*dq1*dqr2*cos(q4)*cos(q5)*cos(q6)*sin(q2)*sin(q3)*sin(q6))/4 - (3^(1/2)*dq1*dqr2*cos(q6)*sin(q2)*sin(q3)*sin(q4)*sin(q5)*sin(q6))/4 + (3^(1/2)*dq2*dqr1*cos(q2)*cos(q3)*cos(q4)*cos(q5)^2*cos(q6)*sin(q6))/2 - (3^(1/2)*dq3*dqr1*cos(q2)*cos(q3)*cos(q4)*cos(q5)^2*cos(q6)*sin(q6))/2 - (3^(1/2)*dq1*dqr2*cos(q2)*cos(q3)*cos(q5)*cos(q6)*sin(q4)*sin(q5)*sin(q6))/4 - (3^(1/2)*dq1*dqr2*cos(q5)*cos(q6)*sin(q2)*sin(q3)*sin(q4)*sin(q5)*sin(q6))/4;
Y4_20_5=(dq3*dqr2*sin(2*q4))/8 - (dq2*dqr2*sin(2*q5))/4 - (dq2*dqr2*sin(2*q4))/8 - (dq2*dqr2*sin(2*q6))/8 + (dq3*dqr2*sin(2*q5))/4 + (dq3*dqr2*sin(2*q6))/8 + (3*dq2*dqr2*cos(q6)^2*sin(q5))/8 - (3*dq3*dqr2*cos(q6)^2*sin(q5))/8 + (dq1*dqr3*cos(q3)*sin(q2))/4 - (dq1*dqr3*cos(q3)*cos(q4)^2*sin(q2))/4 - (dq1*dqr3*cos(q3)*cos(q5)^2*sin(q2))/4 + (5*dq1*dqr3*cos(q3)*cos(q6)^2*sin(q2))/16 + (5*dq2*dqr2*cos(q4)*cos(q5)^2*sin(q4))/4 - (dq2*dqr2*cos(q4)*cos(q6)^2*sin(q4))/16 + dq2*dqr2*cos(q4)^2*cos(q5)*sin(q5) - (5*dq3*dqr2*cos(q4)*cos(q5)^2*sin(q4))/4 + (dq3*dqr2*cos(q4)*cos(q6)^2*sin(q4))/16 - dq3*dqr2*cos(q4)^2*cos(q5)*sin(q5) + (5*dq2*dqr2*cos(q5)*cos(q6)^2*sin(q5))/8 + (dq2*dqr2*cos(q4)^2*cos(q6)*sin(q6))/2 + (dq2*dqr2*cos(q5)^2*cos(q6)*sin(q6))/2 - (5*dq3*dqr2*cos(q5)*cos(q6)^2*sin(q5))/8 - (dq3*dqr2*cos(q4)^2*cos(q6)*sin(q6))/2 - (dq3*dqr2*cos(q5)^2*cos(q6)*sin(q6))/2 - (3^(1/2)*dq6*dqr2*cos(q4)*sin(q5))/8 - (3^(1/2)*dq6*dqr2*cos(q5)*sin(q4))/4 - (3*dq2*dqr2*cos(q4)^2*cos(q6)^2*sin(q5))/4 + (3*dq3*dqr2*cos(q4)^2*cos(q6)^2*sin(q5))/4 + (3^(1/2)*dq5*dqr2*cos(q5)^2*sin(q4))/2 + (3^(1/2)*dq5*dqr2*cos(q6)^2*sin(q4))/8 + (3^(1/2)*dq6*dqr2*cos(q5)^2*sin(q4))/4 + (3^(1/2)*dq6*dqr2*cos(q6)^2*sin(q4))/4 + (3*dq2*dqr2*cos(q5)*cos(q6)*sin(q6))/4 - (3*dq3*dqr2*cos(q5)*cos(q6)*sin(q6))/4 + (3^(1/2)*dq1*dqr2*cos(q2)*cos(q3)*sin(q4))/4 + (3^(1/2)*dq5*dqr2*cos(q4)*cos(q5)*sin(q5))/4 + (3^(1/2)*dq6*dqr2*cos(q4)*cos(q5)*sin(q5))/8 + (3^(1/2)*dq5*dqr2*cos(q4)*cos(q6)*sin(q6))/8 + (7*3^(1/2)*dq6*dqr2*cos(q4)*cos(q6)*sin(q6))/16 - (3^(1/2)*dq1*dqr3*sin(q2)*sin(q3)*sin(q4))/4 + (5*dq1*dqr3*cos(q3)*cos(q4)^2*cos(q5)^2*sin(q2))/4 - (dq1*dqr3*cos(q3)*cos(q4)^2*cos(q6)^2*sin(q2))/16 + (5*dq1*dqr3*cos(q3)*cos(q5)^2*cos(q6)^2*sin(q2))/16 - (25*dq2*dqr2*cos(q4)*cos(q5)^2*cos(q6)^2*sin(q4))/16 - (5*dq2*dqr2*cos(q4)^2*cos(q5)*cos(q6)^2*sin(q5))/4 + (25*dq3*dqr2*cos(q4)*cos(q5)^2*cos(q6)^2*sin(q4))/16 - dq2*dqr2*cos(q4)^2*cos(q5)^2*cos(q6)*sin(q6) + (5*dq3*dqr2*cos(q4)^2*cos(q5)*cos(q6)^2*sin(q5))/4 + dq3*dqr2*cos(q4)^2*cos(q5)^2*cos(q6)*sin(q6) - (3*3^(1/2)*dq5*dqr2*cos(q4)*cos(q6)^2*sin(q5))/16 - (3^(1/2)*dq6*dqr2*cos(q4)*cos(q6)^2*sin(q5))/4 + (3^(1/2)*dq6*dqr2*cos(q5)*cos(q6)^2*sin(q4))/4 - (5*3^(1/2)*dq5*dqr2*cos(q5)^2*cos(q6)^2*sin(q4))/8 - (3^(1/2)*dq6*dqr2*cos(q5)^2*cos(q6)^2*sin(q4))/2 + (3*dq1*dqr3*cos(q3)*cos(q5)*cos(q6)^2*sin(q2))/8 - (3*dq2*dqr2*cos(q4)*cos(q5)*cos(q6)^2*sin(q4))/8 + (3*dq3*dqr2*cos(q4)*cos(q5)*cos(q6)^2*sin(q4))/8 - (3*dq2*dqr2*cos(q4)^2*cos(q5)*cos(q6)*sin(q6))/2 + (3*dq3*dqr2*cos(q4)^2*cos(q5)*cos(q6)*sin(q6))/2 - (3*dq1*dqr3*cos(q3)*cos(q4)^2*cos(q5)*cos(q6)^2*sin(q2))/8 - (5*3^(1/2)*dq5*dqr2*cos(q4)*cos(q5)*cos(q6)^2*sin(q5))/16 - (3^(1/2)*dq5*dqr2*cos(q4)*cos(q5)^2*cos(q6)*sin(q6))/4 - (3^(1/2)*dq6*dqr2*cos(q4)*cos(q5)*cos(q6)^2*sin(q5))/4 - (5*3^(1/2)*dq6*dqr2*cos(q4)*cos(q5)^2*cos(q6)*sin(q6))/16 + (3^(1/2)*dq1*dqr3*cos(q5)^2*sin(q2)*sin(q3)*sin(q4))/4 + (7*3^(1/2)*dq1*dqr3*cos(q6)^2*sin(q2)*sin(q3)*sin(q4))/16 - (25*dq1*dqr3*cos(q3)*cos(q4)^2*cos(q5)^2*cos(q6)^2*sin(q2))/16 - (3*dq1*dqr3*cos(q3)*cos(q6)*sin(q2)*sin(q5)*sin(q6))/4 - (3*3^(1/2)*dq5*dqr2*cos(q4)*cos(q5)*cos(q6)*sin(q6))/8 - (3^(1/2)*dq6*dqr2*cos(q4)*cos(q5)*cos(q6)*sin(q6))/8 - (3^(1/2)*dq1*dqr2*cos(q2)*cos(q3)*cos(q4)*cos(q6)^2*sin(q5))/8 + (3^(1/2)*dq1*dqr3*cos(q4)*cos(q6)^2*sin(q2)*sin(q3)*sin(q5))/8 - (3^(1/2)*dq1*dqr3*cos(q5)*cos(q6)^2*sin(q2)*sin(q3)*sin(q4))/8 + dq1*dqr3*cos(q2)*cos(q4)*cos(q5)*sin(q3)*sin(q4)*sin(q5) - dq1*dqr3*cos(q3)*cos(q4)*cos(q5)*sin(q2)*sin(q4)*sin(q5) - (dq1*dqr3*cos(q3)*cos(q4)*cos(q6)*sin(q2)*sin(q4)*sin(q6))/2 - (dq1*dqr3*cos(q3)*cos(q5)*cos(q6)*sin(q2)*sin(q5)*sin(q6))/4 - (5*3^(1/2)*dq1*dqr3*cos(q5)^2*cos(q6)^2*sin(q2)*sin(q3)*sin(q4))/16 - (3*dq1*dqr3*cos(q2)*cos(q4)*cos(q6)^2*sin(q3)*sin(q4)*sin(q5))/4 + (3*dq1*dqr3*cos(q3)*cos(q4)*cos(q6)^2*sin(q2)*sin(q4)*sin(q5))/4 + (3*dq1*dqr3*cos(q3)*cos(q4)^2*cos(q6)*sin(q2)*sin(q5)*sin(q6))/4 - (3^(1/2)*dq1*dqr2*cos(q2)*cos(q3)*cos(q4)*cos(q5)*sin(q5))/2 - (3^(1/2)*dq1*dqr2*cos(q2)*cos(q3)*cos(q4)*cos(q6)*sin(q6))/4 + (3^(1/2)*dq1*dqr3*cos(q4)*cos(q5)*sin(q2)*sin(q3)*sin(q5))/2 + (3^(1/2)*dq1*dqr3*cos(q4)*cos(q6)*sin(q2)*sin(q3)*sin(q6))/4 - (5*3^(1/2)*dq1*dqr3*cos(q4)*cos(q5)*cos(q6)^2*sin(q2)*sin(q3)*sin(q5))/8 - (3^(1/2)*dq1*dqr3*cos(q4)*cos(q5)^2*cos(q6)*sin(q2)*sin(q3)*sin(q6))/2 - (3*dq1*dqr3*cos(q2)*cos(q4)*cos(q5)*cos(q6)*sin(q3)*sin(q4)*sin(q6))/2 + (3*dq1*dqr3*cos(q3)*cos(q4)*cos(q5)*cos(q6)*sin(q2)*sin(q4)*sin(q6))/2 - (5*dq1*dqr3*cos(q2)*cos(q4)*cos(q5)*cos(q6)^2*sin(q3)*sin(q4)*sin(q5))/4 + (5*dq1*dqr3*cos(q3)*cos(q4)*cos(q5)*cos(q6)^2*sin(q2)*sin(q4)*sin(q5))/4 - dq1*dqr3*cos(q2)*cos(q4)*cos(q5)^2*cos(q6)*sin(q3)*sin(q4)*sin(q6) + dq1*dqr3*cos(q3)*cos(q4)*cos(q5)^2*cos(q6)*sin(q2)*sin(q4)*sin(q6) + (5*dq1*dqr3*cos(q3)*cos(q4)^2*cos(q5)*cos(q6)*sin(q2)*sin(q5)*sin(q6))/4 - (3^(1/2)*dq1*dqr2*cos(q2)*cos(q3)*cos(q4)*cos(q5)*cos(q6)*sin(q6))/4 + (3^(1/2)*dq1*dqr3*cos(q4)*cos(q5)*cos(q6)*sin(q2)*sin(q3)*sin(q6))/4 + (3^(1/2)*dq1*dqr3*cos(q6)*sin(q2)*sin(q3)*sin(q4)*sin(q5)*sin(q6))/4 + (5*3^(1/2)*dq1*dqr2*cos(q2)*cos(q3)*cos(q4)*cos(q5)*cos(q6)^2*sin(q5))/8 + (3^(1/2)*dq1*dqr2*cos(q2)*cos(q3)*cos(q4)*cos(q5)^2*cos(q6)*sin(q6))/2 + (3^(1/2)*dq1*dqr3*cos(q5)*cos(q6)*sin(q2)*sin(q3)*sin(q4)*sin(q5)*sin(q6))/4;
Y4_20_6=(3*dq6*dqr4*sin(q5))/8 + (dq2*dqr3*sin(2*q4))/8 + (dq2*dqr3*sin(2*q5))/4 - (dq3*dqr3*sin(2*q4))/8 + (dq2*dqr3*sin(2*q6))/8 - (dq3*dqr3*sin(2*q5))/4 - (dq3*dqr3*sin(2*q6))/8 - (3*dq5*dqr4*sin(2*q5))/8 - (3*dq2*dqr3*cos(q6)^2*sin(q5))/8 + (3*dq3*dqr3*cos(q6)^2*sin(q5))/8 - (3*dq5*dqr4*cos(q6)^2*sin(q5))/16 - (3*dq6*dqr4*cos(q6)^2*sin(q5))/4 - (dq1*dqr3*cos(q2)*sin(q3))/4 + (dq1*dqr3*cos(q2)*cos(q4)^2*sin(q3))/4 + (dq1*dqr3*cos(q2)*cos(q5)^2*sin(q3))/4 - (5*dq1*dqr3*cos(q2)*cos(q6)^2*sin(q3))/16 - (5*dq2*dqr3*cos(q4)*cos(q5)^2*sin(q4))/4 + (dq2*dqr3*cos(q4)*cos(q6)^2*sin(q4))/16 - dq2*dqr3*cos(q4)^2*cos(q5)*sin(q5) + (5*dq3*dqr3*cos(q4)*cos(q5)^2*sin(q4))/4 - (dq3*dqr3*cos(q4)*cos(q6)^2*sin(q4))/16 + dq3*dqr3*cos(q4)^2*cos(q5)*sin(q5) - (5*dq2*dqr3*cos(q5)*cos(q6)^2*sin(q5))/8 - (dq2*dqr3*cos(q4)^2*cos(q6)*sin(q6))/2 - (dq2*dqr3*cos(q5)^2*cos(q6)*sin(q6))/2 + (5*dq3*dqr3*cos(q5)*cos(q6)^2*sin(q5))/8 + (dq3*dqr3*cos(q4)^2*cos(q6)*sin(q6))/2 + (dq3*dqr3*cos(q5)^2*cos(q6)*sin(q6))/2 + (15*dq5*dqr4*cos(q5)*cos(q6)^2*sin(q5))/16 + (3*dq5*dqr4*cos(q5)^2*cos(q6)*sin(q6))/4 + (3*dq6*dqr4*cos(q5)*cos(q6)^2*sin(q5))/4 + (15*dq6*dqr4*cos(q5)^2*cos(q6)*sin(q6))/16 + (3^(1/2)*dq6*dqr3*cos(q4)*sin(q5))/8 + (3^(1/2)*dq6*dqr3*cos(q5)*sin(q4))/4 + (3*dq2*dqr3*cos(q4)^2*cos(q6)^2*sin(q5))/4 - (3*dq3*dqr3*cos(q4)^2*cos(q6)^2*sin(q5))/4 - (3^(1/2)*dq5*dqr3*cos(q5)^2*sin(q4))/2 - (3^(1/2)*dq5*dqr3*cos(q6)^2*sin(q4))/8 - (3^(1/2)*dq6*dqr3*cos(q5)^2*sin(q4))/4 - (3^(1/2)*dq6*dqr3*cos(q6)^2*sin(q4))/4 - (3*dq2*dqr3*cos(q5)*cos(q6)*sin(q6))/4 + (3*dq3*dqr3*cos(q5)*cos(q6)*sin(q6))/4 - (3*dq5*dqr4*cos(q5)*cos(q6)*sin(q6))/8 - (3*dq6*dqr4*cos(q5)*cos(q6)*sin(q6))/8 - (3^(1/2)*dq1*dqr3*cos(q2)*cos(q3)*sin(q4))/4 - (3^(1/2)*dq5*dqr3*cos(q4)*cos(q5)*sin(q5))/4 - (3^(1/2)*dq6*dqr3*cos(q4)*cos(q5)*sin(q5))/8 - (3^(1/2)*dq5*dqr3*cos(q4)*cos(q6)*sin(q6))/8 - (7*3^(1/2)*dq6*dqr3*cos(q4)*cos(q6)*sin(q6))/16 - (5*dq1*dqr3*cos(q2)*cos(q4)^2*cos(q5)^2*sin(q3))/4 + (dq1*dqr3*cos(q2)*cos(q4)^2*cos(q6)^2*sin(q3))/16 - (5*dq1*dqr3*cos(q2)*cos(q5)^2*cos(q6)^2*sin(q3))/16 + (25*dq2*dqr3*cos(q4)*cos(q5)^2*cos(q6)^2*sin(q4))/16 + (5*dq2*dqr3*cos(q4)^2*cos(q5)*cos(q6)^2*sin(q5))/4 - (25*dq3*dqr3*cos(q4)*cos(q5)^2*cos(q6)^2*sin(q4))/16 + dq2*dqr3*cos(q4)^2*cos(q5)^2*cos(q6)*sin(q6) - (5*dq3*dqr3*cos(q4)^2*cos(q5)*cos(q6)^2*sin(q5))/4 - dq3*dqr3*cos(q4)^2*cos(q5)^2*cos(q6)*sin(q6) + (3*3^(1/2)*dq5*dqr3*cos(q4)*cos(q6)^2*sin(q5))/16 + (3^(1/2)*dq6*dqr3*cos(q4)*cos(q6)^2*sin(q5))/4 - (3^(1/2)*dq6*dqr3*cos(q5)*cos(q6)^2*sin(q4))/4 + (5*3^(1/2)*dq5*dqr3*cos(q5)^2*cos(q6)^2*sin(q4))/8 + (3^(1/2)*dq6*dqr3*cos(q5)^2*cos(q6)^2*sin(q4))/2 - (3*dq1*dqr3*cos(q2)*cos(q5)*cos(q6)^2*sin(q3))/8 + (3*dq2*dqr3*cos(q4)*cos(q5)*cos(q6)^2*sin(q4))/8 - (3*dq3*dqr3*cos(q4)*cos(q5)*cos(q6)^2*sin(q4))/8 + (3*dq2*dqr3*cos(q4)^2*cos(q5)*cos(q6)*sin(q6))/2 - (3*dq3*dqr3*cos(q4)^2*cos(q5)*cos(q6)*sin(q6))/2 + (3^(1/2)*dq6*dqr3*cos(q6)*sin(q4)*sin(q5)*sin(q6))/8 + (3*dq1*dqr3*cos(q2)*cos(q4)^2*cos(q5)*cos(q6)^2*sin(q3))/8 + (3^(1/2)*dq1*dqr3*cos(q2)*cos(q3)*cos(q5)^2*sin(q4))/4 + (7*3^(1/2)*dq1*dqr3*cos(q2)*cos(q3)*cos(q6)^2*sin(q4))/16 + (5*3^(1/2)*dq5*dqr3*cos(q4)*cos(q5)*cos(q6)^2*sin(q5))/16 + (3^(1/2)*dq5*dqr3*cos(q4)*cos(q5)^2*cos(q6)*sin(q6))/4 + (3^(1/2)*dq6*dqr3*cos(q4)*cos(q5)*cos(q6)^2*sin(q5))/4 + (5*3^(1/2)*dq6*dqr3*cos(q4)*cos(q5)^2*cos(q6)*sin(q6))/16 + (25*dq1*dqr3*cos(q2)*cos(q4)^2*cos(q5)^2*cos(q6)^2*sin(q3))/16 + (3*dq1*dqr3*cos(q2)*cos(q6)*sin(q3)*sin(q5)*sin(q6))/4 - (3*dq2*dqr3*cos(q4)*cos(q6)*sin(q4)*sin(q5)*sin(q6))/4 + (3*dq3*dqr3*cos(q4)*cos(q6)*sin(q4)*sin(q5)*sin(q6))/4 + (3*3^(1/2)*dq5*dqr3*cos(q4)*cos(q5)*cos(q6)*sin(q6))/8 + (3^(1/2)*dq6*dqr3*cos(q4)*cos(q5)*cos(q6)*sin(q6))/8 + (3^(1/2)*dq1*dqr3*cos(q2)*cos(q3)*cos(q4)*cos(q6)^2*sin(q5))/8 - (3^(1/2)*dq1*dqr3*cos(q2)*cos(q3)*cos(q5)*cos(q6)^2*sin(q4))/8 + (dq1*dqr3*cos(q2)*cos(q4)*cos(q6)*sin(q3)*sin(q4)*sin(q6))/2 + (dq1*dqr3*cos(q2)*cos(q5)*cos(q6)*sin(q3)*sin(q5)*sin(q6))/4 - (5*dq2*dqr3*cos(q4)*cos(q5)*cos(q6)*sin(q4)*sin(q5)*sin(q6))/4 + (5*dq3*dqr3*cos(q4)*cos(q5)*cos(q6)*sin(q4)*sin(q5)*sin(q6))/4 - (5*3^(1/2)*dq1*dqr3*cos(q2)*cos(q3)*cos(q5)^2*cos(q6)^2*sin(q4))/16 - (3*dq1*dqr3*cos(q2)*cos(q4)^2*cos(q6)*sin(q3)*sin(q5)*sin(q6))/4 + (3^(1/2)*dq1*dqr3*cos(q2)*cos(q3)*cos(q4)*cos(q5)*sin(q5))/2 + (3^(1/2)*dq1*dqr3*cos(q2)*cos(q3)*cos(q4)*cos(q6)*sin(q6))/4 - (3^(1/2)*dq5*dqr3*cos(q5)*cos(q6)*sin(q4)*sin(q5)*sin(q6))/2 - (5*3^(1/2)*dq6*dqr3*cos(q5)*cos(q6)*sin(q4)*sin(q5)*sin(q6))/8 - (5*dq1*dqr3*cos(q2)*cos(q4)^2*cos(q5)*cos(q6)*sin(q3)*sin(q5)*sin(q6))/4 + (3^(1/2)*dq1*dqr3*cos(q2)*cos(q3)*cos(q4)*cos(q5)*cos(q6)*sin(q6))/4 + (3^(1/2)*dq1*dqr3*cos(q2)*cos(q3)*cos(q6)*sin(q4)*sin(q5)*sin(q6))/4 - (5*3^(1/2)*dq1*dqr3*cos(q2)*cos(q3)*cos(q4)*cos(q5)*cos(q6)^2*sin(q5))/8 - (3^(1/2)*dq1*dqr3*cos(q2)*cos(q3)*cos(q4)*cos(q5)^2*cos(q6)*sin(q6))/2 + (3^(1/2)*dq1*dqr3*cos(q2)*cos(q3)*cos(q5)*cos(q6)*sin(q4)*sin(q5)*sin(q6))/4;
Y4_20_7=(3*dq6*dqr5*sin(2*q6))/16 - (3*dq4*dqr5*sin(2*q6))/16 - (3*dq5*dqr4*sin(2*q6))/16 - (3*dq6*dqr4*sin(2*q5))/16 - (9*dq6*dqr4*sin(2*q6))/32 - (3*dq4*dqr5*sin(2*q5))/8 - (3*dq4*dqr5*cos(q6)^2*sin(q5))/16 - (3*dq5*dqr5*cos(q6)^2*sin(q5))/8 - (3*dq6*dqr5*cos(q6)^2*sin(q5))/4 + (15*dq4*dqr5*cos(q5)*cos(q6)^2*sin(q5))/16 + (3*dq4*dqr5*cos(q5)^2*cos(q6)*sin(q6))/4 + (3^(1/2)*dq2*dqr5*cos(q5)^2*sin(q4))/2 + (3^(1/2)*dq2*dqr5*cos(q6)^2*sin(q4))/8 - (3^(1/2)*dq3*dqr5*cos(q5)^2*sin(q4))/2 - (3^(1/2)*dq3*dqr5*cos(q6)^2*sin(q4))/8 - (3*dq4*dqr5*cos(q5)*cos(q6)*sin(q6))/8 - (3*dq5*dqr5*cos(q5)*cos(q6)*sin(q6))/4 - (3*dq6*dqr5*cos(q5)*cos(q6)*sin(q6))/8 + (3*dq1*dqr6*sin(q2)*sin(q3)*sin(q5))/8 - (3*dq1*dqr5*cos(q6)^2*sin(q2)*sin(q3)*sin(q5))/16 - (3*dq1*dqr6*cos(q6)^2*sin(q2)*sin(q3)*sin(q5))/4 + (3^(1/2)*dq2*dqr5*cos(q4)*cos(q5)*sin(q5))/4 - (3^(1/2)*dq3*dqr5*cos(q4)*cos(q5)*sin(q5))/4 + (3^(1/2)*dq2*dqr5*cos(q4)*cos(q6)*sin(q6))/8 - (3^(1/2)*dq3*dqr5*cos(q4)*cos(q6)*sin(q6))/8 - (3*3^(1/2)*dq2*dqr5*cos(q4)*cos(q6)^2*sin(q5))/16 + (3*3^(1/2)*dq3*dqr5*cos(q4)*cos(q6)^2*sin(q5))/16 - (3*dq1*dqr5*cos(q2)*cos(q3)*cos(q5)*sin(q5))/4 - (3*dq1*dqr5*cos(q2)*cos(q3)*cos(q6)*sin(q6))/8 - (3*dq1*dqr5*cos(q5)*sin(q2)*sin(q3)*sin(q5))/4 - (3*dq1*dqr6*cos(q5)*sin(q2)*sin(q3)*sin(q5))/8 - (3*dq1*dqr5*cos(q6)*sin(q2)*sin(q3)*sin(q6))/8 - (9*dq1*dqr6*cos(q6)*sin(q2)*sin(q3)*sin(q6))/16 - (5*3^(1/2)*dq2*dqr5*cos(q5)^2*cos(q6)^2*sin(q4))/8 + (5*3^(1/2)*dq3*dqr5*cos(q5)^2*cos(q6)^2*sin(q4))/8 - (3*dq1*dqr5*cos(q2)*cos(q3)*cos(q6)^2*sin(q5))/16 + (3^(1/2)*dq1*dqr6*cos(q2)*sin(q3)*sin(q4)*sin(q5))/8 - (3^(1/2)*dq1*dqr6*cos(q3)*sin(q2)*sin(q4)*sin(q5))/8 + (3^(1/2)*dq1*dqr5*cos(q2)*cos(q4)*cos(q5)^2*sin(q3))/2 - (3^(1/2)*dq1*dqr5*cos(q3)*cos(q4)*cos(q5)^2*sin(q2))/2 + (3^(1/2)*dq1*dqr5*cos(q2)*cos(q4)*cos(q6)^2*sin(q3))/8 - (3^(1/2)*dq1*dqr5*cos(q3)*cos(q4)*cos(q6)^2*sin(q2))/8 + (3^(1/2)*dq1*dqr6*cos(q2)*cos(q4)*cos(q5)^2*sin(q3))/4 - (3^(1/2)*dq1*dqr6*cos(q3)*cos(q4)*cos(q5)^2*sin(q2))/4 - (3^(1/2)*dq1*dqr6*cos(q3)*cos(q4)*cos(q6)^2*sin(q2))/4 - (5*3^(1/2)*dq2*dqr5*cos(q4)*cos(q5)*cos(q6)^2*sin(q5))/16 - (3^(1/2)*dq2*dqr5*cos(q4)*cos(q5)^2*cos(q6)*sin(q6))/4 + (5*3^(1/2)*dq3*dqr5*cos(q4)*cos(q5)*cos(q6)^2*sin(q5))/16 + (3^(1/2)*dq3*dqr5*cos(q4)*cos(q5)^2*cos(q6)*sin(q6))/4 - (3*dq1*dqr5*cos(q2)*cos(q3)*cos(q5)*cos(q6)*sin(q6))/8 - (3*dq1*dqr5*cos(q5)*cos(q6)*sin(q2)*sin(q3)*sin(q6))/8 - (3*dq1*dqr6*cos(q5)*cos(q6)*sin(q2)*sin(q3)*sin(q6))/8 + (15*dq1*dqr5*cos(q2)*cos(q3)*cos(q5)*cos(q6)^2*sin(q5))/16 + (3*dq1*dqr5*cos(q2)*cos(q3)*cos(q5)^2*cos(q6)*sin(q6))/4 + (15*dq1*dqr5*cos(q5)*cos(q6)^2*sin(q2)*sin(q3)*sin(q5))/16 + (3*dq1*dqr5*cos(q5)^2*cos(q6)*sin(q2)*sin(q3)*sin(q6))/4 + (3*dq1*dqr6*cos(q5)*cos(q6)^2*sin(q2)*sin(q3)*sin(q5))/4 + (15*dq1*dqr6*cos(q5)^2*cos(q6)*sin(q2)*sin(q3)*sin(q6))/16 - (3^(1/2)*dq1*dqr6*cos(q2)*cos(q4)*cos(q5)*sin(q3))/4 + (3^(1/2)*dq1*dqr6*cos(q3)*cos(q4)*cos(q5)*sin(q2))/4 - (3*3^(1/2)*dq2*dqr5*cos(q4)*cos(q5)*cos(q6)*sin(q6))/8 + (3*3^(1/2)*dq3*dqr5*cos(q4)*cos(q5)*cos(q6)*sin(q6))/8 + (3^(1/2)*dq1*dqr6*cos(q2)*cos(q4)*cos(q5)*cos(q6)^2*sin(q3))/4 - (3^(1/2)*dq1*dqr6*cos(q3)*cos(q4)*cos(q5)*cos(q6)^2*sin(q2))/4 + (3*3^(1/2)*dq1*dqr5*cos(q2)*cos(q6)^2*sin(q3)*sin(q4)*sin(q5))/16 - (3*3^(1/2)*dq1*dqr5*cos(q3)*cos(q6)^2*sin(q2)*sin(q4)*sin(q5))/16 + (3^(1/2)*dq1*dqr6*cos(q2)*cos(q6)^2*sin(q3)*sin(q4)*sin(q5))/4 - (3^(1/2)*dq1*dqr6*cos(q3)*cos(q6)^2*sin(q2)*sin(q4)*sin(q5))/4 - (5*3^(1/2)*dq1*dqr5*cos(q2)*cos(q4)*cos(q5)^2*cos(q6)^2*sin(q3))/8 + (5*3^(1/2)*dq1*dqr5*cos(q3)*cos(q4)*cos(q5)^2*cos(q6)^2*sin(q2))/8 - (3^(1/2)*dq1*dqr6*cos(q2)*cos(q4)*cos(q5)^2*cos(q6)^2*sin(q3))/2 + (3^(1/2)*dq1*dqr6*cos(q3)*cos(q4)*cos(q5)^2*cos(q6)^2*sin(q2))/2 - (3^(1/2)*dq1*dqr5*cos(q2)*cos(q5)*sin(q3)*sin(q4)*sin(q5))/4 + (3^(1/2)*dq1*dqr5*cos(q3)*cos(q5)*sin(q2)*sin(q4)*sin(q5))/4 - (3^(1/2)*dq1*dqr6*cos(q2)*cos(q5)*sin(q3)*sin(q4)*sin(q5))/8 + (3^(1/2)*dq1*dqr6*cos(q3)*cos(q5)*sin(q2)*sin(q4)*sin(q5))/8 - (3^(1/2)*dq1*dqr5*cos(q2)*cos(q6)*sin(q3)*sin(q4)*sin(q6))/8 + (3^(1/2)*dq1*dqr5*cos(q3)*cos(q6)*sin(q2)*sin(q4)*sin(q6))/8 - (7*3^(1/2)*dq1*dqr6*cos(q2)*cos(q6)*sin(q3)*sin(q4)*sin(q6))/16 + (7*3^(1/2)*dq1*dqr6*cos(q3)*cos(q6)*sin(q2)*sin(q4)*sin(q6))/16 + (3^(1/2)*dq2*dqr5*cos(q5)*cos(q6)*sin(q4)*sin(q5)*sin(q6))/2 - (3^(1/2)*dq3*dqr5*cos(q5)*cos(q6)*sin(q4)*sin(q5)*sin(q6))/2 + (5*3^(1/2)*dq1*dqr5*cos(q2)*cos(q5)*cos(q6)^2*sin(q3)*sin(q4)*sin(q5))/16 - (5*3^(1/2)*dq1*dqr5*cos(q3)*cos(q5)*cos(q6)^2*sin(q2)*sin(q4)*sin(q5))/16 + (3^(1/2)*dq1*dqr5*cos(q2)*cos(q5)^2*cos(q6)*sin(q3)*sin(q4)*sin(q6))/4 - (3^(1/2)*dq1*dqr5*cos(q3)*cos(q5)^2*cos(q6)*sin(q2)*sin(q4)*sin(q6))/4 + (3^(1/2)*dq1*dqr6*cos(q2)*cos(q5)*cos(q6)^2*sin(q3)*sin(q4)*sin(q5))/4 - (3^(1/2)*dq1*dqr6*cos(q3)*cos(q5)*cos(q6)^2*sin(q2)*sin(q4)*sin(q5))/4 + (5*3^(1/2)*dq1*dqr6*cos(q2)*cos(q5)^2*cos(q6)*sin(q3)*sin(q4)*sin(q6))/16 - (5*3^(1/2)*dq1*dqr6*cos(q3)*cos(q5)^2*cos(q6)*sin(q2)*sin(q4)*sin(q6))/16 + (3*3^(1/2)*dq1*dqr5*cos(q2)*cos(q5)*cos(q6)*sin(q3)*sin(q4)*sin(q6))/8 - (3*3^(1/2)*dq1*dqr5*cos(q3)*cos(q5)*cos(q6)*sin(q2)*sin(q4)*sin(q6))/8 - (3^(1/2)*dq1*dqr6*cos(q2)*cos(q4)*cos(q6)*sin(q3)*sin(q5)*sin(q6))/8 + (3^(1/2)*dq1*dqr6*cos(q2)*cos(q5)*cos(q6)*sin(q3)*sin(q4)*sin(q6))/8 + (3^(1/2)*dq1*dqr6*cos(q3)*cos(q4)*cos(q6)*sin(q2)*sin(q5)*sin(q6))/8 - (3^(1/2)*dq1*dqr6*cos(q3)*cos(q5)*cos(q6)*sin(q2)*sin(q4)*sin(q6))/8 + (3^(1/2)*dq1*dqr5*cos(q2)*cos(q4)*cos(q5)*cos(q6)*sin(q3)*sin(q5)*sin(q6))/2 - (3^(1/2)*dq1*dqr5*cos(q3)*cos(q4)*cos(q5)*cos(q6)*sin(q2)*sin(q5)*sin(q6))/2 + (5*3^(1/2)*dq1*dqr6*cos(q2)*cos(q4)*cos(q5)*cos(q6)*sin(q3)*sin(q5)*sin(q6))/8 - (5*3^(1/2)*dq1*dqr6*cos(q3)*cos(q4)*cos(q5)*cos(q6)*sin(q2)*sin(q5)*sin(q6))/8;
Y4_20_8=(3*dq4*dqr6*sin(q5))/8 - (3*dq4*dqr6*sin(2*q5))/16 - (9*dq4*dqr6*sin(2*q6))/32 + (3*dq5*dqr6*sin(2*q6))/16 + (ddqr1*sin(q2)*sin(q3))/4 - (3*dq4*dqr6*cos(q6)^2*sin(q5))/4 - (3*dq5*dqr6*cos(q6)^2*sin(q5))/4 - (3*ddqr4*cos(q6)*sin(q5)*sin(q6))/4 - (3*ddqr5*cos(q6)*sin(q5)*sin(q6))/4 + (3*ddqr1*cos(q5)^2*sin(q2)*sin(q3))/4 + (9*ddqr1*cos(q6)^2*sin(q2)*sin(q3))/16 + (3*dq4*dqr6*cos(q5)*cos(q6)^2*sin(q5))/4 + (15*dq4*dqr6*cos(q5)^2*cos(q6)*sin(q6))/16 + (3^(1/2)*ddqr2*cos(q6)^2*sin(q4)*sin(q5))/8 - (3^(1/2)*ddqr3*cos(q6)^2*sin(q4)*sin(q5))/8 + (3*ddqr4*cos(q5)*cos(q6)*sin(q5)*sin(q6))/4 - (3^(1/2)*dq2*dqr6*cos(q4)*sin(q5))/8 - (3^(1/2)*dq2*dqr6*cos(q5)*sin(q4))/4 + (3^(1/2)*dq3*dqr6*cos(q4)*sin(q5))/8 + (3^(1/2)*dq3*dqr6*cos(q5)*sin(q4))/4 + (3*ddqr1*cos(q5)*cos(q6)^2*sin(q2)*sin(q3))/8 + (3^(1/2)*dq2*dqr6*cos(q5)^2*sin(q4))/4 + (3^(1/2)*dq2*dqr6*cos(q6)^2*sin(q4))/4 - (3^(1/2)*dq3*dqr6*cos(q5)^2*sin(q4))/4 - (3^(1/2)*dq3*dqr6*cos(q6)^2*sin(q4))/4 + (3*dq1*dqr6*cos(q2)*cos(q3)*sin(q5))/8 - (3*dq4*dqr6*cos(q5)*cos(q6)*sin(q6))/8 - (3*dq5*dqr6*cos(q5)*cos(q6)*sin(q6))/8 - (3^(1/2)*ddqr1*cos(q2)*sin(q3)*sin(q4))/4 + (3^(1/2)*ddqr1*cos(q3)*sin(q2)*sin(q4))/4 + (3^(1/2)*ddqr2*cos(q5)*sin(q4)*sin(q5))/2 - (3^(1/2)*ddqr3*cos(q5)*sin(q4)*sin(q5))/2 + (3^(1/2)*ddqr2*cos(q6)*sin(q4)*sin(q6))/4 - (3^(1/2)*ddqr3*cos(q6)*sin(q4)*sin(q6))/4 - (15*ddqr1*cos(q5)^2*cos(q6)^2*sin(q2)*sin(q3))/16 - (3*ddqr1*cos(q2)*cos(q3)*cos(q6)*sin(q5)*sin(q6))/4 + (3^(1/2)*dq2*dqr6*cos(q4)*cos(q5)*sin(q5))/8 - (3^(1/2)*dq3*dqr6*cos(q4)*cos(q5)*sin(q5))/8 + (7*3^(1/2)*dq2*dqr6*cos(q4)*cos(q6)*sin(q6))/16 - (7*3^(1/2)*dq3*dqr6*cos(q4)*cos(q6)*sin(q6))/16 - (3*ddqr1*cos(q6)*sin(q2)*sin(q3)*sin(q5)*sin(q6))/4 - (3^(1/2)*dq2*dqr6*cos(q4)*cos(q6)^2*sin(q5))/4 + (3^(1/2)*dq2*dqr6*cos(q5)*cos(q6)^2*sin(q4))/4 + (3^(1/2)*dq3*dqr6*cos(q4)*cos(q6)^2*sin(q5))/4 - (3^(1/2)*dq3*dqr6*cos(q5)*cos(q6)^2*sin(q4))/4 - (3*dq1*dqr6*cos(q2)*cos(q3)*cos(q5)*sin(q5))/8 - (9*dq1*dqr6*cos(q2)*cos(q3)*cos(q6)*sin(q6))/16 - (3^(1/2)*ddqr2*cos(q4)*cos(q6)*sin(q5)*sin(q6))/4 + (3^(1/2)*ddqr2*cos(q5)*cos(q6)*sin(q4)*sin(q6))/4 + (3^(1/2)*ddqr3*cos(q4)*cos(q6)*sin(q5)*sin(q6))/4 - (3^(1/2)*ddqr3*cos(q5)*cos(q6)*sin(q4)*sin(q6))/4 - (3^(1/2)*dq2*dqr6*cos(q5)^2*cos(q6)^2*sin(q4))/2 + (3^(1/2)*dq3*dqr6*cos(q5)^2*cos(q6)^2*sin(q4))/2 - (3*dq1*dqr6*cos(q2)*cos(q3)*cos(q6)^2*sin(q5))/4 + (3^(1/2)*ddqr1*cos(q2)*cos(q5)^2*sin(q3)*sin(q4))/4 - (3^(1/2)*ddqr1*cos(q3)*cos(q5)^2*sin(q2)*sin(q4))/4 + (7*3^(1/2)*ddqr1*cos(q2)*cos(q6)^2*sin(q3)*sin(q4))/16 - (7*3^(1/2)*ddqr1*cos(q3)*cos(q6)^2*sin(q2)*sin(q4))/16 - (5*3^(1/2)*ddqr2*cos(q5)*cos(q6)^2*sin(q4)*sin(q5))/8 - (3^(1/2)*ddqr2*cos(q5)^2*cos(q6)*sin(q4)*sin(q6))/2 + (5*3^(1/2)*ddqr3*cos(q5)*cos(q6)^2*sin(q4)*sin(q5))/8 + (3^(1/2)*ddqr3*cos(q5)^2*cos(q6)*sin(q4)*sin(q6))/2 - (3^(1/2)*dq2*dqr6*cos(q6)*sin(q4)*sin(q5)*sin(q6))/8 + (3^(1/2)*dq3*dqr6*cos(q6)*sin(q4)*sin(q5)*sin(q6))/8 - (5*3^(1/2)*ddqr1*cos(q2)*cos(q5)^2*cos(q6)^2*sin(q3)*sin(q4))/16 + (5*3^(1/2)*ddqr1*cos(q3)*cos(q5)^2*cos(q6)^2*sin(q2)*sin(q4))/16 + (3^(1/2)*dq1*dqr6*cos(q2)*cos(q4)*cos(q6)^2*sin(q3))/4 - (3^(1/2)*dq2*dqr6*cos(q4)*cos(q5)*cos(q6)^2*sin(q5))/4 - (5*3^(1/2)*dq2*dqr6*cos(q4)*cos(q5)^2*cos(q6)*sin(q6))/16 + (3^(1/2)*dq3*dqr6*cos(q4)*cos(q5)*cos(q6)^2*sin(q5))/4 + (5*3^(1/2)*dq3*dqr6*cos(q4)*cos(q5)^2*cos(q6)*sin(q6))/16 - (3*dq1*dqr6*cos(q2)*cos(q3)*cos(q5)*cos(q6)*sin(q6))/8 + (3^(1/2)*ddqr1*cos(q2)*cos(q4)*cos(q5)*sin(q3)*sin(q5))/2 - (3^(1/2)*ddqr1*cos(q3)*cos(q4)*cos(q5)*sin(q2)*sin(q5))/2 + (3^(1/2)*ddqr1*cos(q2)*cos(q4)*cos(q6)*sin(q3)*sin(q6))/4 - (3^(1/2)*ddqr1*cos(q3)*cos(q4)*cos(q6)*sin(q2)*sin(q6))/4 - (3^(1/2)*ddqr2*cos(q4)*cos(q5)*cos(q6)*sin(q5)*sin(q6))/4 + (3^(1/2)*ddqr3*cos(q4)*cos(q5)*cos(q6)*sin(q5)*sin(q6))/4 + (3*dq1*dqr6*cos(q2)*cos(q3)*cos(q5)*cos(q6)^2*sin(q5))/4 + (15*dq1*dqr6*cos(q2)*cos(q3)*cos(q5)^2*cos(q6)*sin(q6))/16 + (3^(1/2)*ddqr1*cos(q2)*cos(q4)*cos(q6)^2*sin(q3)*sin(q5))/8 - (3^(1/2)*ddqr1*cos(q2)*cos(q5)*cos(q6)^2*sin(q3)*sin(q4))/8 - (3^(1/2)*ddqr1*cos(q3)*cos(q4)*cos(q6)^2*sin(q2)*sin(q5))/8 + (3^(1/2)*ddqr1*cos(q3)*cos(q5)*cos(q6)^2*sin(q2)*sin(q4))/8 + (3*ddqr1*cos(q2)*cos(q3)*cos(q5)*cos(q6)*sin(q5)*sin(q6))/4 - (3^(1/2)*dq2*dqr6*cos(q4)*cos(q5)*cos(q6)*sin(q6))/8 + (3^(1/2)*dq3*dqr6*cos(q4)*cos(q5)*cos(q6)*sin(q6))/8 + (3*ddqr1*cos(q5)*cos(q6)*sin(q2)*sin(q3)*sin(q5)*sin(q6))/4 + (3^(1/2)*ddqr1*cos(q2)*cos(q4)*cos(q5)*cos(q6)*sin(q3)*sin(q6))/4 - (3^(1/2)*ddqr1*cos(q3)*cos(q4)*cos(q5)*cos(q6)*sin(q2)*sin(q6))/4 + (3^(1/2)*ddqr1*cos(q2)*cos(q6)*sin(q3)*sin(q4)*sin(q5)*sin(q6))/4 - (3^(1/2)*ddqr1*cos(q3)*cos(q6)*sin(q2)*sin(q4)*sin(q5)*sin(q6))/4 - (5*3^(1/2)*ddqr1*cos(q2)*cos(q4)*cos(q5)*cos(q6)^2*sin(q3)*sin(q5))/8 + (5*3^(1/2)*ddqr1*cos(q3)*cos(q4)*cos(q5)*cos(q6)^2*sin(q2)*sin(q5))/8 - (3^(1/2)*ddqr1*cos(q2)*cos(q4)*cos(q5)^2*cos(q6)*sin(q3)*sin(q6))/2 + (3^(1/2)*ddqr1*cos(q3)*cos(q4)*cos(q5)^2*cos(q6)*sin(q2)*sin(q6))/2 + (5*3^(1/2)*dq2*dqr6*cos(q5)*cos(q6)*sin(q4)*sin(q5)*sin(q6))/8 - (5*3^(1/2)*dq3*dqr6*cos(q5)*cos(q6)*sin(q4)*sin(q5)*sin(q6))/8 + (3^(1/2)*ddqr1*cos(q2)*cos(q5)*cos(q6)*sin(q3)*sin(q4)*sin(q5)*sin(q6))/4 - (3^(1/2)*ddqr1*cos(q3)*cos(q5)*cos(q6)*sin(q2)*sin(q4)*sin(q5)*sin(q6))/4;
Y4_20_9=ddqr4/4 + ddqr5/2 + ddqr6/4 + (3*ddqr6*cos(q5))/4 + (3*ddqr4*cos(q5)^2)/4 + (9*ddqr4*cos(q6)^2)/16 - (3*ddqr5*cos(q6)^2)/8 - (15*ddqr4*cos(q5)^2*cos(q6)^2)/16 + (ddqr1*cos(q2)*cos(q3))/4 + (3*ddqr4*cos(q5)*cos(q6)^2)/8 + (3*ddqr5*cos(q5)*cos(q6)^2)/8 + (3^(1/2)*ddqr2*cos(q4))/4 - (3^(1/2)*ddqr3*cos(q4))/4 - (3^(1/2)*ddqr2*cos(q4)*cos(q5)^2)/4 - (7*3^(1/2)*ddqr2*cos(q4)*cos(q6)^2)/16 + (3^(1/2)*ddqr3*cos(q4)*cos(q5)^2)/4 + (7*3^(1/2)*ddqr3*cos(q4)*cos(q6)^2)/16 + (3*ddqr1*cos(q2)*cos(q3)*cos(q5)^2)/4 + (9*ddqr1*cos(q2)*cos(q3)*cos(q6)^2)/16 + (3^(1/2)*ddqr2*cos(q4)*cos(q5)*cos(q6)^2)/8 - (3^(1/2)*ddqr3*cos(q4)*cos(q5)*cos(q6)^2)/8 + (5*3^(1/2)*ddqr2*cos(q4)*cos(q5)^2*cos(q6)^2)/16 - (5*3^(1/2)*ddqr3*cos(q4)*cos(q5)^2*cos(q6)^2)/16 + (3*ddqr1*cos(q2)*cos(q3)*cos(q5)*cos(q6)^2)/8 - (15*ddqr1*cos(q2)*cos(q3)*cos(q5)^2*cos(q6)^2)/16;
Y4_23_1=-sin(q2 - q3)*cos(q4);
Y4_24_1=(sin(q2 - q3)*cos(q4)*cos(q5))/2 - sin(q2 - q3)*sin(q4)*sin(q5);
Y4_25_1=(sin(q2 - q3)*cos(q4)*sin(q5)*sin(q6))/2 - (3*sin(q2 - q3)*cos(q4)*cos(q6))/4 + sin(q2 - q3)*cos(q5)*sin(q4)*sin(q6) + (sin(q2 - q3)*cos(q6)*sin(q4)*sin(q5))/2 - (sin(q2 - q3)*cos(q4)*cos(q5)*cos(q6))/4;
Y5_5_1=(259*dq1*dqr1*cos(q5)*sin(q4))/1000000 - (1369*dq1*dqr1*cos(q2)^2*cos(q4)*sin(q4))/2000000 + (1369*dq2*dqr1*cos(q2)*cos(q4)^2*sin(q3))/2000000 - (1369*dq2*dqr1*cos(q3)*cos(q4)^2*sin(q2))/2000000 - (1369*dq1*dqr1*cos(q3)^2*cos(q4)*sin(q4))/2000000 + (1369*dq2*dqr1*cos(q2)*cos(q5)^2*sin(q3))/2000000 - (1369*dq2*dqr1*cos(q3)*cos(q5)^2*sin(q2))/2000000 - (1369*dq3*dqr1*cos(q2)*cos(q4)^2*sin(q3))/2000000 + (1369*dq3*dqr1*cos(q3)*cos(q4)^2*sin(q2))/2000000 - (1369*dq3*dqr1*cos(q2)*cos(q5)^2*sin(q3))/2000000 + (1369*dq3*dqr1*cos(q3)*cos(q5)^2*sin(q2))/2000000 + (1073*dq1*dqr1*cos(q4)*cos(q5)*sin(q3))/100000 - (1073*dq2*dqr1*cos(q2)*cos(q5)*sin(q4))/100000 - (1073*dq1*dqr1*sin(q3)*sin(q4)*sin(q5))/200000 + (1073*dq1*dqr1*cos(q2)^2*sin(q3)*sin(q4)*sin(q5))/200000 - (1369*3^(1/2)*dq1*dqr1*cos(q2)*cos(q4)*sin(q2))/2000000 + (1369*3^(1/2)*dq1*dqr1*cos(q3)*cos(q4)*sin(q3))/2000000 - (1369*3^(1/2)*dq4*dqr1*cos(q2)*cos(q4)*sin(q3))/2000000 + (1369*3^(1/2)*dq4*dqr1*cos(q3)*cos(q4)*sin(q2))/2000000 + (1369*dq1*dqr1*cos(q2)^2*cos(q3)^2*cos(q4)*sin(q4))/1000000 + (1369*dq1*dqr1*cos(q2)^2*cos(q4)*cos(q5)^2*sin(q4))/1000000 - (1369*dq1*dqr1*cos(q2)^2*cos(q3)^2*cos(q5)*sin(q5))/1000000 - (1369*dq2*dqr1*cos(q2)*cos(q4)^2*cos(q5)^2*sin(q3))/1000000 + (1369*dq2*dqr1*cos(q3)*cos(q4)^2*cos(q5)^2*sin(q2))/1000000 + (1369*dq1*dqr1*cos(q3)^2*cos(q4)*cos(q5)^2*sin(q4))/1000000 + (1369*dq3*dqr1*cos(q2)*cos(q4)^2*cos(q5)^2*sin(q3))/1000000 - (1369*dq3*dqr1*cos(q3)*cos(q4)^2*cos(q5)^2*sin(q2))/1000000 + (1073*3^(1/2)*dq1*dqr1*cos(q2)^2*cos(q3)*sin(q5))/200000 + (32449*dq1*dqr1*cos(q2)*cos(q4)*cos(q5)*sin(q2))/4000000 - (32449*dq1*dqr1*cos(q3)*cos(q4)*cos(q5)*sin(q3))/4000000 + (32449*dq2*dqr1*cos(q2)*cos(q3)*cos(q5)*sin(q4))/4000000 - (32449*dq3*dqr1*cos(q2)*cos(q3)*cos(q5)*sin(q4))/4000000 - dq1*dqr1*cos(q2)^2*cos(q3)^2*sin(q5)*((92981*3^(1/2))/10000000 + 1369/1000000) + (32449*dq2*dqr1*cos(q4)*sin(q2)*sin(q3)*sin(q5))/8000000 + (32449*dq2*dqr1*cos(q5)*sin(q2)*sin(q3)*sin(q4))/4000000 - (32449*dq3*dqr1*cos(q4)*sin(q2)*sin(q3)*sin(q5))/8000000 - (32449*dq3*dqr1*cos(q5)*sin(q2)*sin(q3)*sin(q4))/4000000 - (4107*dq4*dqr1*cos(q5)*sin(q2)*sin(q3)*sin(q5))/4000000 - dq2*dqr1*cos(q2)*cos(q5)*sin(q3)*((23717*3^(1/2))/20000000 + 1369/1000000) + dq2*dqr1*cos(q3)*cos(q5)*sin(q2)*((23717*3^(1/2))/20000000 + 1369/1000000) + dq3*dqr1*cos(q2)*cos(q5)*sin(q3)*((23717*3^(1/2))/20000000 + 1369/1000000) - dq3*dqr1*cos(q3)*cos(q5)*sin(q2)*((23717*3^(1/2))/20000000 + 1369/1000000) - (1073*dq1*dqr1*cos(q2)^2*cos(q4)*cos(q5)*sin(q3))/100000 - dq4*dqr1*sin(q2)*sin(q3)*sin(q5)*((23717*3^(1/2))/40000000 + 1369/2000000) - dq1*dqr1*cos(q2)^2*cos(q4)*cos(q5)*sin(q4)*((23717*3^(1/2))/20000000 + 1369/1000000) + dq2*dqr1*cos(q2)*cos(q4)^2*cos(q5)*sin(q3)*((23717*3^(1/2))/20000000 + 1369/1000000) - dq2*dqr1*cos(q3)*cos(q4)^2*cos(q5)*sin(q2)*((23717*3^(1/2))/20000000 + 1369/1000000) - dq1*dqr1*cos(q3)^2*cos(q4)*cos(q5)*sin(q4)*((23717*3^(1/2))/20000000 + 1369/1000000) - dq3*dqr1*cos(q2)*cos(q4)^2*cos(q5)*sin(q3)*((23717*3^(1/2))/20000000 + 1369/1000000) + dq3*dqr1*cos(q3)*cos(q4)^2*cos(q5)*sin(q2)*((23717*3^(1/2))/20000000 + 1369/1000000) + (1073*3^(1/2)*dq1*dqr1*cos(q2)*sin(q2)*sin(q3)*sin(q5))/200000 + (1369*3^(1/2)*dq1*dqr1*cos(q2)*cos(q3)^2*cos(q4)*sin(q2))/1000000 - (1369*3^(1/2)*dq1*dqr1*cos(q2)^2*cos(q3)*cos(q4)*sin(q3))/1000000 + (1369*3^(1/2)*dq1*dqr1*cos(q2)*cos(q4)*cos(q5)^2*sin(q2))/1000000 - (1369*3^(1/2)*dq1*dqr1*cos(q3)*cos(q4)*cos(q5)^2*sin(q3))/1000000 + (1369*3^(1/2)*dq2*dqr1*cos(q2)*cos(q3)*cos(q5)^2*sin(q4))/2000000 - (1369*3^(1/2)*dq3*dqr1*cos(q2)*cos(q3)*cos(q5)^2*sin(q4))/2000000 + (1369*3^(1/2)*dq4*dqr1*cos(q2)*cos(q4)*cos(q5)^2*sin(q3))/2000000 - (1369*3^(1/2)*dq4*dqr1*cos(q3)*cos(q4)*cos(q5)^2*sin(q2))/2000000 + (1073*dq1*dqr1*cos(q2)*cos(q3)*cos(q4)*cos(q5)*sin(q2))/100000 + (1369*3^(1/2)*dq2*dqr1*cos(q5)^2*sin(q2)*sin(q3)*sin(q4))/2000000 - (1369*3^(1/2)*dq3*dqr1*cos(q5)^2*sin(q2)*sin(q3)*sin(q4))/2000000 - (1369*dq1*dqr1*cos(q2)^2*cos(q3)^2*cos(q4)*cos(q5)^2*sin(q4))/500000 - (1369*dq1*dqr1*cos(q2)^2*cos(q3)^2*cos(q4)^2*cos(q5)*sin(q5))/400000 - (1073*dq1*dqr1*cos(q2)*cos(q3)*sin(q2)*sin(q4)*sin(q5))/200000 - (32449*dq1*dqr1*cos(q2)*cos(q3)^2*cos(q4)*cos(q5)*sin(q2))/2000000 + (32449*dq1*dqr1*cos(q2)^2*cos(q3)*cos(q4)*cos(q5)*sin(q3))/2000000 + dq1*dqr1*cos(q2)^2*cos(q3)^2*cos(q4)^2*sin(q5)*((23717*3^(1/2))/20000000 + 1369/1000000) + dq1*dqr1*cos(q2)*sin(q2)*sin(q4)*sin(q5)*((1369*3^(1/2))/2000000 - 45547/20000000) - dq1*dqr1*cos(q3)*sin(q3)*sin(q4)*sin(q5)*((1369*3^(1/2))/2000000 - 45547/20000000) + dq4*dqr1*cos(q2)*sin(q3)*sin(q4)*sin(q5)*((1369*3^(1/2))/2000000 + 71151/40000000) - dq4*dqr1*cos(q3)*sin(q2)*sin(q4)*sin(q5)*((1369*3^(1/2))/2000000 + 71151/40000000) + dq1*dqr1*cos(q2)^2*cos(q3)^2*cos(q4)*cos(q5)*sin(q4)*((23717*3^(1/2))/10000000 + 1369/500000) + (1369*dq1*dqr1*cos(q2)*cos(q3)*cos(q4)*sin(q2)*sin(q3)*sin(q4))/1000000 - (1369*dq1*dqr1*cos(q2)*cos(q3)*cos(q5)*sin(q2)*sin(q3)*sin(q5))/1000000 + (1369*dq2*dqr1*cos(q2)*cos(q4)*cos(q5)*sin(q3)*sin(q4)*sin(q5))/800000 - (1369*dq2*dqr1*cos(q3)*cos(q4)*cos(q5)*sin(q2)*sin(q4)*sin(q5))/800000 - (1369*dq3*dqr1*cos(q2)*cos(q4)*cos(q5)*sin(q3)*sin(q4)*sin(q5))/800000 + (1369*dq3*dqr1*cos(q3)*cos(q4)*cos(q5)*sin(q2)*sin(q4)*sin(q5))/800000 - (1369*3^(1/2)*dq1*dqr1*cos(q2)*cos(q3)^2*cos(q4)*cos(q5)^2*sin(q2))/500000 + (1369*3^(1/2)*dq1*dqr1*cos(q2)^2*cos(q3)*cos(q4)*cos(q5)^2*sin(q3))/500000 - dq1*dqr1*cos(q2)*cos(q3)*sin(q2)*sin(q3)*sin(q5)*((92981*3^(1/2))/10000000 + 1369/1000000) - dq2*dqr1*cos(q2)*cos(q4)*sin(q3)*sin(q4)*sin(q5)*((23717*3^(1/2))/40000000 + 1369/2000000) + dq2*dqr1*cos(q3)*cos(q4)*sin(q2)*sin(q4)*sin(q5)*((23717*3^(1/2))/40000000 + 1369/2000000) + dq3*dqr1*cos(q2)*cos(q4)*sin(q3)*sin(q4)*sin(q5)*((23717*3^(1/2))/40000000 + 1369/2000000) - dq3*dqr1*cos(q3)*cos(q4)*sin(q2)*sin(q4)*sin(q5)*((23717*3^(1/2))/40000000 + 1369/2000000) - (1369*3^(1/2)*dq1*dqr1*cos(q2)*cos(q5)*sin(q2)*sin(q4)*sin(q5))/2000000 + (1369*3^(1/2)*dq1*dqr1*cos(q3)*cos(q5)*sin(q3)*sin(q4)*sin(q5))/2000000 + (1369*3^(1/2)*dq2*dqr1*cos(q4)*cos(q5)*sin(q2)*sin(q3)*sin(q5))/4000000 - (1369*3^(1/2)*dq3*dqr1*cos(q4)*cos(q5)*sin(q2)*sin(q3)*sin(q5))/4000000 - (1369*3^(1/2)*dq4*dqr1*cos(q2)*cos(q5)*sin(q3)*sin(q4)*sin(q5))/4000000 + (1369*3^(1/2)*dq4*dqr1*cos(q3)*cos(q5)*sin(q2)*sin(q4)*sin(q5))/4000000 - dq1*dqr1*cos(q2)*cos(q3)^2*sin(q2)*sin(q4)*sin(q5)*((1369*3^(1/2))/1000000 - 45547/10000000) + dq1*dqr1*cos(q2)^2*cos(q3)*sin(q3)*sin(q4)*sin(q5)*((1369*3^(1/2))/1000000 - 45547/10000000) + (1369*3^(1/2)*dq1*dqr1*cos(q2)*cos(q3)^2*cos(q5)*sin(q2)*sin(q4)*sin(q5))/1000000 - (1369*3^(1/2)*dq1*dqr1*cos(q2)^2*cos(q3)*cos(q5)*sin(q3)*sin(q4)*sin(q5))/1000000 - (1369*dq1*dqr1*cos(q2)*cos(q3)*cos(q4)*cos(q5)^2*sin(q2)*sin(q3)*sin(q4))/500000 - (1369*dq1*dqr1*cos(q2)*cos(q3)*cos(q4)^2*cos(q5)*sin(q2)*sin(q3)*sin(q5))/400000 + dq1*dqr1*cos(q2)*cos(q3)*cos(q4)^2*sin(q2)*sin(q3)*sin(q5)*((23717*3^(1/2))/20000000 + 1369/1000000) + dq1*dqr1*cos(q2)*cos(q3)*cos(q4)*cos(q5)*sin(q2)*sin(q3)*sin(q4)*((23717*3^(1/2))/10000000 + 1369/500000);
Y5_5_2=(1369*dq2*dqr2*sin(2*q4))/4000000 - (4107*dq1*dqr1*sin(2*q5))/8000000 + (1369*dq2*dqr2*sin(2*q5))/2000000 - (1369*dq3*dqr2*sin(2*q4))/4000000 - (1369*dq3*dqr2*sin(2*q5))/2000000 + dq2*dqr2*sin(q5)*((4329*3^(1/2))/1250000 - 1369/2000000) - dq2*dqr3*sin(q5)*((4329*3^(1/2))/1250000 - 1369/2000000) - dq3*dqr2*sin(q5)*((4329*3^(1/2))/1250000 - 1369/2000000) + dq3*dqr3*sin(q5)*((4329*3^(1/2))/1250000 - 1369/2000000) - dq1*dqr1*sin(q5)*((23717*3^(1/2))/40000000 + 1369/2000000) - (1369*3^(1/2)*dq4*dqr2*sin(q4))/2000000 + (1369*3^(1/2)*dq4*dqr3*sin(q4))/2000000 + (259*dq1*dqr1*cos(q4)*sin(q5))/2000000 - dq4*dqr2*cos(q4)*sin(q5)*((1369*3^(1/2))/2000000 + 71151/40000000) + dq4*dqr3*cos(q4)*sin(q5)*((1369*3^(1/2))/2000000 + 71151/40000000) + (1369*dq1*dqr2*cos(q2)*cos(q4)^2*sin(q3))/2000000 - (1369*dq1*dqr2*cos(q3)*cos(q4)^2*sin(q2))/2000000 + (1369*dq1*dqr2*cos(q2)*cos(q5)^2*sin(q3))/2000000 - (1369*dq1*dqr2*cos(q3)*cos(q5)^2*sin(q2))/2000000 - (1369*dq1*dqr3*cos(q2)*cos(q4)^2*sin(q3))/2000000 + (1369*dq1*dqr3*cos(q3)*cos(q4)^2*sin(q2))/2000000 + (1369*dq1*dqr1*cos(q2)^2*cos(q5)*sin(q5))/2000000 - (1369*dq1*dqr3*cos(q2)*cos(q5)^2*sin(q3))/2000000 + (1369*dq1*dqr3*cos(q3)*cos(q5)^2*sin(q2))/2000000 + (1369*dq1*dqr1*cos(q3)^2*cos(q5)*sin(q5))/2000000 - (1369*dq2*dqr2*cos(q4)*cos(q5)^2*sin(q4))/1000000 - (1369*dq2*dqr2*cos(q4)^2*cos(q5)*sin(q5))/800000 + (1369*dq2*dqr3*cos(q4)*cos(q5)^2*sin(q4))/1000000 + (1369*dq3*dqr2*cos(q4)*cos(q5)^2*sin(q4))/1000000 + (1369*dq2*dqr3*cos(q4)^2*cos(q5)*sin(q5))/800000 + (1369*dq3*dqr2*cos(q4)^2*cos(q5)*sin(q5))/800000 - (1369*dq3*dqr3*cos(q4)*cos(q5)^2*sin(q4))/1000000 - (1369*dq3*dqr3*cos(q4)^2*cos(q5)*sin(q5))/800000 - (1073*3^(1/2)*dq1*dqr1*cos(q3)*sin(q5))/200000 - (1073*3^(1/2)*dq2*dqr2*cos(q3)*sin(q5))/200000 + dq1*dqr1*cos(q2)^2*sin(q5)*((92981*3^(1/2))/20000000 + 1369/2000000) + dq1*dqr1*cos(q3)^2*sin(q5)*((92981*3^(1/2))/20000000 + 1369/2000000) + dq2*dqr2*cos(q4)^2*sin(q5)*((23717*3^(1/2))/40000000 + 1369/2000000) - dq2*dqr3*cos(q4)^2*sin(q5)*((23717*3^(1/2))/40000000 + 1369/2000000) - dq3*dqr2*cos(q4)^2*sin(q5)*((23717*3^(1/2))/40000000 + 1369/2000000) + dq3*dqr3*cos(q4)^2*sin(q5)*((23717*3^(1/2))/40000000 + 1369/2000000) + (1369*3^(1/2)*dq4*dqr2*cos(q5)^2*sin(q4))/2000000 - (1369*3^(1/2)*dq4*dqr3*cos(q5)^2*sin(q4))/2000000 - (1073*dq1*dqr2*cos(q2)*cos(q4)*sin(q5))/200000 - (1073*dq1*dqr2*cos(q2)*cos(q5)*sin(q4))/100000 - (1073*dq2*dqr1*cos(q2)*cos(q4)*sin(q5))/200000 + (1073*dq2*dqr2*cos(q4)*cos(q5)*sin(q3))/100000 - (1073*dq2*dqr2*sin(q3)*sin(q4)*sin(q5))/200000 + (1369*3^(1/2)*dq4*dqr2*cos(q4)*cos(q5)*sin(q5))/4000000 - (1369*3^(1/2)*dq4*dqr3*cos(q4)*cos(q5)*sin(q5))/4000000 - (1369*dq1*dqr2*cos(q2)*cos(q4)^2*cos(q5)^2*sin(q3))/1000000 + (1369*dq1*dqr2*cos(q3)*cos(q4)^2*cos(q5)^2*sin(q2))/1000000 + (1369*dq1*dqr1*cos(q2)^2*cos(q4)^2*cos(q5)*sin(q5))/800000 + (1369*dq1*dqr3*cos(q2)*cos(q4)^2*cos(q5)^2*sin(q3))/1000000 - (1369*dq1*dqr3*cos(q3)*cos(q4)^2*cos(q5)^2*sin(q2))/1000000 + (1369*dq1*dqr1*cos(q3)^2*cos(q4)^2*cos(q5)*sin(q5))/800000 + (32449*dq1*dqr2*cos(q2)*cos(q3)*cos(q4)*sin(q5))/8000000 + (32449*dq1*dqr2*cos(q2)*cos(q3)*cos(q5)*sin(q4))/4000000 + (32449*dq2*dqr1*cos(q2)*cos(q3)*cos(q4)*sin(q5))/8000000 - (32449*dq1*dqr3*cos(q2)*cos(q3)*cos(q4)*sin(q5))/8000000 - (32449*dq1*dqr3*cos(q2)*cos(q3)*cos(q5)*sin(q4))/4000000 - (32449*dq3*dqr1*cos(q2)*cos(q3)*cos(q4)*sin(q5))/8000000 - (4107*dq4*dqr1*cos(q2)*cos(q3)*cos(q5)*sin(q5))/4000000 - dq1*dqr1*cos(q2)^2*cos(q4)^2*sin(q5)*((23717*3^(1/2))/40000000 + 1369/2000000) - dq1*dqr1*cos(q3)^2*cos(q4)^2*sin(q5)*((23717*3^(1/2))/40000000 + 1369/2000000) + (32449*dq1*dqr2*cos(q4)*sin(q2)*sin(q3)*sin(q5))/8000000 + (32449*dq1*dqr2*cos(q5)*sin(q2)*sin(q3)*sin(q4))/4000000 - (32449*dq1*dqr3*cos(q4)*sin(q2)*sin(q3)*sin(q5))/8000000 - (32449*dq1*dqr3*cos(q5)*sin(q2)*sin(q3)*sin(q4))/4000000 - dq1*dqr2*cos(q2)*cos(q5)*sin(q3)*((23717*3^(1/2))/20000000 + 1369/1000000) + dq1*dqr2*cos(q3)*cos(q5)*sin(q2)*((23717*3^(1/2))/20000000 + 1369/1000000) + dq1*dqr3*cos(q2)*cos(q5)*sin(q3)*((23717*3^(1/2))/20000000 + 1369/1000000) - dq1*dqr3*cos(q3)*cos(q5)*sin(q2)*((23717*3^(1/2))/20000000 + 1369/1000000) + dq2*dqr2*cos(q4)*cos(q5)*sin(q4)*((23717*3^(1/2))/20000000 + 1369/1000000) - dq2*dqr3*cos(q4)*cos(q5)*sin(q4)*((23717*3^(1/2))/20000000 + 1369/1000000) - dq3*dqr2*cos(q4)*cos(q5)*sin(q4)*((23717*3^(1/2))/20000000 + 1369/1000000) + dq3*dqr3*cos(q4)*cos(q5)*sin(q4)*((23717*3^(1/2))/20000000 + 1369/1000000) - dq4*dqr1*cos(q2)*cos(q3)*sin(q5)*((23717*3^(1/2))/40000000 + 1369/2000000) + dq1*dqr2*cos(q2)*cos(q4)^2*cos(q5)*sin(q3)*((23717*3^(1/2))/20000000 + 1369/1000000) - dq1*dqr2*cos(q3)*cos(q4)^2*cos(q5)*sin(q2)*((23717*3^(1/2))/20000000 + 1369/1000000) - dq1*dqr3*cos(q2)*cos(q4)^2*cos(q5)*sin(q3)*((23717*3^(1/2))/20000000 + 1369/1000000) + dq1*dqr3*cos(q3)*cos(q4)^2*cos(q5)*sin(q2)*((23717*3^(1/2))/20000000 + 1369/1000000) + (1369*3^(1/2)*dq1*dqr2*cos(q2)*cos(q3)*cos(q5)^2*sin(q4))/2000000 - (1369*3^(1/2)*dq1*dqr3*cos(q2)*cos(q3)*cos(q5)^2*sin(q4))/2000000 + (1369*3^(1/2)*dq1*dqr2*cos(q5)^2*sin(q2)*sin(q3)*sin(q4))/2000000 - (1369*3^(1/2)*dq1*dqr3*cos(q5)^2*sin(q2)*sin(q3)*sin(q4))/2000000 + (1369*dq1*dqr2*cos(q2)*cos(q4)*cos(q5)*sin(q3)*sin(q4)*sin(q5))/800000 - (1369*dq1*dqr2*cos(q3)*cos(q4)*cos(q5)*sin(q2)*sin(q4)*sin(q5))/800000 - (1369*dq1*dqr3*cos(q2)*cos(q4)*cos(q5)*sin(q3)*sin(q4)*sin(q5))/800000 + (1369*dq1*dqr3*cos(q3)*cos(q4)*cos(q5)*sin(q2)*sin(q4)*sin(q5))/800000 - dq1*dqr2*cos(q2)*cos(q4)*sin(q3)*sin(q4)*sin(q5)*((23717*3^(1/2))/40000000 + 1369/2000000) + dq1*dqr2*cos(q3)*cos(q4)*sin(q2)*sin(q4)*sin(q5)*((23717*3^(1/2))/40000000 + 1369/2000000) + dq1*dqr3*cos(q2)*cos(q4)*sin(q3)*sin(q4)*sin(q5)*((23717*3^(1/2))/40000000 + 1369/2000000) - dq1*dqr3*cos(q3)*cos(q4)*sin(q2)*sin(q4)*sin(q5)*((23717*3^(1/2))/40000000 + 1369/2000000) + (1369*3^(1/2)*dq1*dqr2*cos(q2)*cos(q3)*cos(q4)*cos(q5)*sin(q5))/4000000 + (1369*3^(1/2)*dq2*dqr1*cos(q2)*cos(q3)*cos(q4)*cos(q5)*sin(q5))/4000000 - (1369*3^(1/2)*dq1*dqr3*cos(q2)*cos(q3)*cos(q4)*cos(q5)*sin(q5))/4000000 - (1369*3^(1/2)*dq3*dqr1*cos(q2)*cos(q3)*cos(q4)*cos(q5)*sin(q5))/4000000 + (1369*3^(1/2)*dq1*dqr2*cos(q4)*cos(q5)*sin(q2)*sin(q3)*sin(q5))/4000000 - (1369*3^(1/2)*dq1*dqr3*cos(q4)*cos(q5)*sin(q2)*sin(q3)*sin(q5))/4000000;
Y5_5_3=(1369*ddqr4)/2000000 + (1369*ddqr5)/1000000 - (1369*dq2*dqr3*sin(2*q4))/4000000 - (1369*dq2*dqr3*sin(2*q5))/2000000 + (1369*dq3*dqr3*sin(2*q4))/4000000 + (1369*dq3*dqr3*sin(2*q5))/2000000 - (4107*dq4*dqr4*sin(2*q5))/8000000 + (1369*ddqr1*cos(q2)*cos(q3))/2000000 + (32449*ddqr2*cos(q4)*cos(q5))/4000000 - (32449*ddqr3*cos(q4)*cos(q5))/4000000 + (1369*ddqr1*sin(q2)*sin(q3))/2000000 - ddqr4*cos(q5)*((23717*3^(1/2))/20000000 + 1369/1000000) + (1369*3^(1/2)*ddqr2*cos(q4))/2000000 - (1369*3^(1/2)*ddqr3*cos(q4))/2000000 - dq4*dqr4*sin(q5)*((23717*3^(1/2))/40000000 + 1369/2000000) - (1073*ddqr2*cos(q3)*cos(q4)*cos(q5))/100000 - (1073*ddqr1*cos(q4)*sin(q2)*sin(q5))/200000 - (1073*ddqr1*cos(q5)*sin(q2)*sin(q4))/100000 + (1073*ddqr2*cos(q3)*sin(q4)*sin(q5))/200000 - (1369*3^(1/2)*dq2*dqr4*sin(q4))/2000000 + (1369*3^(1/2)*dq3*dqr4*sin(q4))/2000000 - ddqr2*sin(q4)*sin(q5)*((1369*3^(1/2))/2000000 + 58349/10000000) + ddqr3*sin(q4)*sin(q5)*((1369*3^(1/2))/2000000 + 58349/10000000) - (1073*3^(1/2)*ddqr2*sin(q3)*sin(q5))/200000 - dq2*dqr4*cos(q4)*sin(q5)*((1369*3^(1/2))/2000000 + 71151/40000000) + dq3*dqr4*cos(q4)*sin(q5)*((1369*3^(1/2))/2000000 + 71151/40000000) + (259*ddqr1*cos(q2)*cos(q3)*cos(q4)*cos(q5))/1000000 - (259*ddqr1*cos(q2)*cos(q3)*sin(q4)*sin(q5))/2000000 - (32449*ddqr1*cos(q2)*cos(q5)*sin(q3)*sin(q4))/4000000 + (32449*ddqr1*cos(q3)*cos(q5)*sin(q2)*sin(q4))/4000000 + (259*ddqr1*cos(q4)*cos(q5)*sin(q2)*sin(q3))/1000000 - (259*ddqr1*sin(q2)*sin(q3)*sin(q4)*sin(q5))/2000000 - ddqr1*cos(q2)*cos(q3)*cos(q5)*((23717*3^(1/2))/20000000 + 1369/1000000) - ddqr1*cos(q5)*sin(q2)*sin(q3)*((23717*3^(1/2))/20000000 + 1369/1000000) + (1369*3^(1/2)*dq2*dqr4*cos(q5)^2*sin(q4))/2000000 - (1369*3^(1/2)*dq3*dqr4*cos(q5)^2*sin(q4))/2000000 - (1369*3^(1/2)*ddqr1*cos(q2)*sin(q3)*sin(q4))/2000000 + (1369*3^(1/2)*ddqr1*cos(q3)*sin(q2)*sin(q4))/2000000 + (259*3^(1/2)*ddqr1*cos(q2)*sin(q3)*sin(q5))/2000000 - (259*3^(1/2)*ddqr1*cos(q3)*sin(q2)*sin(q5))/2000000 - (1369*3^(1/2)*dq1*dqr4*cos(q2)*cos(q4)*sin(q3))/2000000 + (1369*3^(1/2)*dq1*dqr4*cos(q3)*cos(q4)*sin(q2))/2000000 + (1369*3^(1/2)*dq2*dqr4*cos(q4)*cos(q5)*sin(q5))/4000000 - (1369*3^(1/2)*dq3*dqr4*cos(q4)*cos(q5)*sin(q5))/4000000 - ddqr1*cos(q2)*cos(q4)*sin(q3)*sin(q5)*((1369*3^(1/2))/2000000 + 58349/10000000) + ddqr1*cos(q3)*cos(q4)*sin(q2)*sin(q5)*((1369*3^(1/2))/2000000 + 58349/10000000) - (4107*dq1*dqr4*cos(q2)*cos(q3)*cos(q5)*sin(q5))/4000000 - (4107*dq1*dqr4*cos(q5)*sin(q2)*sin(q3)*sin(q5))/4000000 - dq1*dqr4*cos(q2)*cos(q3)*sin(q5)*((23717*3^(1/2))/40000000 + 1369/2000000) - dq1*dqr4*sin(q2)*sin(q3)*sin(q5)*((23717*3^(1/2))/40000000 + 1369/2000000) + (1369*3^(1/2)*dq1*dqr4*cos(q2)*cos(q4)*cos(q5)^2*sin(q3))/2000000 - (1369*3^(1/2)*dq1*dqr4*cos(q3)*cos(q4)*cos(q5)^2*sin(q2))/2000000 + dq1*dqr4*cos(q2)*sin(q3)*sin(q4)*sin(q5)*((1369*3^(1/2))/2000000 + 71151/40000000) - dq1*dqr4*cos(q3)*sin(q2)*sin(q4)*sin(q5)*((1369*3^(1/2))/2000000 + 71151/40000000) - (1369*3^(1/2)*dq1*dqr4*cos(q2)*cos(q5)*sin(q3)*sin(q4)*sin(q5))/4000000 + (1369*3^(1/2)*dq1*dqr4*cos(q3)*cos(q5)*sin(q2)*sin(q4)*sin(q5))/4000000;
Y5_9_1=(37*dq1*dqr1*sin(q5))/2000 - dq2*dqr2*sin(q5)*((117*3^(1/2))/1250 - 37/2000) + dq2*dqr3*sin(q5)*((117*3^(1/2))/1250 - 37/2000) + dq3*dqr2*sin(q5)*((117*3^(1/2))/1250 - 37/2000) - dq3*dqr3*sin(q5)*((117*3^(1/2))/1250 - 37/2000) - (37*dq2*dqr2*cos(q4)^2*sin(q5))/2000 + (37*dq2*dqr3*cos(q4)^2*sin(q5))/2000 + (37*dq3*dqr2*cos(q4)^2*sin(q5))/2000 - (37*dq3*dqr3*cos(q4)^2*sin(q5))/2000 - (7*dq1*dqr1*cos(q4)*sin(q5))/2000 - (7*dq1*dqr1*cos(q5)*sin(q4))/1000 + (29*3^(1/2)*dq1*dqr1*cos(q3)*sin(q5))/200 + (29*3^(1/2)*dq2*dqr2*cos(q3)*sin(q5))/200 + (37*3^(1/2)*dq4*dqr2*cos(q4)*sin(q5))/2000 - (37*3^(1/2)*dq4*dqr3*cos(q4)*sin(q5))/2000 - dq1*dqr1*cos(q2)^2*sin(q5)*((117*3^(1/2))/1250 + 37/2000) - dq1*dqr1*cos(q3)^2*sin(q5)*((117*3^(1/2))/1250 + 37/2000) + (37*dq1*dqr1*cos(q2)^2*cos(q4)^2*sin(q5))/2000 + (37*dq1*dqr1*cos(q3)^2*cos(q4)^2*sin(q5))/2000 + (37*dq1*dqr2*cos(q2)*cos(q5)*sin(q3))/1000 - (37*dq1*dqr2*cos(q3)*cos(q5)*sin(q2))/1000 + (37*dq2*dqr1*cos(q2)*cos(q5)*sin(q3))/1000 - (37*dq2*dqr1*cos(q3)*cos(q5)*sin(q2))/1000 - (29*dq1*dqr1*cos(q4)*cos(q5)*sin(q3))/100 + (29*dq1*dqr2*cos(q2)*cos(q4)*sin(q5))/200 + (29*dq1*dqr2*cos(q2)*cos(q5)*sin(q4))/100 - (37*dq1*dqr3*cos(q2)*cos(q5)*sin(q3))/1000 + (37*dq1*dqr3*cos(q3)*cos(q5)*sin(q2))/1000 + (29*dq2*dqr1*cos(q2)*cos(q4)*sin(q5))/200 + (29*dq2*dqr1*cos(q2)*cos(q5)*sin(q4))/100 - (37*dq3*dqr1*cos(q2)*cos(q5)*sin(q3))/1000 + (37*dq3*dqr1*cos(q3)*cos(q5)*sin(q2))/1000 + (37*dq4*dqr1*cos(q2)*cos(q3)*sin(q5))/2000 - (29*dq2*dqr2*cos(q4)*cos(q5)*sin(q3))/100 - (37*dq2*dqr2*cos(q4)*cos(q5)*sin(q4))/1000 + (37*dq2*dqr3*cos(q4)*cos(q5)*sin(q4))/1000 + (37*dq3*dqr2*cos(q4)*cos(q5)*sin(q4))/1000 - (37*dq3*dqr3*cos(q4)*cos(q5)*sin(q4))/1000 + (29*dq1*dqr1*sin(q3)*sin(q4)*sin(q5))/200 + (37*dq1*dqr4*sin(q2)*sin(q3)*sin(q5))/2000 + (37*dq4*dqr1*sin(q2)*sin(q3)*sin(q5))/2000 + (29*dq2*dqr2*sin(q3)*sin(q4)*sin(q5))/200 - (29*dq1*dqr1*cos(q2)^2*sin(q3)*sin(q4)*sin(q5))/200 - (29*3^(1/2)*dq1*dqr1*cos(q2)^2*cos(q3)*sin(q5))/200 - (117*dq1*dqr1*cos(q2)*cos(q4)*cos(q5)*sin(q2))/625 + (117*dq1*dqr1*cos(q3)*cos(q4)*cos(q5)*sin(q3))/625 - (117*dq1*dqr2*cos(q2)*cos(q3)*cos(q4)*sin(q5))/1250 - (117*dq1*dqr2*cos(q2)*cos(q3)*cos(q5)*sin(q4))/625 - (117*dq2*dqr1*cos(q2)*cos(q3)*cos(q4)*sin(q5))/1250 - (117*dq2*dqr1*cos(q2)*cos(q3)*cos(q5)*sin(q4))/625 + (117*dq1*dqr3*cos(q2)*cos(q3)*cos(q4)*sin(q5))/1250 + (117*dq1*dqr3*cos(q2)*cos(q3)*cos(q5)*sin(q4))/625 + (117*dq3*dqr1*cos(q2)*cos(q3)*cos(q4)*sin(q5))/1250 + (117*dq3*dqr1*cos(q2)*cos(q3)*cos(q5)*sin(q4))/625 + dq1*dqr1*cos(q2)^2*cos(q3)^2*sin(q5)*((117*3^(1/2))/625 + 37/1000) - (37*dq1*dqr1*cos(q2)^2*cos(q3)^2*cos(q4)^2*sin(q5))/1000 - (117*dq1*dqr2*cos(q4)*sin(q2)*sin(q3)*sin(q5))/1250 - (117*dq1*dqr2*cos(q5)*sin(q2)*sin(q3)*sin(q4))/625 - (117*dq2*dqr1*cos(q4)*sin(q2)*sin(q3)*sin(q5))/1250 - (117*dq2*dqr1*cos(q5)*sin(q2)*sin(q3)*sin(q4))/625 + (117*dq1*dqr3*cos(q4)*sin(q2)*sin(q3)*sin(q5))/1250 + (117*dq1*dqr3*cos(q5)*sin(q2)*sin(q3)*sin(q4))/625 + (117*dq3*dqr1*cos(q4)*sin(q2)*sin(q3)*sin(q5))/1250 + (117*dq3*dqr1*cos(q5)*sin(q2)*sin(q3)*sin(q4))/625 + (29*dq1*dqr1*cos(q2)^2*cos(q4)*cos(q5)*sin(q3))/100 + (37*dq1*dqr1*cos(q2)^2*cos(q4)*cos(q5)*sin(q4))/1000 - (37*dq1*dqr2*cos(q2)*cos(q4)^2*cos(q5)*sin(q3))/1000 + (37*dq1*dqr2*cos(q3)*cos(q4)^2*cos(q5)*sin(q2))/1000 - (37*dq2*dqr1*cos(q2)*cos(q4)^2*cos(q5)*sin(q3))/1000 + (37*dq2*dqr1*cos(q3)*cos(q4)^2*cos(q5)*sin(q2))/1000 + (37*dq1*dqr1*cos(q3)^2*cos(q4)*cos(q5)*sin(q4))/1000 + (37*dq1*dqr3*cos(q2)*cos(q4)^2*cos(q5)*sin(q3))/1000 - (37*dq1*dqr3*cos(q3)*cos(q4)^2*cos(q5)*sin(q2))/1000 + (37*dq3*dqr1*cos(q2)*cos(q4)^2*cos(q5)*sin(q3))/1000 - (37*dq3*dqr1*cos(q3)*cos(q4)^2*cos(q5)*sin(q2))/1000 - (29*3^(1/2)*dq1*dqr1*cos(q2)*sin(q2)*sin(q3)*sin(q5))/200 - (37*3^(1/2)*dq1*dqr4*cos(q2)*sin(q3)*sin(q4)*sin(q5))/2000 + (37*3^(1/2)*dq1*dqr4*cos(q3)*sin(q2)*sin(q4)*sin(q5))/2000 - (37*3^(1/2)*dq4*dqr1*cos(q2)*sin(q3)*sin(q4)*sin(q5))/2000 + (37*3^(1/2)*dq4*dqr1*cos(q3)*sin(q2)*sin(q4)*sin(q5))/2000 - (37*dq1*dqr1*cos(q2)^2*cos(q3)^2*cos(q4)*cos(q5)*sin(q4))/500 - (29*dq1*dqr1*cos(q2)*cos(q3)*cos(q4)*cos(q5)*sin(q2))/100 + (29*dq1*dqr1*cos(q2)*cos(q3)*sin(q2)*sin(q4)*sin(q5))/200 + (37*dq1*dqr2*cos(q2)*cos(q4)*sin(q3)*sin(q4)*sin(q5))/2000 - (37*dq1*dqr2*cos(q3)*cos(q4)*sin(q2)*sin(q4)*sin(q5))/2000 + (37*dq2*dqr1*cos(q2)*cos(q4)*sin(q3)*sin(q4)*sin(q5))/2000 - (37*dq2*dqr1*cos(q3)*cos(q4)*sin(q2)*sin(q4)*sin(q5))/2000 - (37*dq1*dqr3*cos(q2)*cos(q4)*sin(q3)*sin(q4)*sin(q5))/2000 + (37*dq1*dqr3*cos(q3)*cos(q4)*sin(q2)*sin(q4)*sin(q5))/2000 - (37*dq3*dqr1*cos(q2)*cos(q4)*sin(q3)*sin(q4)*sin(q5))/2000 + (37*dq3*dqr1*cos(q3)*cos(q4)*sin(q2)*sin(q4)*sin(q5))/2000 + (234*dq1*dqr1*cos(q2)*cos(q3)^2*cos(q4)*cos(q5)*sin(q2))/625 - (234*dq1*dqr1*cos(q2)^2*cos(q3)*cos(q4)*cos(q5)*sin(q3))/625 - dq1*dqr1*cos(q2)*sin(q2)*sin(q4)*sin(q5)*((37*3^(1/2))/2000 - 117/1250) + dq1*dqr1*cos(q3)*sin(q3)*sin(q4)*sin(q5)*((37*3^(1/2))/2000 - 117/1250) + dq1*dqr1*cos(q2)*cos(q3)*sin(q2)*sin(q3)*sin(q5)*((117*3^(1/2))/625 + 37/1000) - (37*dq1*dqr1*cos(q2)*cos(q3)*cos(q4)^2*sin(q2)*sin(q3)*sin(q5))/1000 + dq1*dqr1*cos(q2)*cos(q3)^2*sin(q2)*sin(q4)*sin(q5)*((37*3^(1/2))/1000 - 117/625) - dq1*dqr1*cos(q2)^2*cos(q3)*sin(q3)*sin(q4)*sin(q5)*((37*3^(1/2))/1000 - 117/625) - (37*dq1*dqr1*cos(q2)*cos(q3)*cos(q4)*cos(q5)*sin(q2)*sin(q3)*sin(q4))/500;
Y5_9_2=(37*ddqr4*cos(q5))/1000 + (37*dq4*dqr4*sin(q5))/2000 - (117*ddqr2*cos(q4)*cos(q5))/625 + (117*ddqr3*cos(q4)*cos(q5))/625 + (37*ddqr1*cos(q2)*cos(q3)*cos(q5))/1000 + (29*ddqr2*cos(q3)*cos(q4)*cos(q5))/100 + (37*ddqr1*cos(q5)*sin(q2)*sin(q3))/1000 + (29*ddqr1*cos(q4)*sin(q2)*sin(q5))/200 + (29*ddqr1*cos(q5)*sin(q2)*sin(q4))/100 - (29*ddqr2*cos(q3)*sin(q4)*sin(q5))/200 + ddqr2*sin(q4)*sin(q5)*((37*3^(1/2))/2000 + 117/1250) - ddqr3*sin(q4)*sin(q5)*((37*3^(1/2))/2000 + 117/1250) + (29*3^(1/2)*ddqr2*sin(q3)*sin(q5))/200 - (7*ddqr1*cos(q2)*cos(q3)*cos(q4)*cos(q5))/1000 + (7*ddqr1*cos(q2)*cos(q3)*sin(q4)*sin(q5))/2000 + (117*ddqr1*cos(q2)*cos(q5)*sin(q3)*sin(q4))/625 - (117*ddqr1*cos(q3)*cos(q5)*sin(q2)*sin(q4))/625 - (7*ddqr1*cos(q4)*cos(q5)*sin(q2)*sin(q3))/1000 + (37*3^(1/2)*dq2*dqr4*cos(q4)*sin(q5))/2000 - (37*3^(1/2)*dq3*dqr4*cos(q4)*sin(q5))/2000 + (7*ddqr1*sin(q2)*sin(q3)*sin(q4)*sin(q5))/2000 + (37*dq1*dqr4*cos(q2)*cos(q3)*sin(q5))/2000 - (7*3^(1/2)*ddqr1*cos(q2)*sin(q3)*sin(q5))/2000 + (7*3^(1/2)*ddqr1*cos(q3)*sin(q2)*sin(q5))/2000 + ddqr1*cos(q2)*cos(q4)*sin(q3)*sin(q5)*((37*3^(1/2))/2000 + 117/1250) - ddqr1*cos(q3)*cos(q4)*sin(q2)*sin(q5)*((37*3^(1/2))/2000 + 117/1250);
